simulink library "outp"  (R2021b)
(part 10 of 11)

  UnitConverter67/1 -> VOUTP_LRWhlRotDir_enum/1  "VOUTP_LRWhlRotDir_enum"
  VAPM_LRWhlRotDirTimeOut_flg/1 -> VAPM_LRWhlRotDirTimeOut_flg_Inproc/1  "VAPM_LRWhlRotDirTimeOut_flg"
  VAPM_LRWhlRotDirTimeOut_flg_Inproc/1 -> UnitConverter68/1
  UnitConverter68/1 -> VOUTP_LRWhlRotDirTimeOut_flg/1  "VOUTP_LRWhlRotDirTimeOut_flg"
  VAPM_RRWhlRotDir_enum/1 -> VAPM_RRWhlRotDir_enum_Inproc/1  "VAPM_RRWhlRotDir_enum"
  VAPM_RRWhlRotDir_enum_Inproc/1 -> UnitConverter69/1
  UnitConverter69/1 -> VOUTP_RRWhlRotDir_enum/1  "VOUTP_RRWhlRotDir_enum"
  VAPM_RRWhlRotDirTimeOut_flg/1 -> VAPM_RRWhlRotDirTimeOut_flg_Inproc/1  "VAPM_RRWhlRotDirTimeOut_flg"
  VAPM_RRWhlRotDirTimeOut_flg_Inproc/1 -> UnitConverter70/1
  UnitConverter70/1 -> VOUTP_RRWhlRotDirTimeOut_flg/1  "VOUTP_RRWhlRotDirTimeOut_flg"
  VAPM_LFPulseCountV_flg/1 -> VAPM_LFPulseCountV_flg_Inproc/1  "VAPM_LFPulseCountV_flg"
  VAPM_LFPulseCountV_flg_Inproc/1 -> UnitConverter71/1
  UnitConverter71/1 -> VOUTP_LFPulseCountV_flg/1  "VOUTP_LFPulseCountV_flg"
  VAPM_LFPulseCountVTimeOut_flg/1 -> VAPM_LFPulseCountVTimeOut_flg_Inproc/1  "VAPM_LFPulseCountVTimeOut_flg"
  VAPM_LFPulseCountVTimeOut_flg_Inproc/1 -> UnitConverter72/1
  UnitConverter72/1 -> VOUTP_LFPulseCountVTimeOut_flg/1  "VOUTP_LFPulseCountVTimeOut_flg"
  VAPM_RFPulseCountV_flg/1 -> VAPM_RFPulseCountV_flg_Inproc/1  "VAPM_RFPulseCountV_flg"
  VAPM_RFPulseCountV_flg_Inproc/1 -> UnitConverter73/1
  UnitConverter73/1 -> VOUTP_RFPulseCountV_flg/1  "VOUTP_RFPulseCountV_flg"
  VAPM_RFPulseCountVTimeOut_flg/1 -> VAPM_RFPulseCountVTimeOut_flg_Inproc/1  "VAPM_RFPulseCountVTimeOut_flg"
  VAPM_RFPulseCountVTimeOut_flg_Inproc/1 -> UnitConverter74/1
  UnitConverter74/1 -> VOUTP_RFPulseCountVTimeOut_flg/1  "VOUTP_RFPulseCountVTimeOut_flg"
  VAPM_LRPulseCountV_flg/1 -> VAPM_LRPulseCountV_flg_Inproc/1  "VAPM_LRPulseCountV_flg"
  VAPM_LRPulseCountV_flg_Inproc/1 -> UnitConverter75/1
  UnitConverter75/1 -> VOUTP_LRPulseCountV_flg/1  "VOUTP_LRPulseCountV_flg"
  VAPM_LRPulseCountVTimeOut_flg/1 -> VAPM_LRPulseCountVTimeOut_flg_Inproc/1  "VAPM_LRPulseCountVTimeOut_flg"
  VAPM_LRPulseCountVTimeOut_flg_Inproc/1 -> UnitConverter76/1
  UnitConverter76/1 -> VOUTP_LRPulseCountVTimeOut_flg/1  "VOUTP_LRPulseCountVTimeOut_flg"
  VAPM_RRPulseCountV_flg/1 -> VAPM_RRPulseCountV_flg_Inproc/1  "VAPM_RRPulseCountV_flg"
  VAPM_RRPulseCountV_flg_Inproc/1 -> UnitConverter77/1
  UnitConverter77/1 -> VOUTP_RRPulseCountV_flg/1  "VOUTP_RRPulseCountV_flg"
  VAPM_RRPulseCountVTimeOut_flg/1 -> VAPM_RRPulseCountVTimeOut_flg_Inproc/1  "VAPM_RRPulseCountVTimeOut_flg"
  VAPM_RRPulseCountVTimeOut_flg_Inproc/1 -> UnitConverter78/1
  UnitConverter78/1 -> VOUTP_RRPulseCountVTimeOut_flg/1  "VOUTP_RRPulseCountVTimeOut_flg"
  VAPM_LFPulseCount_enum/1 -> VAPM_LFPulseCount_enum_Inproc/1  "VAPM_LFPulseCount_enum"
  VAPM_LFPulseCount_enum_Inproc/1 -> UnitConverter79/1
  UnitConverter79/1 -> VOUTP_LFPulseCount_enum/1  "VOUTP_LFPulseCount_enum"
  VAPM_LFPulseCountTimeOut_flg/1 -> VAPM_LFPulseCountTimeOut_flg_Inproc/1  "VAPM_LFPulseCountTimeOut_flg"
  VAPM_LFPulseCountTimeOut_flg_Inproc/1 -> UnitConverter80/1
  UnitConverter80/1 -> VOUTP_LFPulseCountTimeOut_flg/1  "VOUTP_LFPulseCountTimeOut_flg"
  VAPM_RFPulseCount_enum/1 -> VAPM_RFPulseCount_enum_Inproc/1  "VAPM_RFPulseCount_enum"
  VAPM_RFPulseCount_enum_Inproc/1 -> UnitConverter81/1
  UnitConverter81/1 -> VOUTP_RFPulseCount_enum/1  "VOUTP_RFPulseCount_enum"
  VAPM_RFPulseCountTimeOut_flg/1 -> VAPM_RFPulseCountTimeOut_flg_Inproc/1  "VAPM_RFPulseCountTimeOut_flg"
  VAPM_RFPulseCountTimeOut_flg_Inproc/1 -> UnitConverter82/1
  UnitConverter82/1 -> VOUTP_RFPulseCountTimeOut_flg/1  "VOUTP_RFPulseCountTimeOut_flg"
  VAPM_LRPulseCount_enum/1 -> VAPM_LRPulseCount_enum_Inproc/1  "VAPM_LRPulseCount_enum"
  VAPM_LRPulseCount_enum_Inproc/1 -> UnitConverter83/1
  UnitConverter83/1 -> VOUTP_LRPulseCount_enum/1  "VOUTP_LRPulseCount_enum"
  VAPM_LRPulseCountTimeOut_flg/1 -> VAPM_LRPulseCountTimeOut_flg_Inproc/1  "VAPM_LRPulseCountTimeOut_flg"
  VAPM_LRPulseCountTimeOut_flg_Inproc/1 -> UnitConverter84/1
  UnitConverter84/1 -> VOUTP_LRPulseCountTimeOut_flg/1  "VOUTP_LRPulseCountTimeOut_flg"
  VAPM_RRPulseCount_enum/1 -> VAPM_RRPulseCount_enum_Inproc/1  "VAPM_RRPulseCount_enum"
  VAPM_RRPulseCount_enum_Inproc/1 -> UnitConverter85/1
  UnitConverter85/1 -> VOUTP_RRPulseCount_enum/1  "VOUTP_RRPulseCount_enum"
  VAPM_RRPulseCountTimeOut_flg/1 -> VAPM_RRPulseCountTimeOut_flg_Inproc/1  "VAPM_RRPulseCountTimeOut_flg"
  VAPM_RRPulseCountTimeOut_flg_Inproc/1 -> UnitConverter86/1
  UnitConverter86/1 -> VOUTP_RRPulseCountTimeOut_flg/1  "VOUTP_RRPulseCountTimeOut_flg"
  VAPM_ShifterHandleCmd_enum/1 -> VAPM_ShifterHandleCmd_enum_Inproc/1  "VAPM_ShifterHandleCmd_enum"
  VAPM_ShifterHandleCmd_enum_Inproc/1 -> UnitConverter87/1
  UnitConverter87/1 -> VOUTP_ShifterHandleCmd_enum/1  "VOUTP_ShifterHandleCmd_enum"
  VAPM_ShifterHandleCmdTimeOut_flg/1 -> VAPM_ShifterHandleCmdTimeOut_flg_Inproc/1  "VAPM_ShifterHandleCmdTimeOut_flg"
  VAPM_ShifterHandleCmdTimeOut_flg_Inproc/1 -> UnitConverter88/1
  UnitConverter88/1 -> VOUTP_ShifterHandleCmdTimeOut_flg/1  "VOUTP_ShifterHandleCmdTimeOut_flg"
  VAPM_DriIntend_enum/1 -> VAPM_DriIntend_enum_Inproc/1  "VAPM_DriIntend_enum"
  VAPM_DriIntend_enum_Inproc/1 -> UnitConverter89/1
  UnitConverter89/1 -> VOUTP_DriIntend_enum/1  "VOUTP_DriIntend_enum"
  VAPM_DriIntendTimeOut_flg/1 -> VAPM_DriIntendTimeOut_flg_Inproc/1  "VAPM_DriIntendTimeOut_flg"
  VAPM_DriIntendTimeOut_flg_Inproc/1 -> UnitConverter90/1
  UnitConverter90/1 -> VOUTP_DriIntendTimeOut_flg/1  "VOUTP_DriIntendTimeOut_flg"
  VAPM_EPSAOIControl_enum/1 -> VAPM_EPSAOIControl_enum_Inproc/1  "VAPM_EPSAOIControl_enum"
  VAPM_EPSAOIControl_enum_Inproc/1 -> UnitConverter91/1
  UnitConverter91/1 -> VOUTP_EPSAOIControl_enum/1  "VOUTP_EPSAOIControl_enum"
  VAPM_EPSAOIControlTimeOut_flg/1 -> VAPM_EPSAOIControlTimeOut_flg_Inproc/1  "VAPM_EPSAOIControlTimeOut_flg"
  VAPM_EPSAOIControlTimeOut_flg_Inproc/1 -> UnitConverter92/1
  UnitConverter92/1 -> VOUTP_EPSAOIControlTimeOut_flg/1  "VOUTP_EPSAOIControlTimeOut_flg"
  VAPM_SASAngle_Deg/1 -> VAPM_SASAngle_Deg_Inproc/1  "VAPM_SASAngle_Deg"
  VAPM_SASAngle_Deg_Inproc/1 -> UnitConverter93/1
  UnitConverter93/1 -> VOUTP_SASAngle_Deg/1  "VOUTP_SASAngle_Deg"
  VAPM_SASAngleTimeOut_flg/1 -> VAPM_SASAngleTimeOut_flg_Inproc/1  "VAPM_SASAngleTimeOut_flg"
  VAPM_SASAngleTimeOut_flg_Inproc/1 -> UnitConverter94/1
  UnitConverter94/1 -> VOUTP_SASAngleTimeOut_flg/1  "VOUTP_SASAngleTimeOut_flg"
  VAPM_SASSpeed_degps/1 -> VAPM_SASSpeed_degps_Inproc/1  "VAPM_SASSpeed_degps"
  VAPM_SASSpeed_degps_Inproc/1 -> UnitConverter95/1
  UnitConverter95/1 -> VOUTP_SASSpeed_degps/1  "VOUTP_SASSpeed_degps"
  VAPM_SASSpeedTimeOut_flg/1 -> VAPM_SASSpeedTimeOut_flg_Inproc/1  "VAPM_SASSpeedTimeOut_flg"
  VAPM_SASSpeedTimeOut_flg_Inproc/1 -> UnitConverter96/1
  UnitConverter96/1 -> VOUTP_SASSpeedTimeOut_flg/1  "VOUTP_SASSpeedTimeOut_flg"
  VAPM_SASSpeedValid_flg/1 -> VAPM_SASSpeedValid_flg_Inproc/1  "VAPM_SASSpeedValid_flg"
  VAPM_SASSpeedValid_flg_Inproc/1 -> UnitConverter97/1
  UnitConverter97/1 -> VOUTP_SASSpeedValid_flg/1  "VOUTP_SASSpeedValid_flg"
  VAPM_SASSpeedValidTimeOut_flg/1 -> VAPM_SASSpeedValidTimeOut_flg_Inproc/1  "VAPM_SASSpeedValidTimeOut_flg"
  VAPM_SASSpeedValidTimeOut_flg_Inproc/1 -> UnitConverter98/1
  UnitConverter98/1 -> VOUTP_SASSpeedValidTimeOut_flg/1  "VOUTP_SASSpeedValidTimeOut_flg"
  VAPM_SASCAL_flg/1 -> VAPM_SASCAL_flg_Inproc/1  "VAPM_SASCAL_flg"
  VAPM_SASCAL_flg_Inproc/1 -> UnitConverter99/1
  UnitConverter99/1 -> VOUTP_SASCAL_flg/1  "VOUTP_SASCAL_flg"
  VAPM_SASCALTimeOut_flg/1 -> VAPM_SASCALTimeOut_flg_Inproc/1  "VAPM_SASCALTimeOut_flg"
  VAPM_SASCALTimeOut_flg_Inproc/1 -> UnitConverter100/1
  UnitConverter100/1 -> VOUTP_SASCALTimeOut_flg/1  "VOUTP_SASCALTimeOut_flg"
  VAPM_SASV_flg/1 -> VAPM_SASV_flg_Inproc/1  "VAPM_SASV_flg"
  VAPM_SASV_flg_Inproc/1 -> UnitConverter101/1
  UnitConverter101/1 -> VOUTP_SASV_flg/1  "VOUTP_SASV_flg"
  VAPM_SASVTimeOut_flg/1 -> VAPM_SASVTimeOut_flg_Inproc/1  "VAPM_SASVTimeOut_flg"
  VAPM_SASVTimeOut_flg_Inproc/1 -> UnitConverter102/1
  UnitConverter102/1 -> VOUTP_SASVTimeOut_flg/1  "VOUTP_SASVTimeOut_flg"
  VAPM_GRADE_Deg/1 -> VAPM_GRADE_Deg_Inproc/1  "VAPM_GRADE_Deg"
  VAPM_GRADE_Deg_Inproc/1 -> UnitConverter103/1
  UnitConverter103/1 -> VOUTP_GRADE_Deg/1  "VOUTP_GRADE_Deg"
  VAPM_GRADETimeOut_flg/1 -> VAPM_GRADETimeOut_flg_Inproc/1  "VAPM_GRADETimeOut_flg"
  VAPM_GRADETimeOut_flg_Inproc/1 -> UnitConverter104/1
  UnitConverter104/1 -> VOUTP_GRADETimeOut_flg/1  "VOUTP_GRADETimeOut_flg"
  VAPM_YawRate_degps/1 -> VAPM_YawRate_degps_Inproc/1  "VAPM_YawRate_degps"
  VAPM_YawRate_degps_Inproc/1 -> UnitConverter105/1
  UnitConverter105/1 -> VOUTP_YawRate_degps/1  "VOUTP_YawRate_degps"
  VAPM_YawRateTimeOut_flg/1 -> VAPM_YawRateTimeOut_flg_Inproc/1  "VAPM_YawRateTimeOut_flg"
  VAPM_YawRateTimeOut_flg_Inproc/1 -> UnitConverter106/1
  UnitConverter106/1 -> VOUTP_YawRateTimeOut_flg/1  "VOUTP_YawRateTimeOut_flg"
  VAPM_LatAccel_Gps/1 -> VAPM_LatAccel_Gps_Inproc/1  "VAPM_LatAccel_Gps"
  VAPM_LatAccel_Gps_Inproc/1 -> UnitConverter107/1
  UnitConverter107/1 -> VOUTP_LatAccel_Gps/1  "VOUTP_LatAccel_Gps"
  VAPM_LatAccelTimeOut_flg/1 -> VAPM_LatAccelTimeOut_flg_Inproc/1  "VAPM_LatAccelTimeOut_flg"
  VAPM_LatAccelTimeOut_flg_Inproc/1 -> UnitConverter108/1
  UnitConverter108/1 -> VOUTP_LatAccelTimeOut_flg/1  "VOUTP_LatAccelTimeOut_flg"
  VAPM_LongAccel_Gps/1 -> VAPM_LongAccel_Gps_Inproc/1  "VAPM_LongAccel_Gps"
  VAPM_LongAccel_Gps_Inproc/1 -> UnitConverter109/1
  UnitConverter109/1 -> VOUTP_LongAccel_Gps/1  "VOUTP_LongAccel_Gps"
  VAPM_LongAccelTimeOut_flg/1 -> VAPM_LongAccelTimeOut_flg_Inproc/1  "VAPM_LongAccelTimeOut_flg"
  VAPM_LongAccelTimeOut_flg_Inproc/1 -> UnitConverter110/1
  UnitConverter110/1 -> VOUTP_LongAccelTimeOut_flg/1  "VOUTP_LongAccelTimeOut_flg"
  VAPM_MCPressure_bar/1 -> VAPM_MCPressure_bar_Inproc/1  "VAPM_MCPressure_bar"
  VAPM_MCPressure_bar_Inproc/1 -> UnitConverter111/1
  UnitConverter111/1 -> VOUTP_MCPressure_bar/1  "VOUTP_MCPressure_bar"
  VAPM_MCPressureTimeOut_flg/1 -> VAPM_MCPressureTimeOut_flg_Inproc/1  "VAPM_MCPressureTimeOut_flg"
  VAPM_MCPressureTimeOut_flg_Inproc/1 -> UnitConverter112/1
  UnitConverter112/1 -> VOUTP_MCPressureTimeOut_flg/1  "VOUTP_MCPressureTimeOut_flg"
  VAPM_YawRateV_flg/1 -> VAPM_YawRateV_flg_Inproc/1  "VAPM_YawRateV_flg"
  VAPM_YawRateV_flg_Inproc/1 -> UnitConverter113/1
  UnitConverter113/1 -> VOUTP_YawRateV_flg/1  "VOUTP_YawRateV_flg"
  VAPM_YawRateVTimeOut_flg/1 -> VAPM_YawRateVTimeOut_flg_Inproc/1  "VAPM_YawRateVTimeOut_flg"
  VAPM_YawRateVTimeOut_flg_Inproc/1 -> UnitConverter114/1
  UnitConverter114/1 -> VOUTP_YawRateVTimeOut_flg/1  "VOUTP_YawRateVTimeOut_flg"
  VAPM_LatAccelV_flg/1 -> VAPM_LatAccelV_flg_Inproc/1  "VAPM_LatAccelV_flg"
  VAPM_LatAccelV_flg_Inproc/1 -> UnitConverter115/1
  UnitConverter115/1 -> VOUTP_LatAccelV_flg/1  "VOUTP_LatAccelV_flg"
  VAPM_LatAccelVTimeOut_flg/1 -> VAPM_LatAccelVTimeOut_flg_Inproc/1  "VAPM_LatAccelVTimeOut_flg"
  VAPM_LatAccelVTimeOut_flg_Inproc/1 -> UnitConverter116/1
  UnitConverter116/1 -> VOUTP_LatAccelVTimeOut_flg/1  "VOUTP_LatAccelVTimeOut_flg"
  VAPM_LongAccelV_flg/1 -> VAPM_LongAccelV_flg_Inproc/1  "VAPM_LongAccelV_flg"
  VAPM_LongAccelV_flg_Inproc/1 -> UnitConverter117/1
  UnitConverter117/1 -> VOUTP_LongAccelV_flg/1  "VOUTP_LongAccelV_flg"
  VAPM_LongAccelVTimeOut_flg/1 -> VAPM_LongAccelVTimeOut_flg_Inproc/1  "VAPM_LongAccelVTimeOut_flg"
  VAPM_LongAccelVTimeOut_flg_Inproc/1 -> UnitConverter118/1
  UnitConverter118/1 -> VOUTP_LongAccelVTimeOut_flg/1  "VOUTP_LongAccelVTimeOut_flg"
  VAPM_MCPressureV_bar/1 -> VAPM_MCPressureV_bar_Inproc/1  "VAPM_MCPressureV_bar"
  VAPM_MCPressureV_bar_Inproc/1 -> UnitConverter119/1
  UnitConverter119/1 -> VOUTP_MCPressureV_bar/1  "VOUTP_MCPressureV_bar"
  VAPM_MCPressureVTimeOut_flg/1 -> VAPM_MCPressureVTimeOut_flg_Inproc/1  "VAPM_MCPressureVTimeOut_flg"
  VAPM_MCPressureVTimeOut_flg_Inproc/1 -> UnitConverter120/1
  UnitConverter120/1 -> VOUTP_MCPressureVTimeOut_flg/1  "VOUTP_MCPressureVTimeOut_flg"
  VAPM_BrkSwSta_flg/1 -> VAPM_BrkSwSta_flg_Inproc/1  "VAPM_BrkSwSta_flg"
  VAPM_BrkSwSta_flg_Inproc/1 -> UnitConverter121/1
  UnitConverter121/1 -> VOUTP_BrkSwSta_flg/1  "VOUTP_BrkSwSta_flg"
  VAPM_BrkSwStaTimeOut_flg/1 -> VAPM_BrkSwStaTimeOut_flg_Inproc/1  "VAPM_BrkSwStaTimeOut_flg"
  VAPM_BrkSwStaTimeOut_flg_Inproc/1 -> UnitConverter122/1
  UnitConverter122/1 -> VOUTP_BrkSwStaTimeOut_flg/1  "VOUTP_BrkSwStaTimeOut_flg"
  VAPM_BrkSwV_flg/1 -> VAPM_BrkSwV_flg_Inproc/1  "VAPM_BrkSwV_flg"
  VAPM_BrkSwV_flg_Inproc/1 -> UnitConverter123/1
  UnitConverter123/1 -> VOUTP_BrkSwV_flg/1  "VOUTP_BrkSwV_flg"
  VAPM_BrkSwVTimeOut_flg/1 -> VAPM_BrkSwVTimeOut_flg_Inproc/1  "VAPM_BrkSwVTimeOut_flg"
  VAPM_BrkSwVTimeOut_flg_Inproc/1 -> UnitConverter124/1
  UnitConverter124/1 -> VOUTP_BrkSwVTimeOut_flg/1  "VOUTP_BrkSwVTimeOut_flg"
  VAPM_ESCStandstill_flg/1 -> VAPM_ESCStandstill_flg_Inproc/1  "VAPM_ESCStandstill_flg"
  VAPM_ESCStandstill_flg_Inproc/1 -> UnitConverter125/1
  UnitConverter125/1 -> VOUTP_ESCStandstill_flg/1  "VOUTP_ESCStandstill_flg"
  VAPM_ESCStandstillTimeOut_flg/1 -> VAPM_ESCStandstillTimeOut_flg_Inproc/1  "VAPM_ESCStandstillTimeOut_flg"
  VAPM_ESCStandstillTimeOut_flg_Inproc/1 -> UnitConverter126/1
  UnitConverter126/1 -> VOUTP_ESCStandstillTimeOut_flg/1  "VOUTP_ESCStandstillTimeOut_flg"
  VAPM_ESCAPSSta_enum/1 -> VAPM_ESCAPSSta_enum_Inproc/1  "VAPM_ESCAPSSta_enum"
  VAPM_ESCAPSSta_enum_Inproc/1 -> UnitConverter127/1
  UnitConverter127/1 -> VOUTP_ESCAPSSta_enum/1  "VOUTP_ESCAPSSta_enum"
  VAPM_ESCAPSStaTimeOut_flg/1 -> VAPM_ESCAPSStaTimeOut_flg_Inproc/1  "VAPM_ESCAPSStaTimeOut_flg"
  VAPM_ESCAPSStaTimeOut_flg_Inproc/1 -> UnitConverter128/1
  UnitConverter128/1 -> VOUTP_ESCAPSStaTimeOut_flg/1  "VOUTP_ESCAPSStaTimeOut_flg"
  VAPM_EPBExtReleaseAvail_flg/1 -> VAPM_EPBExtReleaseAvail_flg_Inproc/1  "VAPM_EPBExtReleaseAvail_flg"
  VAPM_EPBExtReleaseAvail_flg_Inproc/1 -> UnitConverter129/1
  UnitConverter129/1 -> VOUTP_EPBExtReleaseAvail_flg/1  "VOUTP_EPBExtReleaseAvail_flg"
  VAPM_EPBExtReleaseAvailTimeOut_flg/1 -> VAPM_EPBExtReleaseAvailTimeOut_flg_Inproc/1  "VAPM_EPBExtReleaseAvailTimeOut_flg"
  VAPM_EPBExtReleaseAvailTimeOut_flg_Inproc/1 -> UnitConverter130/1
  UnitConverter130/1 -> VOUTP_EPBExtReleaseAvailTimeOut_flg/1  "VOUTP_EPBExtReleaseAvailTimeOut_flg"
  VAPM_EPBExtApplyAvail_flg/1 -> VAPM_EPBExtApplyAvail_flg_Inproc/1  "VAPM_EPBExtApplyAvail_flg"
  VAPM_EPBExtApplyAvail_flg_Inproc/1 -> UnitConverter131/1
  UnitConverter131/1 -> VOUTP_EPBExtApplyAvail_flg/1  "VOUTP_EPBExtApplyAvail_flg"
  VAPM_EPBExtApplyAvailTimeOut_flg/1 -> VAPM_EPBExtApplyAvailTimeOut_flg_Inproc/1  "VAPM_EPBExtApplyAvailTimeOut_flg"
  VAPM_EPBExtApplyAvailTimeOut_flg_Inproc/1 -> UnitConverter132/1
  UnitConverter132/1 -> VOUTP_EPBExtApplyAvailTimeOut_flg/1  "VOUTP_EPBExtApplyAvailTimeOut_flg"
  VAPM_EPBErrSta_enum/1 -> VAPM_EPBErrSta_enum_Inproc/1  "VAPM_EPBErrSta_enum"
  VAPM_EPBErrSta_enum_Inproc/1 -> UnitConverter133/1
  UnitConverter133/1 -> VOUTP_EPBErrSta_enum/1  "VOUTP_EPBErrSta_enum"
  VAPM_EPBErrStaTimeOut_flg/1 -> VAPM_EPBErrStaTimeOut_flg_Inproc/1  "VAPM_EPBErrStaTimeOut_flg"
  VAPM_EPBErrStaTimeOut_flg_Inproc/1 -> UnitConverter134/1
  UnitConverter134/1 -> VOUTP_EPBErrStaTimeOut_flg/1  "VOUTP_EPBErrStaTimeOut_flg"
  VAPM_EPBSta_enum/1 -> VAPM_EPBSta_enum_Inproc/1  "VAPM_EPBSta_enum"
  VAPM_EPBSta_enum_Inproc/1 -> UnitConverter135/1
  UnitConverter135/1 -> VOUTP_EPBSta_enum/1  "VOUTP_EPBSta_enum"
  VAPM_EPBStaTimeOut_flg/1 -> VAPM_EPBStaTimeOut_flg_Inproc/1  "VAPM_EPBStaTimeOut_flg"
  VAPM_EPBStaTimeOut_flg_Inproc/1 -> UnitConverter136/1
  UnitConverter136/1 -> VOUTP_EPBStaTimeOut_flg/1  "VOUTP_EPBStaTimeOut_flg"
  VAPM_AVMparkingcancel_enum/1 -> VAPM_AVMparkingcancel_enum_Inproc/1  "VAPM_AVMparkingcancel_enum"
  VAPM_AVMparkingcancel_enum_Inproc/1 -> UnitConverter137/1
  UnitConverter137/1 -> VOUTP_AVMparkingcancel_enum/1  "VOUTP_AVMparkingcancel_enum"
  VAPM_AVMparkingcancelTimeOut_flg/1 -> VAPM_AVMparkingcancelTimeOut_flg_Inproc/1  "VAPM_AVMparkingcancelTimeOut_flg"
  VAPM_AVMparkingcancelTimeOut_flg_Inproc/1 -> UnitConverter138/1
  UnitConverter138/1 -> VOUTP_AVMparkingcancelTimeOut_flg/1  "VOUTP_AVMparkingcancelTimeOut_flg"
  VAPM_AVMparkingexcute_enum/1 -> VAPM_AVMparkingexcute_enum_Inproc/1  "VAPM_AVMparkingexcute_enum"
  VAPM_AVMparkingexcute_enum_Inproc/1 -> UnitConverter139/1
  UnitConverter139/1 -> VOUTP_AVMparkingexcute_enum/1  "VOUTP_AVMparkingexcute_enum"
  VAPM_AVMparkingexcuteTimeOut_flg/1 -> VAPM_AVMparkingexcuteTimeOut_flg_Inproc/1  "VAPM_AVMparkingexcuteTimeOut_flg"
  VAPM_AVMparkingexcuteTimeOut_flg_Inproc/1 -> UnitConverter140/1
  UnitConverter140/1 -> VOUTP_AVMparkingexcuteTimeOut_flg/1  "VOUTP_AVMparkingexcuteTimeOut_flg"
  VAPM_AVMParkingmode_enum/1 -> VAPM_AVMParkingmode_enum_Inproc/1  "VAPM_AVMParkingmode_enum"
  VAPM_AVMParkingmode_enum_Inproc/1 -> UnitConverter141/1
  UnitConverter141/1 -> VOUTP_AVMParkingmode_enum/1  "VOUTP_AVMParkingmode_enum"
  VAPM_AVMParkingmodeTimeOut_flg/1 -> VAPM_AVMParkingmodeTimeOut_flg_Inproc/1  "VAPM_AVMParkingmodeTimeOut_flg"
  VAPM_AVMParkingmodeTimeOut_flg_Inproc/1 -> UnitConverter142/1
  UnitConverter142/1 -> VOUTP_AVMParkingmodeTimeOut_flg/1  "VOUTP_AVMParkingmodeTimeOut_flg"
  VAPM_AVMErrSTA_flg/1 -> VAPM_AVMErrSTA_flg_Inproc/1  "VAPM_AVMErrSTA_flg"
  VAPM_AVMErrSTA_flg_Inproc/1 -> UnitConverter143/1
  UnitConverter143/1 -> VOUTP_AVMErrSTA_flg/1  "VOUTP_AVMErrSTA_flg"
  VAPM_AVMErrSTATimeOut_flg/1 -> VAPM_AVMErrSTATimeOut_flg_Inproc/1  "VAPM_AVMErrSTATimeOut_flg"
  VAPM_AVMErrSTATimeOut_flg_Inproc/1 -> UnitConverter144/1
  UnitConverter144/1 -> VOUTP_AVMErrSTATimeOut_flg/1  "VOUTP_AVMErrSTATimeOut_flg"
  VAPM_IVIStatus_flg/1 -> VAPM_IVIStatus_flg_Inproc/1  "VAPM_IVIStatus_flg"
  VAPM_IVIStatus_flg_Inproc/1 -> UnitConverter145/1
  UnitConverter145/1 -> VOUTP_IVIStatus_flg/1  "VOUTP_IVIStatus_flg"
  VAPM_IVIStatusTimeOut_flg/1 -> VAPM_IVIStatusTimeOut_flg_Inproc/1  "VAPM_IVIStatusTimeOut_flg"
  VAPM_IVIStatusTimeOut_flg_Inproc/1 -> UnitConverter146/1
  UnitConverter146/1 -> VOUTP_IVIStatusTimeOut_flg/1  "VOUTP_IVIStatusTimeOut_flg"
  VAPM_CAASSw_enum/1 -> VAPM_CAASSw_enum_Inproc/1  "VAPM_CAASSw_enum"
  VAPM_CAASSw_enum_Inproc/1 -> UnitConverter147/1
  UnitConverter147/1 -> VOUTP_CAASSw_enum/1  "VOUTP_CAASSw_enum"
  VAPM_CAASSwTimeOut_flg/1 -> VAPM_CAASSwTimeOut_flg_Inproc/1  "VAPM_CAASSwTimeOut_flg"
  VAPM_CAASSwTimeOut_flg_Inproc/1 -> UnitConverter148/1
  UnitConverter148/1 -> VOUTP_CAASSwTimeOut_flg/1  "VOUTP_CAASSwTimeOut_flg"
  VAPM_IVIScreen_enum/1 -> VAPM_IVIScreen_enum_Inproc/1  "VAPM_IVIScreen_enum"
  VAPM_IVIScreen_enum_Inproc/1 -> UnitConverter149/1
  UnitConverter149/1 -> VOUTP_IVIScreen_enum/1  "VOUTP_IVIScreen_enum"
  VAPM_IVIScreenTimeOut_flg/1 -> VAPM_IVIScreenTimeOut_flg_Inproc/1  "VAPM_IVIScreenTimeOut_flg"
  VAPM_IVIScreenTimeOut_flg_Inproc/1 -> UnitConverter150/1
  UnitConverter150/1 -> VOUTP_IVIScreenTimeOut_flg/1  "VOUTP_IVIScreenTimeOut_flg"
  VAPM_ABSActive_flg/1 -> VAPM_ABSActive_flg_Inproc/1  "VAPM_ABSActive_flg"
  VAPM_ABSActive_flg_Inproc/1 -> UnitConverter151/1
  UnitConverter151/1 -> VOUTP_ABSActive_flg/1  "VOUTP_ABSActive_flg"
  VAPM_ABSActiveTimeOut_flg/1 -> VAPM_ABSActiveTimeOut_flg_Inproc/1  "VAPM_ABSActiveTimeOut_flg"
  VAPM_ABSActiveTimeOut_flg_Inproc/1 -> UnitConverter152/1
  UnitConverter152/1 -> VOUTP_ABSActiveTimeOut_flg/1  "VOUTP_ABSActiveTimeOut_flg"
  VAPM_TCSActive_flg/1 -> VAPM_TCSActive_flg_Inproc/1  "VAPM_TCSActive_flg"
  VAPM_TCSActive_flg_Inproc/1 -> UnitConverter153/1
  UnitConverter153/1 -> VOUTP_TCSActive_flg/1  "VOUTP_TCSActive_flg"
  VAPM_TCSActiveTimeOut_flg/1 -> VAPM_TCSActiveTimeOut_flg_Inproc/1  "VAPM_TCSActiveTimeOut_flg"
  VAPM_TCSActiveTimeOut_flg_Inproc/1 -> UnitConverter154/1
  UnitConverter154/1 -> VOUTP_TCSActiveTimeOut_flg/1  "VOUTP_TCSActiveTimeOut_flg"
  VAPM_DriverSeatBeltCmd_flg/1 -> VAPM_DriverSeatBeltCmd_flg_Inproc/1  "VAPM_DriverSeatBeltCmd_flg"
  VAPM_DriverSeatBeltCmd_flg_Inproc/1 -> UnitConverter155/1
  UnitConverter155/1 -> VOUTP_DriverSeatBeltCmd_flg/1  "VOUTP_DriverSeatBeltCmd_flg"
  VAPM_DriverSeatBeltCmdTimeOut_flg/1 -> VAPM_DriverSeatBeltCmdTimeOut_flg_Inproc/1  "VAPM_DriverSeatBeltCmdTimeOut_flg"
  VAPM_DriverSeatBeltCmdTimeOut_flg_Inproc/1 -> UnitConverter156/1
  UnitConverter156/1 -> VOUTP_DriverSeatBeltCmdTimeOut_flg/1  "VOUTP_DriverSeatBeltCmdTimeOut_flg"
  VAPM_APSProgressPCT_pct/1 -> VAPM_APSProgressPCT_pct_Inproc/1  "VAPM_APSProgressPCT_pct"
  VAPM_APSProgressPCT_pct_Inproc/1 -> UnitConverter157/1
  UnitConverter157/1 -> VOUTP_APSProgressPCT_pct/1  "VOUTP_APSProgressPCT_pct"
  VAPM_APSRQDisplay_enum/1 -> VAPM_APSRQDisplay_enum_Inproc/1  "VAPM_APSRQDisplay_enum"
  VAPM_APSRQDisplay_enum_Inproc/1 -> UnitConverter158/1
  UnitConverter158/1 -> VOUTP_APSRQDisplay_enum/1  "VOUTP_APSRQDisplay_enum"
  VAPM_APSSWVer_enum/1 -> VAPM_APSSWVer_enum_Inproc/1  "VAPM_APSSWVer_enum"
  VAPM_APSSWVer_enum_Inproc/1 -> UnitConverter159/1
  UnitConverter159/1 -> VOUTP_APSSWVer_enum/1  "VOUTP_APSSWVer_enum"
  VAPM_APSHWVer_enum/1 -> VAPM_APSHWVer_enum_Inproc/1  "VAPM_APSHWVer_enum"
  VAPM_APSHWVer_enum_Inproc/1 -> UnitConverter160/1
  UnitConverter160/1 -> VOUTP_APSHWVer_enum/1  "VOUTP_APSHWVer_enum"
  VAPM_APSExitCondition_enum/1 -> VAPM_APSExitCondition_enum_Inproc/1  "VAPM_APSExitCondition_enum"
  VAPM_APSExitCondition_enum_Inproc/1 -> UnitConverter161/1
  UnitConverter161/1 -> VOUTP_APSExitCondition_enum/1  "VOUTP_APSExitCondition_enum"
  VAPM_APSAngleTarget_Deg/1 -> VAPM_APSAngleTarget_Deg_Inproc/1  "VAPM_APSAngleTarget_Deg"
  VAPM_APSAngleTarget_Deg_Inproc/1 -> UnitConverter162/1
  UnitConverter162/1 -> VOUTP_APSAngleTarget_Deg/1  "VOUTP_APSAngleTarget_Deg"
  VAPM_APSVRqEPASCtrl_flg/1 -> VAPM_APSVRqEPASCtrl_flg_Inproc/1  "VAPM_APSVRqEPASCtrl_flg"
  VAPM_APSVRqEPASCtrl_flg_Inproc/1 -> UnitConverter163/1
  UnitConverter163/1 -> VOUTP_APSVRqEPASCtrl_flg/1  "VOUTP_APSVRqEPASCtrl_flg"
  VAPM_APSRqEPASCtrl_flg/1 -> VAPM_APSRqEPASCtrl_flg_Inproc/1  "VAPM_APSRqEPASCtrl_flg"
  VAPM_APSRqEPASCtrl_flg_Inproc/1 -> UnitConverter164/1
  UnitConverter164/1 -> VOUTP_APSRqEPASCtrl_flg/1  "VOUTP_APSRqEPASCtrl_flg"
  VAPM_CAASSta_enum/1 -> VAPM_CAASSta_enum_Inproc/1  "VAPM_CAASSta_enum"
  VAPM_CAASSta_enum_Inproc/1 -> UnitConverter165/1
  UnitConverter165/1 -> VOUTP_CAASSta_enum/1  "VOUTP_CAASSta_enum"
  VAPM_DKCPDkeyAreaRAPSSta_enum/1 -> VAPM_DKCPDkeyAreaRAPSSta_enum_Inproc/1  "VAPM_DKCPDkeyAreaRAPSSta_enum"
  VAPM_DKCPDkeyAreaRAPSSta_enum_Inproc/1 -> UnitConverter166/1
  UnitConverter166/1 -> VOUTP_DKCPDkeyAreaRAPSSta_enum/1  "VOUTP_DKCPDkeyAreaRAPSSta_enum"
  VAPM_DKCParkingModeCmd_enum/1 -> VAPM_DKCParkingModeCmd_enum_Inproc/1  "VAPM_DKCParkingModeCmd_enum"
  VAPM_DKCParkingModeCmd_enum_Inproc/1 -> UnitConverter167/1
  UnitConverter167/1 -> VOUTP_DKCParkingModeCmd_enum/1  "VOUTP_DKCParkingModeCmd_enum"
  VAPM_PUIDLowPower_flg/1 -> VAPM_PUIDLowPower_flg_Inproc/1  "VAPM_PUIDLowPower_flg"
  VAPM_PUIDLowPower_flg_Inproc/1 -> UnitConverter168/1
  UnitConverter168/1 -> VOUTP_PUIDLowPower_flg/1  "VOUTP_PUIDLowPower_flg"
  VAPM_CAASVMCReqA_flg/1 -> VAPM_CAASVMCReqA_flg_Inproc/1  "VAPM_CAASVMCReqA_flg"
  VAPM_CAASVMCReqA_flg_Inproc/1 -> UnitConverter169/1
  UnitConverter169/1 -> VOUTP_CAASVMCReqA_flg/1  "VOUTP_CAASVMCReqA_flg"
  VAPM_APSShiftPosnReq_enum/1 -> VAPM_APSShiftPosnReq_enum_Inproc/1  "VAPM_APSShiftPosnReq_enum"
  VAPM_APSShiftPosnReq_enum_Inproc/1 -> UnitConverter170/1
  UnitConverter170/1 -> VOUTP_APSShiftPosnReq_enum/1  "VOUTP_APSShiftPosnReq_enum"
  VAPM_APSSpeedCMD_kph/1 -> VAPM_APSSpeedCMD_kph_Inproc/1  "VAPM_APSSpeedCMD_kph"
  VAPM_APSSpeedCMD_kph_Inproc/1 -> UnitConverter171/1
  UnitConverter171/1 -> VOUTP_APSSpeedCMD_kph/1  "VOUTP_APSSpeedCMD_kph"
  VAPM_APSVMCReqA_flg/1 -> VAPM_APSVMCReqA_flg_Inproc/1  "VAPM_APSVMCReqA_flg"
  VAPM_APSVMCReqA_flg_Inproc/1 -> UnitConverter172/1
  UnitConverter172/1 -> VOUTP_APSVMCReqA_flg/1  "VOUTP_APSVMCReqA_flg"
  VAPM_RAPSBCMLamp_enum/1 -> VAPM_RAPSBCMLamp_enum_Inproc/1  "VAPM_RAPSBCMLamp_enum"
  VAPM_RAPSBCMLamp_enum_Inproc/1 -> UnitConverter173/1
  UnitConverter173/1 -> VOUTP_RAPSBCMLamp_enum/1  "VOUTP_RAPSBCMLamp_enum"
  VAPM_RAPSBCMLockReq_flg/1 -> VAPM_RAPSBCMLockReq_flg_Inproc/1  "VAPM_RAPSBCMLockReq_flg"
  VAPM_RAPSBCMLockReq_flg_Inproc/1 -> UnitConverter174/1
  UnitConverter174/1 -> VOUTP_RAPSBCMLockReq_flg/1  "VOUTP_RAPSBCMLockReq_flg"
  VAPM_APSPwrReq_enum/1 -> VAPM_APSPwrReq_enum_Inproc/1  "VAPM_APSPwrReq_enum"
  VAPM_APSPwrReq_enum_Inproc/1 -> UnitConverter175/1
  UnitConverter175/1 -> VOUTP_APSPwrReq_enum/1  "VOUTP_APSPwrReq_enum"
  VAPM_RAPSErrWarnSta_enum/1 -> VAPM_RAPSErrWarnSta_enum_Inproc/1  "VAPM_RAPSErrWarnSta_enum"
  VAPM_RAPSErrWarnSta_enum_Inproc/1 -> UnitConverter176/1
  UnitConverter176/1 -> VOUTP_RAPSErrWarnSta_enum/1  "VOUTP_RAPSErrWarnSta_enum"
  VAPM_RAPSErrLv1_flg/1 -> VAPM_RAPSErrLv1_flg_Inproc/1  "VAPM_RAPSErrLv1_flg"
  VAPM_RAPSErrLv1_flg_Inproc/1 -> UnitConverter177/1
  UnitConverter177/1 -> VOUTP_RAPSErrLv1_flg/1  "VOUTP_RAPSErrLv1_flg"
  VAPM_IVIUserTakeOverAPSSta_flg/1 -> VAPM_IVIUserTakeOverAPSSta_flg_Inproc/1  "VAPM_IVIUserTakeOverAPSSta_flg"
  VAPM_IVIUserTakeOverAPSSta_flg_Inproc/1 -> UnitConverter178/1
  UnitConverter178/1 -> VOUTP_IVIUserTakeOverAPSSta_flg/1  "VOUTP_IVIUserTakeOverAPSSta_flg"
  VBCM_AntitheftSta_enum/1 -> VBCM_AntitheftSta_enum_Inproc/1  "VBCM_AntitheftSta_enum"
  VBCM_AntitheftSta_enum_Inproc/1 -> UnitConverter179/1
  UnitConverter179/1 -> VOUTP_AntitheftSta_enum/1  "VOUTP_AntitheftSta_enum"
  VBCM_TailgateRemote_enum/1 -> VBCM_TailgateRemote_enum_Inproc/1  "VBCM_TailgateRemote_enum"
  VBCM_TailgateRemote_enum_Inproc/1 -> UnitConverter180/1
  UnitConverter180/1 -> VOUTP_TailgateRemote_enum/1  "VOUTP_TailgateRemote_enum"
  VBCM_HornCtrl_flg/1 -> VBCM_HornCtrl_flg_Inproc/1  "VBCM_HornCtrl_flg"
  VBCM_HornCtrl_flg_Inproc/1 -> UnitConverter181/1
  UnitConverter181/1 -> VOUTP_HornCtrl_flg/1  "VOUTP_HornCtrl_flg"
  VBCM_AllDoorSW_flg/1 -> VBCM_AllDoorSW_flg_Inproc/1  "VBCM_AllDoorSW_flg"
  VBCM_AllDoorSW_flg_Inproc/1 -> UnitConverter182/1
  UnitConverter182/1 -> VOUTP_AllDoorSW_flg/1  "VOUTP_AllDoorSW_flg"
  VBCM_BCMDoorLockSta_flg/1 -> VBCM_BCMDoorLockSta_flg_Inproc/1  "VBCM_BCMDoorLockSta_flg"
  VBCM_BCMDoorLockSta_flg_Inproc/1 -> UnitConverter183/1
  UnitConverter183/1 -> VOUTP_BCMDoorLockSta_flg/1  "VOUTP_BCMDoorLockSta_flg"
  VBCM_AntitheftSeatFlod_flg/1 -> VBCM_AntitheftSeatFlod_flg_Inproc/1  "VBCM_AntitheftSeatFlod_flg"
  VBCM_AntitheftSeatFlod_flg_Inproc/1 -> UnitConverter184/1
  UnitConverter184/1 -> VOUTP_AntitheftSeatFlod_flg/1  "VOUTP_AntitheftSeatFlod_flg"
  VBCM_HoodSW_flg/1 -> VBCM_HoodSW_flg_Inproc/1  "VBCM_HoodSW_flg"
  VBCM_HoodSW_flg_Inproc/1 -> UnitConverter185/1
  UnitConverter185/1 -> VOUTP_HoodSW_flg/1  "VOUTP_HoodSW_flg"
  VBCM_TailgateSW_flg/1 -> VBCM_TailgateSW_flg_Inproc/1  "VBCM_TailgateSW_flg"
  VBCM_TailgateSW_flg_Inproc/1 -> UnitConverter186/1
  UnitConverter186/1 -> VOUTP_TailgateSW_flg/1  "VOUTP_TailgateSW_flg"
  VBCM_DrDoorSW_flg/1 -> VBCM_DrDoorSW_flg_Inproc/1  "VBCM_DrDoorSW_flg"
  VBCM_DrDoorSW_flg_Inproc/1 -> UnitConverter187/1
  UnitConverter187/1 -> VOUTP_DrDoorSW_flg/1  "VOUTP_DrDoorSW_flg"
  VBCM_PsDoorSW_flg/1 -> VBCM_PsDoorSW_flg_Inproc/1  "VBCM_PsDoorSW_flg"
  VBCM_PsDoorSW_flg_Inproc/1 -> UnitConverter188/1
  UnitConverter188/1 -> VOUTP_PsDoorSW_flg/1  "VOUTP_PsDoorSW_flg"
  VBCM_RLDoorSW_flg/1 -> VBCM_RLDoorSW_flg_Inproc/1  "VBCM_RLDoorSW_flg"
  VBCM_RLDoorSW_flg_Inproc/1 -> UnitConverter189/1
  UnitConverter189/1 -> VOUTP_RLDoorSW_flg/1  "VOUTP_RLDoorSW_flg"
  VBCM_RRDoorSW_flg/1 -> VBCM_RRDoorSW_flg_Inproc/1  "VBCM_RRDoorSW_flg"
  VBCM_RRDoorSW_flg_Inproc/1 -> UnitConverter190/1
  UnitConverter190/1 -> VOUTP_RRDoorSW_flg/1  "VOUTP_RRDoorSW_flg"
  VBCM_LockSetting_flg/1 -> VBCM_LockSetting_flg_Inproc/1  "VBCM_LockSetting_flg"
  VBCM_LockSetting_flg_Inproc/1 -> UnitConverter191/1
  UnitConverter191/1 -> VOUTP_LockSetting_flg/1  "VOUTP_LockSetting_flg"
  VBCM_FrChargingDoorCtrl_enum/1 -> VBCM_FrChargingDoorCtrl_enum_Inproc/1  "VBCM_FrChargingDoorCtrl_enum"
  VBCM_FrChargingDoorCtrl_enum_Inproc/1 -> UnitConverter192/1
  UnitConverter192/1 -> VOUTP_FrChargingDoorCtrl_enum/1  "VOUTP_FrChargingDoorCtrl_enum"
  VBCM_RrChargingDoorCtrl_enum/1 -> VBCM_RrChargingDoorCtrl_enum_Inproc/1  "VBCM_RrChargingDoorCtrl_enum"
  VBCM_RrChargingDoorCtrl_enum_Inproc/1 -> UnitConverter193/1
  UnitConverter193/1 -> VOUTP_RrChargingDoorCtrl_enum/1  "VOUTP_RrChargingDoorCtrl_enum"
  VBCM_CrashDetd_flg/1 -> VBCM_CrashDetd_flg_Inproc/1  "VBCM_CrashDetd_flg"
  VBCM_CrashDetd_flg_Inproc/1 -> UnitConverter194/1
  UnitConverter194/1 -> VOUTP_CrashDetd_flg/1  "VOUTP_CrashDetd_flg"
  VBCM_CTDCtrl_enum/1 -> VBCM_CTDCtrl_enum_Inproc/1  "VBCM_CTDCtrl_enum"
  VBCM_CTDCtrl_enum_Inproc/1 -> UnitConverter195/1
  UnitConverter195/1 -> VOUTP_CTDCtrl_enum/1  "VOUTP_CTDCtrl_enum"
  VBCM_DoorLockIND_flg/1 -> VBCM_DoorLockIND_flg_Inproc/1  "VBCM_DoorLockIND_flg"
  VBCM_DoorLockIND_flg_Inproc/1 -> UnitConverter196/1
  UnitConverter196/1 -> VOUTP_DoorLockIND_flg/1  "VOUTP_DoorLockIND_flg"
  VBCM_CTDLockSW_flg/1 -> VBCM_CTDLockSW_flg_Inproc/1  "VBCM_CTDLockSW_flg"
  VBCM_CTDLockSW_flg_Inproc/1 -> UnitConverter197/1
  UnitConverter197/1 -> VOUTP_CTDLockSW_flg/1  "VOUTP_CTDLockSW_flg"
  VBCM_Dimmer_pct/1 -> VBCM_Dimmer_pct_Inproc/1  "VBCM_Dimmer_pct"
  VBCM_Dimmer_pct_Inproc/1 -> UnitConverter198/1
  UnitConverter198/1 -> VOUTP_Dimmer_pct/1  "VOUTP_Dimmer_pct"
  VBCM_DimmerEN_flg/1 -> VBCM_DimmerEN_flg_Inproc/1  "VBCM_DimmerEN_flg"
  VBCM_DimmerEN_flg_Inproc/1 -> UnitConverter199/1
  UnitConverter199/1 -> VOUTP_DimmerEN_flg/1  "VOUTP_DimmerEN_flg"
  VBCM_PosLamp_flg/1 -> VBCM_PosLamp_flg_Inproc/1  "VBCM_PosLamp_flg"
  VBCM_PosLamp_flg_Inproc/1 -> UnitConverter200/1
  UnitConverter200/1 -> VOUTP_PosLamp_flg/1  "VOUTP_PosLamp_flg"
  VBCM_LBeam_flg/1 -> VBCM_LBeam_flg_Inproc/1  "VBCM_LBeam_flg"
  VBCM_LBeam_flg_Inproc/1 -> UnitConverter201/1
  UnitConverter201/1 -> VOUTP_LBeam_flg/1  "VOUTP_LBeam_flg"
  VBCM_HBeam_flg/1 -> VBCM_HBeam_flg_Inproc/1  "VBCM_HBeam_flg"
  VBCM_HBeam_flg_Inproc/1 -> UnitConverter202/1
  UnitConverter202/1 -> VOUTP_HBeam_flg/1  "VOUTP_HBeam_flg"
  VBCM_RrFogLamp_flg/1 -> VBCM_RrFogLamp_flg_Inproc/1  "VBCM_RrFogLamp_flg"
  VBCM_RrFogLamp_flg_Inproc/1 -> UnitConverter203/1
  UnitConverter203/1 -> VOUTP_RrFogLamp_flg/1  "VOUTP_RrFogLamp_flg"
  VBCM_BrakeLamp_flg/1 -> VBCM_BrakeLamp_flg_Inproc/1  "VBCM_BrakeLamp_flg"
  VBCM_BrakeLamp_flg_Inproc/1 -> UnitConverter204/1
  UnitConverter204/1 -> VOUTP_BrakeLamp_flg/1  "VOUTP_BrakeLamp_flg"
  VBCM_ReverseLamp_flg/1 -> VBCM_ReverseLamp_flg_Inproc/1  "VBCM_ReverseLamp_flg"
  VBCM_ReverseLamp_flg_Inproc/1 -> UnitConverter205/1
  UnitConverter205/1 -> VOUTP_ReverseLamp_flg/1  "VOUTP_ReverseLamp_flg"
  VBCM_LDRL_flg/1 -> VBCM_LDRL_flg_Inproc/1  "VBCM_LDRL_flg"
  VBCM_LDRL_flg_Inproc/1 -> UnitConverter206/1
  UnitConverter206/1 -> VOUTP_LDRL_flg/1  "VOUTP_LDRL_flg"
  VBCM_RDRL_flg/1 -> VBCM_RDRL_flg_Inproc/1  "VBCM_RDRL_flg"
  VBCM_RDRL_flg_Inproc/1 -> UnitConverter207/1
  UnitConverter207/1 -> VOUTP_RDRL_flg/1  "VOUTP_RDRL_flg"
  VBCM_LBSD_flg/1 -> VBCM_LBSD_flg_Inproc/1  "VBCM_LBSD_flg"
  VBCM_LBSD_flg_Inproc/1 -> UnitConverter208/1
  UnitConverter208/1 -> VOUTP_LBSD_flg/1  "VOUTP_LBSD_flg"
  VBCM_RBSD_flg/1 -> VBCM_RBSD_flg_Inproc/1  "VBCM_RBSD_flg"
  VBCM_RBSD_flg_Inproc/1 -> UnitConverter209/1
  UnitConverter209/1 -> VOUTP_RBSD_flg/1  "VOUTP_RBSD_flg"
  VBCM_HazardSW_flg/1 -> VBCM_HazardSW_flg_Inproc/1  "VBCM_HazardSW_flg"
  VBCM_HazardSW_flg_Inproc/1 -> UnitConverter210/1
  UnitConverter210/1 -> VOUTP_HazardSW_flg/1  "VOUTP_HazardSW_flg"
  VBCM_LTurnLP_flg/1 -> VBCM_LTurnLP_flg_Inproc/1  "VBCM_LTurnLP_flg"
  VBCM_LTurnLP_flg_Inproc/1 -> UnitConverter211/1
  UnitConverter211/1 -> VOUTP_LTurnLP_flg/1  "VOUTP_LTurnLP_flg"
  VBCM_RTurnLP_flg/1 -> VBCM_RTurnLP_flg_Inproc/1  "VBCM_RTurnLP_flg"
  VBCM_RTurnLP_flg_Inproc/1 -> UnitConverter212/1
  UnitConverter212/1 -> VOUTP_RTurnLP_flg/1  "VOUTP_RTurnLP_flg"
  VBCM_BCMBuzzerReq_flg/1 -> VBCM_BCMBuzzerReq_flg_Inproc/1  "VBCM_BCMBuzzerReq_flg"
  VBCM_BCMBuzzerReq_flg_Inproc/1 -> UnitConverter213/1
  UnitConverter213/1 -> VOUTP_BCMBuzzerReq_flg/1  "VOUTP_BCMBuzzerReq_flg"
  VBCM_MirrorCtrl_enum/1 -> VBCM_MirrorCtrl_enum_Inproc/1  "VBCM_MirrorCtrl_enum"
  VBCM_MirrorCtrl_enum_Inproc/1 -> UnitConverter214/1
  UnitConverter214/1 -> VOUTP_MirrorCtrl_enum/1  "VOUTP_MirrorCtrl_enum"
  VBCM_MirrorDefog_flg/1 -> VBCM_MirrorDefog_flg_Inproc/1  "VBCM_MirrorDefog_flg"
  VBCM_MirrorDefog_flg_Inproc/1 -> UnitConverter215/1
  UnitConverter215/1 -> VOUTP_MirrorDefog_flg/1  "VOUTP_MirrorDefog_flg"
  VBCM_RrDefog_flg/1 -> VBCM_RrDefog_flg_Inproc/1  "VBCM_RrDefog_flg"
  VBCM_RrDefog_flg_Inproc/1 -> UnitConverter216/1
  UnitConverter216/1 -> VOUTP_RrDefog_flg/1  "VOUTP_RrDefog_flg"
  VBCM_RoomLampH_flg/1 -> VBCM_RoomLampH_flg_Inproc/1  "VBCM_RoomLampH_flg"
  VBCM_RoomLampH_flg_Inproc/1 -> UnitConverter217/1
  UnitConverter217/1 -> VOUTP_RoomLampH_flg/1  "VOUTP_RoomLampH_flg"
  VBCM_RoomLampL_flg/1 -> VBCM_RoomLampL_flg_Inproc/1  "VBCM_RoomLampL_flg"
  VBCM_RoomLampL_flg_Inproc/1 -> UnitConverter218/1
  UnitConverter218/1 -> VOUTP_RoomLampL_flg/1  "VOUTP_RoomLampL_flg"
  VBCM_TrunkRel_flg/1 -> VBCM_TrunkRel_flg_Inproc/1  "VBCM_TrunkRel_flg"
  VBCM_TrunkRel_flg_Inproc/1 -> UnitConverter219/1
  UnitConverter219/1 -> VOUTP_TrunkRel_flg/1  "VOUTP_TrunkRel_flg"
  VBCM_TailgateHDSW_flg/1 -> VBCM_TailgateHDSW_flg_Inproc/1  "VBCM_TailgateHDSW_flg"
  VBCM_TailgateHDSW_flg_Inproc/1 -> UnitConverter220/1
  UnitConverter220/1 -> VOUTP_TailgateHDSW_flg/1  "VOUTP_TailgateHDSW_flg"
  VBCM_FrWiperL_flg/1 -> VBCM_FrWiperL_flg_Inproc/1  "VBCM_FrWiperL_flg"
  VBCM_FrWiperL_flg_Inproc/1 -> UnitConverter221/1
  UnitConverter221/1 -> VOUTP_FrWiperL_flg/1  "VOUTP_FrWiperL_flg"
  VBCM_FrWiperH_flg/1 -> VBCM_FrWiperH_flg_Inproc/1  "VBCM_FrWiperH_flg"
  VBCM_FrWiperH_flg_Inproc/1 -> UnitConverter222/1
  UnitConverter222/1 -> VOUTP_FrWiperH_flg/1  "VOUTP_FrWiperH_flg"
  VBCM_RrWiper_flg/1 -> VBCM_RrWiper_flg_Inproc/1  "VBCM_RrWiper_flg"
  VBCM_RrWiper_flg_Inproc/1 -> UnitConverter223/1
  UnitConverter223/1 -> VOUTP_RrWiper_flg/1  "VOUTP_RrWiper_flg"
  VBCM_WasherCtrl_enum/1 -> VBCM_WasherCtrl_enum_Inproc/1  "VBCM_WasherCtrl_enum"
  VBCM_WasherCtrl_enum_Inproc/1 -> UnitConverter224/1
  UnitConverter224/1 -> VOUTP_WasherCtrl_enum/1  "VOUTP_WasherCtrl_enum"
  VBCM_WiperFixMode_flg/1 -> VBCM_WiperFixMode_flg_Inproc/1  "VBCM_WiperFixMode_flg"
  VBCM_WiperFixMode_flg_Inproc/1 -> UnitConverter225/1
  UnitConverter225/1 -> VOUTP_WiperFixMode_flg/1  "VOUTP_WiperFixMode_flg"
  VBCM_AmbLightBreath1_enum/1 -> VBCM_AmbLightBreath1_enum_Inproc/1  "VBCM_AmbLightBreath1_enum"
  VBCM_AmbLightBreath1_enum_Inproc/1 -> UnitConverter226/1
  UnitConverter226/1 -> VOUTP_AmbLightBreath1_enum/1  "VOUTP_AmbLightBreath1_enum"
  VBCM_AmbLightBreath2_enum/1 -> VBCM_AmbLightBreath2_enum_Inproc/1  "VBCM_AmbLightBreath2_enum"
  VBCM_AmbLightBreath2_enum_Inproc/1 -> UnitConverter227/1
  UnitConverter227/1 -> VOUTP_AmbLightBreath2_enum/1  "VOUTP_AmbLightBreath2_enum"
  VBCM_AmbLightBreath3_enum/1 -> VBCM_AmbLightBreath3_enum_Inproc/1  "VBCM_AmbLightBreath3_enum"
  VBCM_AmbLightBreath3_enum_Inproc/1 -> UnitConverter228/1
  UnitConverter228/1 -> VOUTP_AmbLightBreath3_enum/1  "VOUTP_AmbLightBreath3_enum"
  VBCM_AmbLightBreath4_enum/1 -> VBCM_AmbLightBreath4_enum_Inproc/1  "VBCM_AmbLightBreath4_enum"
  VBCM_AmbLightBreath4_enum_Inproc/1 -> UnitConverter229/1
  UnitConverter229/1 -> VOUTP_AmbLightBreath4_enum/1  "VOUTP_AmbLightBreath4_enum"
  VBCM_AmbLightBreath5_enum/1 -> VBCM_AmbLightBreath5_enum_Inproc/1  "VBCM_AmbLightBreath5_enum"
  VBCM_AmbLightBreath5_enum_Inproc/1 -> UnitConverter230/1
  UnitConverter230/1 -> VOUTP_AmbLightBreath5_enum/1  "VOUTP_AmbLightBreath5_enum"
  VBCM_AmbLightBreath6_enum/1 -> VBCM_AmbLightBreath6_enum_Inproc/1  "VBCM_AmbLightBreath6_enum"
  VBCM_AmbLightBreath6_enum_Inproc/1 -> UnitConverter231/1
  UnitConverter231/1 -> VOUTP_AmbLightBreath6_enum/1  "VOUTP_AmbLightBreath6_enum"
  VBCM_AmbLightBrightness1_enum/1 -> VBCM_AmbLightBrightness1_enum_Inproc/1  "VBCM_AmbLightBrightness1_enum"
  VBCM_AmbLightBrightness1_enum_Inproc/1 -> UnitConverter232/1
  UnitConverter232/1 -> VOUTP_AmbLightBrightness1_enum/1  "VOUTP_AmbLightBrightness1_enum"
  VBCM_AmbLightBrightness2_enum/1 -> VBCM_AmbLightBrightness2_enum_Inproc/1  "VBCM_AmbLightBrightness2_enum"
  VBCM_AmbLightBrightness2_enum_Inproc/1 -> UnitConverter233/1
  UnitConverter233/1 -> VOUTP_AmbLightBrightness2_enum/1  "VOUTP_AmbLightBrightness2_enum"
  VBCM_AmbLightBrightness3_enum/1 -> VBCM_AmbLightBrightness3_enum_Inproc/1  "VBCM_AmbLightBrightness3_enum"
  VBCM_AmbLightBrightness3_enum_Inproc/1 -> UnitConverter234/1
  UnitConverter234/1 -> VOUTP_AmbLightBrightness3_enum/1  "VOUTP_AmbLightBrightness3_enum"
  VBCM_AmbLightBrightness4_enum/1 -> VBCM_AmbLightBrightness4_enum_Inproc/1  "VBCM_AmbLightBrightness4_enum"
  VBCM_AmbLightBrightness4_enum_Inproc/1 -> UnitConverter235/1
  UnitConverter235/1 -> VOUTP_AmbLightBrightness4_enum/1  "VOUTP_AmbLightBrightness4_enum"
  VBCM_AmbLightBrightness5_enum/1 -> VBCM_AmbLightBrightness5_enum_Inproc/1  "VBCM_AmbLightBrightness5_enum"
  VBCM_AmbLightBrightness5_enum_Inproc/1 -> UnitConverter236/1
  UnitConverter236/1 -> VOUTP_AmbLightBrightness5_enum/1  "VOUTP_AmbLightBrightness5_enum"
  VBCM_AmbLightBrightness6_enum/1 -> VBCM_AmbLightBrightness6_enum_Inproc/1  "VBCM_AmbLightBrightness6_enum"
  VBCM_AmbLightBrightness6_enum_Inproc/1 -> UnitConverter237/1
  UnitConverter237/1 -> VOUTP_AmbLightBrightness6_enum/1  "VOUTP_AmbLightBrightness6_enum"
  VBCM_AmbLightColor1_enum/1 -> VBCM_AmbLightColor1_enum_Inproc/1  "VBCM_AmbLightColor1_enum"
  VBCM_AmbLightColor1_enum_Inproc/1 -> UnitConverter238/1
  UnitConverter238/1 -> VOUTP_AmbLightColor1_enum/1  "VOUTP_AmbLightColor1_enum"
  VBCM_AmbLightColor2_enum/1 -> VBCM_AmbLightColor2_enum_Inproc/1  "VBCM_AmbLightColor2_enum"
  VBCM_AmbLightColor2_enum_Inproc/1 -> UnitConverter239/1
  UnitConverter239/1 -> VOUTP_AmbLightColor2_enum/1  "VOUTP_AmbLightColor2_enum"
  VBCM_AmbLightColor3_enum/1 -> VBCM_AmbLightColor3_enum_Inproc/1  "VBCM_AmbLightColor3_enum"
  VBCM_AmbLightColor3_enum_Inproc/1 -> UnitConverter240/1
  UnitConverter240/1 -> VOUTP_AmbLightColor3_enum/1  "VOUTP_AmbLightColor3_enum"
  VBCM_AmbLightColor4_enum/1 -> VBCM_AmbLightColor4_enum_Inproc/1  "VBCM_AmbLightColor4_enum"
  VBCM_AmbLightColor4_enum_Inproc/1 -> UnitConverter241/1
  UnitConverter241/1 -> VOUTP_AmbLightColor4_enum/1  "VOUTP_AmbLightColor4_enum"
  VBCM_AmbLightColor5_enum/1 -> VBCM_AmbLightColor5_enum_Inproc/1  "VBCM_AmbLightColor5_enum"
  VBCM_AmbLightColor5_enum_Inproc/1 -> UnitConverter242/1
  UnitConverter242/1 -> VOUTP_AmbLightColor5_enum/1  "VOUTP_AmbLightColor5_enum"
  VBCM_AmbLightColor6_enum/1 -> VBCM_AmbLightColor6_enum_Inproc/1  "VBCM_AmbLightColor6_enum"
  VBCM_AmbLightColor6_enum_Inproc/1 -> UnitConverter243/1
  UnitConverter243/1 -> VOUTP_AmbLightColor6_enum/1  "VOUTP_AmbLightColor6_enum"
  VBCM_LampPwr_flg/1 -> VBCM_LampPwr_flg_Inproc/1  "VBCM_LampPwr_flg"
  VBCM_LampPwr_flg_Inproc/1 -> UnitConverter244/1
  UnitConverter244/1 -> VOUTP_LampPwr_flg/1  "VOUTP_LampPwr_flg"
  VBCM_SPTGDet_flg/1 -> VBCM_SPTGDet_flg_Inproc/1  "VBCM_SPTGDet_flg"
  VBCM_SPTGDet_flg_Inproc/1 -> UnitConverter245/1
  UnitConverter245/1 -> VOUTP_SPTGDet_flg/1  "VOUTP_SPTGDet_flg"
  VBCM_APSOpenPTG_flg/1 -> VBCM_APSOpenPTG_flg_Inproc/1  "VBCM_APSOpenPTG_flg"
  VBCM_APSOpenPTG_flg_Inproc/1 -> UnitConverter246/1
  UnitConverter246/1 -> VOUTP_APSOpenPTG_flg/1  "VOUTP_APSOpenPTG_flg"
  VBCM_FollowMe_flg/1 -> VBCM_FollowMe_flg_Inproc/1  "VBCM_FollowMe_flg"
  VBCM_FollowMe_flg_Inproc/1 -> UnitConverter247/1
  UnitConverter247/1 -> VOUTP_FollowMe_flg/1  "VOUTP_FollowMe_flg"
  VBCM_IVIRST_flg/1 -> VBCM_IVIRST_flg_Inproc/1  "VBCM_IVIRST_flg"
  VBCM_IVIRST_flg_Inproc/1 -> UnitConverter248/1
  UnitConverter248/1 -> VOUTP_IVIRST_flg/1  "VOUTP_IVIRST_flg"
  VBCM_CountAlarm_enum/1 -> VBCM_CountAlarm_enum_Inproc/1  "VBCM_CountAlarm_enum"
  VBCM_CountAlarm_enum_Inproc/1 -> UnitConverter249/1
  UnitConverter249/1 -> VOUTP_CountAlarm_enum/1  "VOUTP_CountAlarm_enum"
  VBCM_MFSWTri_flg/1 -> VBCM_MFSWTri_flg_Inproc/1  "VBCM_MFSWTri_flg"
  VBCM_MFSWTri_flg_Inproc/1 -> UnitConverter250/1
  UnitConverter250/1 -> VOUTP_MFSWTri_flg/1  "VOUTP_MFSWTri_flg"
  VBCM_MirrorFlodPos_flg/1 -> VBCM_MirrorFlodPos_flg_Inproc/1  "VBCM_MirrorFlodPos_flg"
  VBCM_MirrorFlodPos_flg_Inproc/1 -> UnitConverter251/1
  UnitConverter251/1 -> VOUTP_MirrorFlodPos_flg/1  "VOUTP_MirrorFlodPos_flg"
  VBCM_FuelDoorPos_flg/1 -> VBCM_FuelDoorPos_flg_Inproc/1  "VBCM_FuelDoorPos_flg"
  VBCM_FuelDoorPos_flg_Inproc/1 -> UnitConverter252/1
  UnitConverter252/1 -> VOUTP_FuelDoorPos_flg/1  "VOUTP_FuelDoorPos_flg"
  VBCM_MFRDNBrightReq_pct/1 -> VBCM_MFRDNBrightReq_pct_Inproc/1  "VBCM_MFRDNBrightReq_pct"
  VBCM_MFRDNBrightReq_pct_Inproc/1 -> UnitConverter253/1
  UnitConverter253/1 -> VOUTP_MFRDNBrightReq_pct/1  "VOUTP_MFRDNBrightReq_pct"
  VBCM_PTGInnerSW2_enum/1 -> VBCM_PTGInnerSW2_enum_Inproc/1  "VBCM_PTGInnerSW2_enum"
  VBCM_PTGInnerSW2_enum_Inproc/1 -> UnitConverter254/1
  UnitConverter254/1 -> VOUTP_PTGInnerSW2_enum/1  "VOUTP_PTGInnerSW2_enum"
  VBCM_DrvWdwCtrlCmd_pct/1 -> VBCM_DrvWdwCtrlCmd_pct_Inproc/1  "VBCM_DrvWdwCtrlCmd_pct"
  VBCM_DrvWdwCtrlCmd_pct_Inproc/1 -> UnitConverter255/1
  UnitConverter255/1 -> VOUTP_DrvWdwCtrlCmd_pct/1  "VOUTP_DrvWdwCtrlCmd_pct"
  VBCM_PasWdwCtrlCmd_pct/1 -> VBCM_PasWdwCtrlCmd_pct_Inproc/1  "VBCM_PasWdwCtrlCmd_pct"
  VBCM_PasWdwCtrlCmd_pct_Inproc/1 -> UnitConverter256/1
  UnitConverter256/1 -> VOUTP_PasWdwCtrlCmd_pct/1  "VOUTP_PasWdwCtrlCmd_pct"
  VBCM_DrRWdwCtrlCmd_pct/1 -> VBCM_DrRWdwCtrlCmd_pct_Inproc/1  "VBCM_DrRWdwCtrlCmd_pct"
  VBCM_DrRWdwCtrlCmd_pct_Inproc/1 -> UnitConverter257/1
  UnitConverter257/1 -> VOUTP_DrRWdwCtrlCmd_pct/1  "VOUTP_DrRWdwCtrlCmd_pct"
  VBCM_PsRWdwCtrlCmd_pct/1 -> VBCM_PsRWdwCtrlCmd_pct_Inproc/1  "VBCM_PsRWdwCtrlCmd_pct"
  VBCM_PsRWdwCtrlCmd_pct_Inproc/1 -> UnitConverter258/1
  UnitConverter258/1 -> VOUTP_PsRWdwCtrlCmd_pct/1  "VOUTP_PsRWdwCtrlCmd_pct"
  VBCM_APMDoorControlSta_flg/1 -> VBCM_APMDoorControlSta_flg_Inproc/1  "VBCM_APMDoorControlSta_flg"
  VBCM_APMDoorControlSta_flg_Inproc/1 -> UnitConverter259/1
  UnitConverter259/1 -> VOUTP_APMDoorControlSta_flg/1  "VOUTP_APMDoorControlSta_flg"
  VBCM_AmbFunEN_flg/1 -> VBCM_AmbFunEN_flg_Inproc/1  "VBCM_AmbFunEN_flg"
  VBCM_AmbFunEN_flg_Inproc/1 -> UnitConverter260/1
  UnitConverter260/1 -> VOUTP_AmbFunEN_flg/1  "VOUTP_AmbFunEN_flg"
  VBCM_AmbWelEN_flg/1 -> VBCM_AmbWelEN_flg_Inproc/1  "VBCM_AmbWelEN_flg"
  VBCM_AmbWelEN_flg_Inproc/1 -> UnitConverter261/1
  UnitConverter261/1 -> VOUTP_AmbWelEN_flg/1  "VOUTP_AmbWelEN_flg"
  VBCM_AmbDimEN_flg/1 -> VBCM_AmbDimEN_flg_Inproc/1  "VBCM_AmbDimEN_flg"
  VBCM_AmbDimEN_flg_Inproc/1 -> UnitConverter262/1
  UnitConverter262/1 -> VOUTP_AmbDimEN_flg/1  "VOUTP_AmbDimEN_flg"
  VBCM_AmbLinkDriSta_flg/1 -> VBCM_AmbLinkDriSta_flg_Inproc/1  "VBCM_AmbLinkDriSta_flg"
  VBCM_AmbLinkDriSta_flg_Inproc/1 -> UnitConverter263/1
  UnitConverter263/1 -> VOUTP_AmbLinkDriSta_flg/1  "VOUTP_AmbLinkDriSta_flg"
  VBCM_AmbPwrWarnEN_flg/1 -> VBCM_AmbPwrWarnEN_flg_Inproc/1  "VBCM_AmbPwrWarnEN_flg"
  VBCM_AmbPwrWarnEN_flg_Inproc/1 -> UnitConverter264/1
  UnitConverter264/1 -> VOUTP_AmbPwrWarnEN_flg/1  "VOUTP_AmbPwrWarnEN_flg"
  VBCM_AmbODAEN_flg/1 -> VBCM_AmbODAEN_flg_Inproc/1  "VBCM_AmbODAEN_flg"
  VBCM_AmbODAEN_flg_Inproc/1 -> UnitConverter265/1
  UnitConverter265/1 -> VOUTP_AmbODAEN_flg/1  "VOUTP_AmbODAEN_flg"
  VBCM_AmbColorSta_enum/1 -> VBCM_AmbColorSta_enum_Inproc/1  "VBCM_AmbColorSta_enum"
  VBCM_AmbColorSta_enum_Inproc/1 -> UnitConverter266/1
  UnitConverter266/1 -> VOUTP_AmbColorSta_enum/1  "VOUTP_AmbColorSta_enum"
  VBCM_AmbBrightSta_enum/1 -> VBCM_AmbBrightSta_enum_Inproc/1  "VBCM_AmbBrightSta_enum"
  VBCM_AmbBrightSta_enum_Inproc/1 -> UnitConverter267/1
  UnitConverter267/1 -> VOUTP_AmbBrightSta_enum/1  "VOUTP_AmbBrightSta_enum"
  VBCM_LockAlarm_enum/1 -> VBCM_LockAlarm_enum_Inproc/1  "VBCM_LockAlarm_enum"
  VBCM_LockAlarm_enum_Inproc/1 -> UnitConverter268/1
  UnitConverter268/1 -> VOUTP_LockAlarm_enum/1  "VOUTP_LockAlarm_enum"
  VBCM_ATCtrl_enum/1 -> VBCM_ATCtrl_enum_Inproc/1  "VBCM_ATCtrl_enum"
  VBCM_ATCtrl_enum_Inproc/1 -> UnitConverter269/1
  UnitConverter269/1 -> VOUTP_ATCtrl_enum/1  "VOUTP_ATCtrl_enum"
  VBCM_fUnlockSingle_flg/1 -> VBCM_fUnlockSingle_flg_Inproc/1  "VBCM_fUnlockSingle_flg"
  VBCM_fUnlockSingle_flg_Inproc/1 -> UnitConverter270/1
  UnitConverter270/1 -> VOUTP_fUnlockSingle_flg/1  "VOUTP_fUnlockSingle_flg"
  VBCM_UserNow_enum/1 -> VBCM_UserNow_enum_Inproc/1  "VBCM_UserNow_enum"
  VBCM_UserNow_enum_Inproc/1 -> UnitConverter271/1
  UnitConverter271/1 -> VOUTP_UserNow_enum/1  "VOUTP_UserNow_enum"
  VBCM_AmbFunENFlash_enum/1 -> VBCM_AmbFunENFlash_enum_Inproc/1  "VBCM_AmbFunENFlash_enum"
  VBCM_AmbFunENFlash_enum_Inproc/1 -> UnitConverter272/1
  UnitConverter272/1 -> VOUTP_AmbFunENFlash_enum/1  "VOUTP_AmbFunENFlash_enum"
  VBCM_AmbWelENFlash_enum/1 -> VBCM_AmbWelENFlash_enum_Inproc/1  "VBCM_AmbWelENFlash_enum"
  VBCM_AmbWelENFlash_enum_Inproc/1 -> UnitConverter273/1
  UnitConverter273/1 -> VOUTP_AmbWelENFlash_enum/1  "VOUTP_AmbWelENFlash_enum"
  VBCM_AmbDimENFlash_enum/1 -> VBCM_AmbDimENFlash_enum_Inproc/1  "VBCM_AmbDimENFlash_enum"
  VBCM_AmbDimENFlash_enum_Inproc/1 -> UnitConverter274/1
  UnitConverter274/1 -> VOUTP_AmbDimENFlash_enum/1  "VOUTP_AmbDimENFlash_enum"
  VBCM_AmbLinkDriStaFlash_enum/1 -> VBCM_AmbLinkDriStaFlash_enum_Inproc/1  "VBCM_AmbLinkDriStaFlash_enum"
  VBCM_AmbLinkDriStaFlash_enum_Inproc/1 -> UnitConverter275/1
  UnitConverter275/1 -> VOUTP_AmbLinkDriStaFlash_enum/1  "VOUTP_AmbLinkDriStaFlash_enum"
  VBCM_AmbPwrWarnENFlash_enum/1 -> VBCM_AmbPwrWarnENFlash_enum_Inproc/1  "VBCM_AmbPwrWarnENFlash_enum"
  VBCM_AmbPwrWarnENFlash_enum_Inproc/1 -> UnitConverter276/1
  UnitConverter276/1 -> VOUTP_AmbPwrWarnENFlash_enum/1  "VOUTP_AmbPwrWarnENFlash_enum"
  VBCM_AmbODAENFlash_enum/1 -> VBCM_AmbODAENFlash_enum_Inproc/1  "VBCM_AmbODAENFlash_enum"
  VBCM_AmbODAENFlash_enum_Inproc/1 -> UnitConverter277/1
  UnitConverter277/1 -> VOUTP_AmbODAENFlash_enum/1  "VOUTP_AmbODAENFlash_enum"
  VBCM_AmbColorSta1_enum/1 -> VBCM_AmbColorSta1_enum_Inproc/1  "VBCM_AmbColorSta1_enum"
  VBCM_AmbColorSta1_enum_Inproc/1 -> UnitConverter278/1
  UnitConverter278/1 -> VOUTP_AmbColorSta1_enum/1  "VOUTP_AmbColorSta1_enum"
  VBCM_AmbColorSta2_enum/1 -> VBCM_AmbColorSta2_enum_Inproc/1  "VBCM_AmbColorSta2_enum"
  VBCM_AmbColorSta2_enum_Inproc/1 -> UnitConverter279/1
  UnitConverter279/1 -> VOUTP_AmbColorSta2_enum/1  "VOUTP_AmbColorSta2_enum"
  VBCM_AmbColorSta3_enum/1 -> VBCM_AmbColorSta3_enum_Inproc/1  "VBCM_AmbColorSta3_enum"
  VBCM_AmbColorSta3_enum_Inproc/1 -> UnitConverter280/1
  UnitConverter280/1 -> VOUTP_AmbColorSta3_enum/1  "VOUTP_AmbColorSta3_enum"
  VBCM_AmbColorSta4_enum/1 -> VBCM_AmbColorSta4_enum_Inproc/1  "VBCM_AmbColorSta4_enum"
  VBCM_AmbColorSta4_enum_Inproc/1 -> UnitConverter281/1
  UnitConverter281/1 -> VOUTP_AmbColorSta4_enum/1  "VOUTP_AmbColorSta4_enum"
  VBCM_AmbColorSta5_enum/1 -> VBCM_AmbColorSta5_enum_Inproc/1  "VBCM_AmbColorSta5_enum"
  VBCM_AmbColorSta5_enum_Inproc/1 -> UnitConverter282/1
  UnitConverter282/1 -> VOUTP_AmbColorSta5_enum/1  "VOUTP_AmbColorSta5_enum"
  VBCM_AmbColorSta7_enum/1 -> VBCM_AmbColorSta7_enum_Inproc/1  "VBCM_AmbColorSta7_enum"
  VBCM_AmbColorSta7_enum_Inproc/1 -> UnitConverter283/1
  UnitConverter283/1 -> VOUTP_AmbColorSta7_enum/1  "VOUTP_AmbColorSta7_enum"
  VBCM_AmbBrightnessSta1_enum/1 -> VBCM_AmbBrightnessSta1_enum_Inproc/1  "VBCM_AmbBrightnessSta1_enum"
  VBCM_AmbBrightnessSta1_enum_Inproc/1 -> UnitConverter284/1
  UnitConverter284/1 -> VOUTP_AmbBrightnessSta1_enum/1  "VOUTP_AmbBrightnessSta1_enum"
  VBCM_AmbBrightnessSta2_enum/1 -> VBCM_AmbBrightnessSta2_enum_Inproc/1  "VBCM_AmbBrightnessSta2_enum"
  VBCM_AmbBrightnessSta2_enum_Inproc/1 -> UnitConverter285/1
  UnitConverter285/1 -> VOUTP_AmbBrightnessSta2_enum/1  "VOUTP_AmbBrightnessSta2_enum"
  VBCM_AmbBrightnessSta3_enum/1 -> VBCM_AmbBrightnessSta3_enum_Inproc/1  "VBCM_AmbBrightnessSta3_enum"
  VBCM_AmbBrightnessSta3_enum_Inproc/1 -> UnitConverter286/1
  UnitConverter286/1 -> VOUTP_AmbBrightnessSta3_enum/1  "VOUTP_AmbBrightnessSta3_enum"
  VBCM_AmbBrightnessSta4_enum/1 -> VBCM_AmbBrightnessSta4_enum_Inproc/1  "VBCM_AmbBrightnessSta4_enum"
  VBCM_AmbBrightnessSta4_enum_Inproc/1 -> UnitConverter287/1
  UnitConverter287/1 -> VOUTP_AmbBrightnessSta4_enum/1  "VOUTP_AmbBrightnessSta4_enum"
  VBCM_AmbBrightnessSta5_enum/1 -> VBCM_AmbBrightnessSta5_enum_Inproc/1  "VBCM_AmbBrightnessSta5_enum"
  VBCM_AmbBrightnessSta5_enum_Inproc/1 -> UnitConverter288/1
  UnitConverter288/1 -> VOUTP_AmbBrightnessSta5_enum/1  "VOUTP_AmbBrightnessSta5_enum"
  VBCM_AmbBrightnessSta7_enum/1 -> VBCM_AmbBrightnessSta7_enum_Inproc/1  "VBCM_AmbBrightnessSta7_enum"
  VBCM_AmbBrightnessSta7_enum_Inproc/1 -> UnitConverter289/1
  UnitConverter289/1 -> VOUTP_AmbBrightnessSta7_enum/1  "VOUTP_AmbBrightnessSta7_enum"
  VBCM_HazardIND_flg/1 -> VBCM_HazardIND_flg_Inproc/1  "VBCM_HazardIND_flg"
  VBCM_HazardIND_flg_Inproc/1 -> UnitConverter290/1
  UnitConverter290/1 -> VOUTP_HazardIND_flg/1  "VOUTP_HazardIND_flg"
  VBCM_DimSwSta_flg/1 -> VBCM_DimSwSta_flg_Inproc/1  "VBCM_DimSwSta_flg"
  VBCM_DimSwSta_flg_Inproc/1 -> UnitConverter291/1
  UnitConverter291/1 -> VOUTP_DimSwSta_flg/1  "VOUTP_DimSwSta_flg"
  VBCM_PassSWSta_flg/1 -> VBCM_PassSWSta_flg_Inproc/1  "VBCM_PassSWSta_flg"
  VBCM_PassSWSta_flg_Inproc/1 -> UnitConverter292/1
  UnitConverter292/1 -> VOUTP_PassSWSta_flg/1  "VOUTP_PassSWSta_flg"
  VBCM_FWipSwSta_enum/1 -> VBCM_FWipSwSta_enum_Inproc/1  "VBCM_FWipSwSta_enum"
  VBCM_FWipSwSta_enum_Inproc/1 -> UnitConverter293/1
  UnitConverter293/1 -> VOUTP_FWipSwSta_enum/1  "VOUTP_FWipSwSta_enum"
  VBCM_FWasSwSta_enum/1 -> VBCM_FWasSwSta_enum_Inproc/1  "VBCM_FWasSwSta_enum"
  VBCM_FWasSwSta_enum_Inproc/1 -> UnitConverter294/1
  UnitConverter294/1 -> VOUTP_FWasSwSta_enum/1  "VOUTP_FWasSwSta_enum"
  VBCM_TurnSwSta_enum/1 -> VBCM_TurnSwSta_enum_Inproc/1  "VBCM_TurnSwSta_enum"
  VBCM_TurnSwSta_enum_Inproc/1 -> UnitConverter295/1
  UnitConverter295/1 -> VOUTP_TurnSwSta_enum/1  "VOUTP_TurnSwSta_enum"
  VBCM_TurnSwTSetSta_enum/1 -> VBCM_TurnSwTSetSta_enum_Inproc/1  "VBCM_TurnSwTSetSta_enum"
  VBCM_TurnSwTSetSta_enum_Inproc/1 -> UnitConverter296/1
  UnitConverter296/1 -> VOUTP_TurnSwTSetSta_enum/1  "VOUTP_TurnSwTSetSta_enum"
  VBCM_SPTGENFun_flg/1 -> VBCM_SPTGENFun_flg_Inproc/1  "VBCM_SPTGENFun_flg"
  VBCM_SPTGENFun_flg_Inproc/1 -> UnitConverter297/1
  UnitConverter297/1 -> VOUTP_SPTGENFun_flg/1  "VOUTP_SPTGENFun_flg"
  VBCM_SPTGENFunMem_enum/1 -> VBCM_SPTGENFunMem_enum_Inproc/1  "VBCM_SPTGENFunMem_enum"
  VBCM_SPTGENFunMem_enum_Inproc/1 -> UnitConverter298/1
  UnitConverter298/1 -> VOUTP_SPTGENFunMem_enum/1  "VOUTP_SPTGENFunMem_enum"
  VBCM_OutMode_enum/1 -> VBCM_OutMode_enum_Inproc/1  "VBCM_OutMode_enum"
  VBCM_OutMode_enum_Inproc/1 -> UnitConverter299/1
  UnitConverter299/1 -> VOUTP_OutMode_enum/1  "VOUTP_OutMode_enum"
  VBCM_TurnSwTimeSetSta123_enum/1 -> VBCM_TurnSwTimeSetSta123_enum_Inproc/1  "VBCM_TurnSwTimeSetSta123_enum"
  VBCM_TurnSwTimeSetSta123_enum_Inproc/1 -> UnitConverter300/1
  UnitConverter300/1 -> VOUTP_TurnSwTimeSetSta123_enum/1  "VOUTP_TurnSwTimeSetSta123_enum"
  VBCM_TurnSwTimeSetSta457_enum/1 -> VBCM_TurnSwTimeSetSta457_enum_Inproc/1  "VBCM_TurnSwTimeSetSta457_enum"
  VBCM_TurnSwTimeSetSta457_enum_Inproc/1 -> UnitConverter301/1
  UnitConverter301/1 -> VOUTP_TurnSwTimeSetSta457_enum/1  "VOUTP_TurnSwTimeSetSta457_enum"
  VBCM_FDLHandleLampCmd_flg/1 -> VBCM_FDLHandleLampCmd_flg_Inproc/1  "VBCM_FDLHandleLampCmd_flg"
  VBCM_FDLHandleLampCmd_flg_Inproc/1 -> UnitConverter302/1
  UnitConverter302/1 -> VOUTP_FDLHandleLampCmd_flg/1  "VOUTP_FDLHandleLampCmd_flg"
  VBCM_FDRHandleLampCmd_flg/1 -> VBCM_FDRHandleLampCmd_flg_Inproc/1  "VBCM_FDRHandleLampCmd_flg"
  VBCM_FDRHandleLampCmd_flg_Inproc/1 -> UnitConverter303/1
  UnitConverter303/1 -> VOUTP_FDRHandleLampCmd_flg/1  "VOUTP_FDRHandleLampCmd_flg"
  VBCM_FDHandleCmd_enum/1 -> VBCM_FDHandleCmd_enum_Inproc/1  "VBCM_FDHandleCmd_enum"
  VBCM_FDHandleCmd_enum_Inproc/1 -> UnitConverter304/1
  UnitConverter304/1 -> VOUTP_FDHandleCmd_enum/1  "VOUTP_FDHandleCmd_enum"
  VBCM_HBeamADB_enum/1 -> VBCM_HBeamADB_enum_Inproc/1  "VBCM_HBeamADB_enum"
  VBCM_HBeamADB_enum_Inproc/1 -> UnitConverter305/1
  UnitConverter305/1 -> VOUTP_HBeamADB_enum/1  "VOUTP_HBeamADB_enum"
  VBCM_WalkInUnLkENMem_enum/1 -> VBCM_WalkInUnLkENMem_enum_Inproc/1  "VBCM_WalkInUnLkENMem_enum"
  VBCM_WalkInUnLkENMem_enum_Inproc/1 -> UnitConverter306/1
  UnitConverter306/1 -> VOUTP_WalkInUnLkENMem_enum/1  "VOUTP_WalkInUnLkENMem_enum"
  VBCM_WalkOutLkENMem_enum/1 -> VBCM_WalkOutLkENMem_enum_Inproc/1  "VBCM_WalkOutLkENMem_enum"
  VBCM_WalkOutLkENMem_enum_Inproc/1 -> UnitConverter307/1
  UnitConverter307/1 -> VOUTP_WalkOutLkENMem_enum/1  "VOUTP_WalkOutLkENMem_enum"
  VBCM_RmLpModeENMem_enum/1 -> VBCM_RmLpModeENMem_enum_Inproc/1  "VBCM_RmLpModeENMem_enum"
  VBCM_RmLpModeENMem_enum_Inproc/1 -> UnitConverter308/1
  UnitConverter308/1 -> VOUTP_RmLpModeENMem_enum/1  "VOUTP_RmLpModeENMem_enum"
  VBCM_LockSettingStaMem_enum/1 -> VBCM_LockSettingStaMem_enum_Inproc/1  "VBCM_LockSettingStaMem_enum"
  VBCM_LockSettingStaMem_enum_Inproc/1 -> UnitConverter309/1
  UnitConverter309/1 -> VOUTP_LockSettingStaMem_enum/1  "VOUTP_LockSettingStaMem_enum"
  VBCM_FollowMeENMem_enum/1 -> VBCM_FollowMeENMem_enum_Inproc/1  "VBCM_FollowMeENMem_enum"
  VBCM_FollowMeENMem_enum_Inproc/1 -> UnitConverter310/1
  UnitConverter310/1 -> VOUTP_FollowMeENMem_enum/1  "VOUTP_FollowMeENMem_enum"
  VBCM_WalkInUnLkENFunSta_flg/1 -> VBCM_WalkInUnLkENFunSta_flg_Inproc/1  "VBCM_WalkInUnLkENFunSta_flg"
  VBCM_WalkInUnLkENFunSta_flg_Inproc/1 -> UnitConverter311/1
  UnitConverter311/1 -> VOUTP_WalkInUnLkENFunSta_flg/1  "VOUTP_WalkInUnLkENFunSta_flg"
  VBCM_WalkOutLkENFunSta_flg/1 -> VBCM_WalkOutLkENFunSta_flg_Inproc/1  "VBCM_WalkOutLkENFunSta_flg"
  VBCM_WalkOutLkENFunSta_flg_Inproc/1 -> UnitConverter312/1
  UnitConverter312/1 -> VOUTP_WalkOutLkENFunSta_flg/1  "VOUTP_WalkOutLkENFunSta_flg"
  VBCM_RmLpModeENFunSta_flg/1 -> VBCM_RmLpModeENFunSta_flg_Inproc/1  "VBCM_RmLpModeENFunSta_flg"
  VBCM_RmLpModeENFunSta_flg_Inproc/1 -> UnitConverter313/1
  UnitConverter313/1 -> VOUTP_RmLpModeENFunSta_flg/1  "VOUTP_RmLpModeENFunSta_flg"
  VBCM_FollowMeENFunSta_flg/1 -> VBCM_FollowMeENFunSta_flg_Inproc/1  "VBCM_FollowMeENFunSta_flg"
  VBCM_FollowMeENFunSta_flg_Inproc/1 -> UnitConverter314/1
  UnitConverter314/1 -> VOUTP_FollowMeENFunSta_flg/1  "VOUTP_FollowMeENFunSta_flg"
  VBCM_HoodRelCmd_flg/1 -> VBCM_HoodRelCmd_flg_Inproc/1  "VBCM_HoodRelCmd_flg"
  VBCM_HoodRelCmd_flg_Inproc/1 -> UnitConverter315/1
  UnitConverter315/1 -> VOUTP_HoodRelCmd_flg/1  "VOUTP_HoodRelCmd_flg"
  VBCM_WelcomeLight_enum/1 -> VBCM_WelcomeLight_enum_Inproc/1  "VBCM_WelcomeLight_enum"
  VBCM_WelcomeLight_enum_Inproc/1 -> UnitConverter316/1
  UnitConverter316/1 -> VOUTP_WelcomeLight_enum/1  "VOUTP_WelcomeLight_enum"
  VBCM_PTGOpenHeightSta_enum/1 -> VBCM_PTGOpenHeightSta_enum_Inproc/1  "VBCM_PTGOpenHeightSta_enum"
  VBCM_PTGOpenHeightSta_enum_Inproc/1 -> UnitConverter317/1
  UnitConverter317/1 -> VOUTP_PTGOpenHeightSta_enum/1  "VOUTP_PTGOpenHeightSta_enum"
  VBCM_UserHeightSet_cnt/1 -> VBCM_UserHeightSet_cnt_Inproc/1  "VBCM_UserHeightSet_cnt"
  VBCM_UserHeightSet_cnt_Inproc/1 -> UnitConverter318/1
  UnitConverter318/1 -> VOUTP_UserHeightSet_cnt/1  "VOUTP_UserHeightSet_cnt"
  VBCM_PTGUserHeight1_cnt/1 -> VBCM_PTGUserHeight1_cnt_Inproc/1  "VBCM_PTGUserHeight1_cnt"
  VBCM_PTGUserHeight1_cnt_Inproc/1 -> UnitConverter319/1
  UnitConverter319/1 -> VOUTP_PTGUserHeight1_cnt/1  "VOUTP_PTGUserHeight1_cnt"
  VBCM_PTGUserHeight2_cnt/1 -> VBCM_PTGUserHeight2_cnt_Inproc/1  "VBCM_PTGUserHeight2_cnt"
  VBCM_PTGUserHeight2_cnt_Inproc/1 -> UnitConverter320/1
  UnitConverter320/1 -> VOUTP_PTGUserHeight2_cnt/1  "VOUTP_PTGUserHeight2_cnt"
  VBCM_PTGUserHeight3_cnt/1 -> VBCM_PTGUserHeight3_cnt_Inproc/1  "VBCM_PTGUserHeight3_cnt"
  VBCM_PTGUserHeight3_cnt_Inproc/1 -> UnitConverter321/1
  UnitConverter321/1 -> VOUTP_PTGUserHeight3_cnt/1  "VOUTP_PTGUserHeight3_cnt"
  VBCM_PTGUserHeight4_cnt/1 -> VBCM_PTGUserHeight4_cnt_Inproc/1  "VBCM_PTGUserHeight4_cnt"
  VBCM_PTGUserHeight4_cnt_Inproc/1 -> UnitConverter322/1
  UnitConverter322/1 -> VOUTP_PTGUserHeight4_cnt/1  "VOUTP_PTGUserHeight4_cnt"
  VBCM_PTGUserHeight5_cnt/1 -> VBCM_PTGUserHeight5_cnt_Inproc/1  "VBCM_PTGUserHeight5_cnt"
  VBCM_PTGUserHeight5_cnt_Inproc/1 -> UnitConverter323/1
  UnitConverter323/1 -> VOUTP_PTGUserHeight5_cnt/1  "VOUTP_PTGUserHeight5_cnt"
  VBCM_PTGUserHeight7_cnt/1 -> VBCM_PTGUserHeight7_cnt_Inproc/1  "VBCM_PTGUserHeight7_cnt"
  VBCM_PTGUserHeight7_cnt_Inproc/1 -> UnitConverter324/1
  UnitConverter324/1 -> VOUTP_PTGUserHeight7_cnt/1  "VOUTP_PTGUserHeight7_cnt"
  VBCM_PTGOpenHeight12_enum/1 -> VBCM_PTGOpenHeight12_enum_Inproc/1  "VBCM_PTGOpenHeight12_enum"
  VBCM_PTGOpenHeight12_enum_Inproc/1 -> UnitConverter325/1
  UnitConverter325/1 -> VOUTP_PTGOpenHeight12_enum/1  "VOUTP_PTGOpenHeight12_enum"
  VBCM_PTGOpenHeight34_enum/1 -> VBCM_PTGOpenHeight34_enum_Inproc/1  "VBCM_PTGOpenHeight34_enum"
  VBCM_PTGOpenHeight34_enum_Inproc/1 -> UnitConverter326/1
  UnitConverter326/1 -> VOUTP_PTGOpenHeight34_enum/1  "VOUTP_PTGOpenHeight34_enum"
  VBCM_PTGOpenHeight57_enum/1 -> VBCM_PTGOpenHeight57_enum_Inproc/1  "VBCM_PTGOpenHeight57_enum"
  VBCM_PTGOpenHeight57_enum_Inproc/1 -> UnitConverter327/1
  UnitConverter327/1 -> VOUTP_PTGOpenHeight57_enum/1  "VOUTP_PTGOpenHeight57_enum"
  VBCM_SenstivityPosnCmd_enum/1 -> VBCM_SenstivityPosnCmd_enum_Inproc/1  "VBCM_SenstivityPosnCmd_enum"
  VBCM_SenstivityPosnCmd_enum_Inproc/1 -> UnitConverter328/1
  UnitConverter328/1 -> VOUTP_SenstivityPosnCmd_enum/1  "VOUTP_SenstivityPosnCmd_enum"
  VBCM_TimeGapLevelSta_enum/1 -> VBCM_TimeGapLevelSta_enum_Inproc/1  "VBCM_TimeGapLevelSta_enum"
  VBCM_TimeGapLevelSta_enum_Inproc/1 -> UnitConverter329/1
  UnitConverter329/1 -> VOUTP_TimeGapLevelSta_enum/1  "VOUTP_TimeGapLevelSta_enum"
  VBCM_ACCLevelMem12_enum/1 -> VBCM_ACCLevelMem12_enum_Inproc/1  "VBCM_ACCLevelMem12_enum"
  VBCM_ACCLevelMem12_enum_Inproc/1 -> UnitConverter330/1
  UnitConverter330/1 -> VOUTP_ACCLevelMem12_enum/1  "VOUTP_ACCLevelMem12_enum"
  VBCM_ACCLevelMem34_enum/1 -> VBCM_ACCLevelMem34_enum_Inproc/1  "VBCM_ACCLevelMem34_enum"
  VBCM_ACCLevelMem34_enum_Inproc/1 -> UnitConverter331/1
  UnitConverter331/1 -> VOUTP_ACCLevelMem34_enum/1  "VOUTP_ACCLevelMem34_enum"
  VBCM_ACCLevelMem57_enum/1 -> VBCM_ACCLevelMem57_enum_Inproc/1  "VBCM_ACCLevelMem57_enum"
  VBCM_ACCLevelMem57_enum_Inproc/1 -> UnitConverter332/1
  UnitConverter332/1 -> VOUTP_ACCLevelMem57_enum/1  "VOUTP_ACCLevelMem57_enum"
  VBCM_LRightStaCmd_flg/1 -> VBCM_LRightStaCmd_flg_Inproc/1  "VBCM_LRightStaCmd_flg"
  VBCM_LRightStaCmd_flg_Inproc/1 -> UnitConverter333/1
  UnitConverter333/1 -> VOUTP_LRightStaCmd_flg/1  "VOUTP_LRightStaCmd_flg"
  VBCM_LLeftStaCmd_flg/1 -> VBCM_LLeftStaCmd_flg_Inproc/1  "VBCM_LLeftStaCmd_flg"
  VBCM_LLeftStaCmd_flg_Inproc/1 -> UnitConverter334/1
  UnitConverter334/1 -> VOUTP_LLeftStaCmd_flg/1  "VOUTP_LLeftStaCmd_flg"
  VBCM_AutoLockSta_flg/1 -> VBCM_AutoLockSta_flg_Inproc/1  "VBCM_AutoLockSta_flg"
  VBCM_AutoLockSta_flg_Inproc/1 -> UnitConverter335/1
  UnitConverter335/1 -> VOUTP_AutoLockSta_flg/1  "VOUTP_AutoLockSta_flg"
  VBCM_AutoLockMem_enum/1 -> VBCM_AutoLockMem_enum_Inproc/1  "VBCM_AutoLockMem_enum"
  VBCM_AutoLockMem_enum_Inproc/1 -> UnitConverter336/1
  UnitConverter336/1 -> VOUTP_AutoLockMem_enum/1  "VOUTP_AutoLockMem_enum"
  VBCM_AutoUnlockSta_flg/1 -> VBCM_AutoUnlockSta_flg_Inproc/1  "VBCM_AutoUnlockSta_flg"
  VBCM_AutoUnlockSta_flg_Inproc/1 -> UnitConverter337/1
  UnitConverter337/1 -> VOUTP_AutoUnlockSta_flg/1  "VOUTP_AutoUnlockSta_flg"
  VBCM_AutoUnlockMem_enum/1 -> VBCM_AutoUnlockMem_enum_Inproc/1  "VBCM_AutoUnlockMem_enum"
  VBCM_AutoUnlockMem_enum_Inproc/1 -> UnitConverter338/1
  UnitConverter338/1 -> VOUTP_AutoUnlockMem_enum/1  "VOUTP_AutoUnlockMem_enum"
  VBCM_HMIKey1FuncSta_enum/1 -> VBCM_HMIKey1FuncSta_enum_Inproc/1  "VBCM_HMIKey1FuncSta_enum"
  VBCM_HMIKey1FuncSta_enum_Inproc/1 -> UnitConverter339/1
  UnitConverter339/1 -> VOUTP_HMIKey1FuncSta_enum/1  "VOUTP_HMIKey1FuncSta_enum"
  VBCM_HMIKey2FuncSta_enum/1 -> VBCM_HMIKey2FuncSta_enum_Inproc/1  "VBCM_HMIKey2FuncSta_enum"
  VBCM_HMIKey2FuncSta_enum_Inproc/1 -> UnitConverter340/1
  UnitConverter340/1 -> VOUTP_HMIKey2FuncSta_enum/1  "VOUTP_HMIKey2FuncSta_enum"
  VBCM_HMIKey3FuncSta_enum/1 -> VBCM_HMIKey3FuncSta_enum_Inproc/1  "VBCM_HMIKey3FuncSta_enum"
  VBCM_HMIKey3FuncSta_enum_Inproc/1 -> UnitConverter341/1
  UnitConverter341/1 -> VOUTP_HMIKey3FuncSta_enum/1  "VOUTP_HMIKey3FuncSta_enum"
  VBCM_HMIKey4FuncSta_enum/1 -> VBCM_HMIKey4FuncSta_enum_Inproc/1  "VBCM_HMIKey4FuncSta_enum"
  VBCM_HMIKey4FuncSta_enum_Inproc/1 -> UnitConverter342/1
  UnitConverter342/1 -> VOUTP_HMIKey4FuncSta_enum/1  "VOUTP_HMIKey4FuncSta_enum"
  VBCM_HMIKey5FuncSta_enum/1 -> VBCM_HMIKey5FuncSta_enum_Inproc/1  "VBCM_HMIKey5FuncSta_enum"
  VBCM_HMIKey5FuncSta_enum_Inproc/1 -> UnitConverter343/1
  UnitConverter343/1 -> VOUTP_HMIKey5FuncSta_enum/1  "VOUTP_HMIKey5FuncSta_enum"
  VBCM_HMIKey6FuncSta_enum/1 -> VBCM_HMIKey6FuncSta_enum_Inproc/1  "VBCM_HMIKey6FuncSta_enum"
  VBCM_HMIKey6FuncSta_enum_Inproc/1 -> UnitConverter344/1
  UnitConverter344/1 -> VOUTP_HMIKey6FuncSta_enum/1  "VOUTP_HMIKey6FuncSta_enum"
  VBCM_HMIKey7FuncSta_enum/1 -> VBCM_HMIKey7FuncSta_enum_Inproc/1  "VBCM_HMIKey7FuncSta_enum"
  VBCM_HMIKey7FuncSta_enum_Inproc/1 -> UnitConverter345/1
  UnitConverter345/1 -> VOUTP_HMIKey7FuncSta_enum/1  "VOUTP_HMIKey7FuncSta_enum"
  VBCM_HMIKey8FuncSta_enum/1 -> VBCM_HMIKey8FuncSta_enum_Inproc/1  "VBCM_HMIKey8FuncSta_enum"
  VBCM_HMIKey8FuncSta_enum_Inproc/1 -> UnitConverter346/1
  UnitConverter346/1 -> VOUTP_HMIKey8FuncSta_enum/1  "VOUTP_HMIKey8FuncSta_enum"
  VBCM_AutoWipHSpdENSta_flg/1 -> VBCM_AutoWipHSpdENSta_flg_Inproc/1  "VBCM_AutoWipHSpdENSta_flg"
  VBCM_AutoWipHSpdENSta_flg_Inproc/1 -> UnitConverter347/1
  UnitConverter347/1 -> VOUTP_AutoWipHSpdENSta_flg/1  "VOUTP_AutoWipHSpdENSta_flg"
  VBCM_DrvWdwReqAP_enum/1 -> VBCM_DrvWdwReqAP_enum_Inproc/1  "VBCM_DrvWdwReqAP_enum"
  VBCM_DrvWdwReqAP_enum_Inproc/1 -> UnitConverter348/1
  UnitConverter348/1 -> VOUTP_DrvWdwReqAP_enum/1  "VOUTP_DrvWdwReqAP_enum"
  VBCM_PasWdwReqAP_enum/1 -> VBCM_PasWdwReqAP_enum_Inproc/1  "VBCM_PasWdwReqAP_enum"
  VBCM_PasWdwReqAP_enum_Inproc/1 -> UnitConverter349/1
  UnitConverter349/1 -> VOUTP_PasWdwReqAP_enum/1  "VOUTP_PasWdwReqAP_enum"
  VBCM_DrRWdwReqAP_enum/1 -> VBCM_DrRWdwReqAP_enum_Inproc/1  "VBCM_DrRWdwReqAP_enum"
  VBCM_DrRWdwReqAP_enum_Inproc/1 -> UnitConverter350/1
  UnitConverter350/1 -> VOUTP_DrRWdwReqAP_enum/1  "VOUTP_DrRWdwReqAP_enum"
  VBCM_PsRWdwReqAP_enum/1 -> VBCM_PsRWdwReqAP_enum_Inproc/1  "VBCM_PsRWdwReqAP_enum"
  VBCM_PsRWdwReqAP_enum_Inproc/1 -> UnitConverter351/1
  UnitConverter351/1 -> VOUTP_PsRWdwReqAP_enum/1  "VOUTP_PsRWdwReqAP_enum"
  VBCM_CLWinLockDrSta_flg/1 -> VBCM_CLWinLockDrSta_flg_Inproc/1  "VBCM_CLWinLockDrSta_flg"
  VBCM_CLWinLockDrSta_flg_Inproc/1 -> UnitConverter352/1
  UnitConverter352/1 -> VOUTP_CLWinLockDrSta_flg/1  "VOUTP_CLWinLockDrSta_flg"
  VBCM_CLWinLockDrStaMem_enum/1 -> VBCM_CLWinLockDrStaMem_enum_Inproc/1  "VBCM_CLWinLockDrStaMem_enum"
  VBCM_CLWinLockDrStaMem_enum_Inproc/1 -> UnitConverter353/1
  UnitConverter353/1 -> VOUTP_CLWinLockDrStaMem_enum/1  "VOUTP_CLWinLockDrStaMem_enum"
  VBCM_WinLFOpenedSta_pct/1 -> VBCM_WinLFOpenedSta_pct_Inproc/1  "VBCM_WinLFOpenedSta_pct"
  VBCM_WinLFOpenedSta_pct_Inproc/1 -> UnitConverter354/1
  UnitConverter354/1 -> VOUTP_WinLFOpenedSta_pct/1  "VOUTP_WinLFOpenedSta_pct"
  VBCM_WinRFOpenedSta_pct/1 -> VBCM_WinRFOpenedSta_pct_Inproc/1  "VBCM_WinRFOpenedSta_pct"
  VBCM_WinRFOpenedSta_pct_Inproc/1 -> UnitConverter355/1
  UnitConverter355/1 -> VOUTP_WinRFOpenedSta_pct/1  "VOUTP_WinRFOpenedSta_pct"
  VBCM_WinLROpenedSta_pct/1 -> VBCM_WinLROpenedSta_pct_Inproc/1  "VBCM_WinLROpenedSta_pct"
  VBCM_WinLROpenedSta_pct_Inproc/1 -> UnitConverter356/1
  UnitConverter356/1 -> VOUTP_WinLROpenedSta_pct/1  "VOUTP_WinLROpenedSta_pct"
  VBCM_WinRROpenedSta_pct/1 -> VBCM_WinRROpenedSta_pct_Inproc/1  "VBCM_WinRROpenedSta_pct"
  VBCM_WinRROpenedSta_pct_Inproc/1 -> UnitConverter357/1
  UnitConverter357/1 -> VOUTP_WinRROpenedSta_pct/1  "VOUTP_WinRROpenedSta_pct"
  VDDM_C3BMS6RCDTC_raw32/1 -> VDDM_C3BMS6RCDTC_raw32_Inproc/1  "VDDM_C3BMS6RCDTC_raw32"
  VDDM_C3BMS6RCDTC_raw32_Inproc/1 -> UnitConverter358/1
  UnitConverter358/1 -> VOUTP_C3BMS6RCDTC_raw32/1  "VOUTP_C3BMS6RCDTC_raw32"
  VDDM_C3BMS6CSDTC_raw32/1 -> VDDM_C3BMS6CSDTC_raw32_Inproc/1  "VDDM_C3BMS6CSDTC_raw32"
  VDDM_C3BMS6CSDTC_raw32_Inproc/1 -> UnitConverter359/1
  UnitConverter359/1 -> VOUTP_C3BMS6CSDTC_raw32/1  "VOUTP_C3BMS6CSDTC_raw32"
  VDDM_C3BMS6LCDTC_raw32/1 -> VDDM_C3BMS6LCDTC_raw32_Inproc/1  "VDDM_C3BMS6LCDTC_raw32"
  VDDM_C3BMS6LCDTC_raw32_Inproc/1 -> UnitConverter360/1
  UnitConverter360/1 -> VOUTP_C3BMS6LCDTC_raw32/1  "VOUTP_C3BMS6LCDTC_raw32"
  VDDM_C3BMS1RCDTC_raw32/1 -> VDDM_C3BMS1RCDTC_raw32_Inproc/1  "VDDM_C3BMS1RCDTC_raw32"
  VDDM_C3BMS1RCDTC_raw32_Inproc/1 -> UnitConverter361/1
  UnitConverter361/1 -> VOUTP_C3BMS1RCDTC_raw32/1  "VOUTP_C3BMS1RCDTC_raw32"
  VDDM_C3BMS1CSDTC_raw32/1 -> VDDM_C3BMS1CSDTC_raw32_Inproc/1  "VDDM_C3BMS1CSDTC_raw32"
  VDDM_C3BMS1CSDTC_raw32_Inproc/1 -> UnitConverter362/1
  UnitConverter362/1 -> VOUTP_C3BMS1CSDTC_raw32/1  "VOUTP_C3BMS1CSDTC_raw32"
  VDDM_C3BMS1LCDTC_raw32/1 -> VDDM_C3BMS1LCDTC_raw32_Inproc/1  "VDDM_C3BMS1LCDTC_raw32"
  VDDM_C3BMS1LCDTC_raw32_Inproc/1 -> UnitConverter363/1
  UnitConverter363/1 -> VOUTP_C3BMS1LCDTC_raw32/1  "VOUTP_C3BMS1LCDTC_raw32"
  VDDM_C3CCU1RCDTC_raw32/1 -> VDDM_C3CCU1RCDTC_raw32_Inproc/1  "VDDM_C3CCU1RCDTC_raw32"
  VDDM_C3CCU1RCDTC_raw32_Inproc/1 -> UnitConverter364/1
  UnitConverter364/1 -> VOUTP_C3CCU1RCDTC_raw32/1  "VOUTP_C3CCU1RCDTC_raw32"
  VDDM_C3CCU1CSDTC_raw32/1 -> VDDM_C3CCU1CSDTC_raw32_Inproc/1  "VDDM_C3CCU1CSDTC_raw32"
  VDDM_C3CCU1CSDTC_raw32_Inproc/1 -> UnitConverter365/1
  UnitConverter365/1 -> VOUTP_C3CCU1CSDTC_raw32/1  "VOUTP_C3CCU1CSDTC_raw32"
  VDDM_C3CCU1LCDTC_raw32/1 -> VDDM_C3CCU1LCDTC_raw32_Inproc/1  "VDDM_C3CCU1LCDTC_raw32"
  VDDM_C3CCU1LCDTC_raw32_Inproc/1 -> UnitConverter366/1
  UnitConverter366/1 -> VOUTP_C3CCU1LCDTC_raw32/1  "VOUTP_C3CCU1LCDTC_raw32"
  VDDM_C3CCU2RCDTC_raw32/1 -> VDDM_C3CCU2RCDTC_raw32_Inproc/1  "VDDM_C3CCU2RCDTC_raw32"
  VDDM_C3CCU2RCDTC_raw32_Inproc/1 -> UnitConverter367/1
  UnitConverter367/1 -> VOUTP_C3CCU2RCDTC_raw32/1  "VOUTP_C3CCU2RCDTC_raw32"
  VDDM_C3CCU2CSDTC_raw32/1 -> VDDM_C3CCU2CSDTC_raw32_Inproc/1  "VDDM_C3CCU2CSDTC_raw32"
  VDDM_C3CCU2CSDTC_raw32_Inproc/1 -> UnitConverter368/1
  UnitConverter368/1 -> VOUTP_C3CCU2CSDTC_raw32/1  "VOUTP_C3CCU2CSDTC_raw32"
  VDDM_C3CCU2LCDTC_raw32/1 -> VDDM_C3CCU2LCDTC_raw32_Inproc/1  "VDDM_C3CCU2LCDTC_raw32"
  VDDM_C3CCU2LCDTC_raw32_Inproc/1 -> UnitConverter369/1
  UnitConverter369/1 -> VOUTP_C3CCU2LCDTC_raw32/1  "VOUTP_C3CCU2LCDTC_raw32"
  VDDM_C1ABM1RCDTC_raw32/1 -> VDDM_C1ABM1RCDTC_raw32_Inproc/1  "VDDM_C1ABM1RCDTC_raw32"
  VDDM_C1ABM1RCDTC_raw32_Inproc/1 -> UnitConverter370/1
  UnitConverter370/1 -> VOUTP_C1ABM1RCDTC_raw32/1  "VOUTP_C1ABM1RCDTC_raw32"
  VDDM_C1ABM1CSDTC_raw32/1 -> VDDM_C1ABM1CSDTC_raw32_Inproc/1  "VDDM_C1ABM1CSDTC_raw32"
  VDDM_C1ABM1CSDTC_raw32_Inproc/1 -> UnitConverter371/1
  UnitConverter371/1 -> VOUTP_C1ABM1CSDTC_raw32/1  "VOUTP_C1ABM1CSDTC_raw32"
  VDDM_C1ABM1LCDTC_raw32/1 -> VDDM_C1ABM1LCDTC_raw32_Inproc/1  "VDDM_C1ABM1LCDTC_raw32"
  VDDM_C1ABM1LCDTC_raw32_Inproc/1 -> UnitConverter372/1
  UnitConverter372/1 -> VOUTP_C1ABM1LCDTC_raw32/1  "VOUTP_C1ABM1LCDTC_raw32"
  VDDM_Lv1ErrDTC_raw32/1 -> VDDM_Lv1ErrDTC_raw32_Inproc/1  "VDDM_Lv1ErrDTC_raw32"
  VDDM_Lv1ErrDTC_raw32_Inproc/1 -> UnitConverter373/1
  UnitConverter373/1 -> VOUTP_Lv1ErrDTC_raw32/1  "VOUTP_Lv1ErrDTC_raw32"
  VDDM_Lv2ErrDTC_raw32/1 -> VDDM_Lv2ErrDTC_raw32_Inproc/1  "VDDM_Lv2ErrDTC_raw32"
  VDDM_Lv2ErrDTC_raw32_Inproc/1 -> UnitConverter374/1
  UnitConverter374/1 -> VOUTP_Lv2ErrDTC_raw32/1  "VOUTP_Lv2ErrDTC_raw32"
  VDDM_Lv3ErrDTC_raw32/1 -> VDDM_Lv3ErrDTC_raw32_Inproc/1  "VDDM_Lv3ErrDTC_raw32"
  VDDM_Lv3ErrDTC_raw32_Inproc/1 -> UnitConverter375/1
  UnitConverter375/1 -> VOUTP_Lv3ErrDTC_raw32/1  "VOUTP_Lv3ErrDTC_raw32"
  VDDM_Lv4ErrDTC_raw32/1 -> VDDM_Lv4ErrDTC_raw32_Inproc/1  "VDDM_Lv4ErrDTC_raw32"
  VDDM_Lv4ErrDTC_raw32_Inproc/1 -> UnitConverter376/1
  UnitConverter376/1 -> VOUTP_Lv4ErrDTC_raw32/1  "VOUTP_Lv4ErrDTC_raw32"
  VDDM_BrkSWErrDTC_raw32/1 -> VDDM_BrkSWErrDTC_raw32_Inproc/1  "VDDM_BrkSWErrDTC_raw32"
  VDDM_BrkSWErrDTC_raw32_Inproc/1 -> UnitConverter377/1
  UnitConverter377/1 -> VOUTP_BrkSWErrDTC_raw32/1  "VOUTP_BrkSWErrDTC_raw32"
  VDDM_BrkSWNoBacDTC_raw32/1 -> VDDM_BrkSWNoBacDTC_raw32_Inproc/1  "VDDM_BrkSWNoBacDTC_raw32"
  VDDM_BrkSWNoBacDTC_raw32_Inproc/1 -> UnitConverter378/1
  UnitConverter378/1 -> VOUTP_BrkSWNoBacDTC_raw32/1  "VOUTP_BrkSWNoBacDTC_raw32"
  VDDM_KeyAuthDTC_raw32/1 -> VDDM_KeyAuthDTC_raw32_Inproc/1  "VDDM_KeyAuthDTC_raw32"
  VDDM_KeyAuthDTC_raw32_Inproc/1 -> UnitConverter379/1
  UnitConverter379/1 -> VOUTP_KeyAuthDTC_raw32/1  "VOUTP_KeyAuthDTC_raw32"
  VDDM_ONtoRdyDTC_raw32/1 -> VDDM_ONtoRdyDTC_raw32_Inproc/1  "VDDM_ONtoRdyDTC_raw32"
  VDDM_ONtoRdyDTC_raw32_Inproc/1 -> UnitConverter380/1
  UnitConverter380/1 -> VOUTP_ONtoRdyDTC_raw32/1  "VOUTP_ONtoRdyDTC_raw32"
  VDDM_HVB4PreDTC_raw32/1 -> VDDM_HVB4PreDTC_raw32_Inproc/1  "VDDM_HVB4PreDTC_raw32"
  VDDM_HVB4PreDTC_raw32_Inproc/1 -> UnitConverter381/1
  UnitConverter381/1 -> VOUTP_HVB4PreDTC_raw32/1  "VOUTP_HVB4PreDTC_raw32"
  VDDM_MCU4PreDTC_raw32/1 -> VDDM_MCU4PreDTC_raw32_Inproc/1  "VDDM_MCU4PreDTC_raw32"
  VDDM_MCU4PreDTC_raw32_Inproc/1 -> UnitConverter382/1
  UnitConverter382/1 -> VOUTP_MCU4PreDTC_raw32/1  "VOUTP_MCU4PreDTC_raw32"
  VDDM_DCDC4PreDTC_raw32/1 -> VDDM_DCDC4PreDTC_raw32_Inproc/1  "VDDM_DCDC4PreDTC_raw32"
  VDDM_DCDC4PreDTC_raw32_Inproc/1 -> UnitConverter383/1
  UnitConverter383/1 -> VOUTP_DCDC4PreDTC_raw32/1  "VOUTP_DCDC4PreDTC_raw32"
  VDDM_HVRlyCloDTC_raw32/1 -> VDDM_HVRlyCloDTC_raw32_Inproc/1  "VDDM_HVRlyCloDTC_raw32"
  VDDM_HVRlyCloDTC_raw32_Inproc/1 -> UnitConverter384/1
  UnitConverter384/1 -> VOUTP_HVRlyCloDTC_raw32/1  "VOUTP_HVRlyCloDTC_raw32"
  VDDM_BMSRdyDTC_raw32/1 -> VDDM_BMSRdyDTC_raw32_Inproc/1  "VDDM_BMSRdyDTC_raw32"
  VDDM_BMSRdyDTC_raw32_Inproc/1 -> UnitConverter385/1
  UnitConverter385/1 -> VOUTP_BMSRdyDTC_raw32/1  "VOUTP_BMSRdyDTC_raw32"
  VDDM_DCDCEnaDTC_raw32/1 -> VDDM_DCDCEnaDTC_raw32_Inproc/1  "VDDM_DCDCEnaDTC_raw32"
  VDDM_DCDCEnaDTC_raw32_Inproc/1 -> UnitConverter386/1
  UnitConverter386/1 -> VOUTP_DCDCEnaDTC_raw32/1  "VOUTP_DCDCEnaDTC_raw32"
  VDDM_HiLvSaChkDTC_raw32/1 -> VDDM_HiLvSaChkDTC_raw32_Inproc/1  "VDDM_HiLvSaChkDTC_raw32"
  VDDM_HiLvSaChkDTC_raw32_Inproc/1 -> UnitConverter387/1
  UnitConverter387/1 -> VOUTP_HiLvSaChkDTC_raw32/1  "VOUTP_HiLvSaChkDTC_raw32"
  VDDM_MidLvSaChkDTC_raw32/1 -> VDDM_MidLvSaChkDTC_raw32_Inproc/1  "VDDM_MidLvSaChkDTC_raw32"
  VDDM_MidLvSaChkDTC_raw32_Inproc/1 -> UnitConverter388/1
  UnitConverter388/1 -> VOUTP_MidLvSaChkDTC_raw32/1  "VOUTP_MidLvSaChkDTC_raw32"
  VDDM_MCUDisDTC_raw32/1 -> VDDM_MCUDisDTC_raw32_Inproc/1  "VDDM_MCUDisDTC_raw32"
  VDDM_MCUDisDTC_raw32_Inproc/1 -> UnitConverter389/1
  UnitConverter389/1 -> VOUTP_MCUDisDTC_raw32/1  "VOUTP_MCUDisDTC_raw32"
  VDDM_DCDCDisDTC_raw32/1 -> VDDM_DCDCDisDTC_raw32_Inproc/1  "VDDM_DCDCDisDTC_raw32"
  VDDM_DCDCDisDTC_raw32_Inproc/1 -> UnitConverter390/1
  UnitConverter390/1 -> VOUTP_DCDCDisDTC_raw32/1  "VOUTP_DCDCDisDTC_raw32"
  VDDM_HVRlyOpDTC_raw32/1 -> VDDM_HVRlyOpDTC_raw32_Inproc/1  "VDDM_HVRlyOpDTC_raw32"
  VDDM_HVRlyOpDTC_raw32_Inproc/1 -> UnitConverter391/1
  UnitConverter391/1 -> VOUTP_HVRlyOpDTC_raw32/1  "VOUTP_HVRlyOpDTC_raw32"
  VDDM_MCUActDTC_raw32/1 -> VDDM_MCUActDTC_raw32_Inproc/1  "VDDM_MCUActDTC_raw32"
  VDDM_MCUActDTC_raw32_Inproc/1 -> UnitConverter392/1
  UnitConverter392/1 -> VOUTP_MCUActDTC_raw32/1  "VOUTP_MCUActDTC_raw32"
  VDDM_OBC4PreDTC_raw32/1 -> VDDM_OBC4PreDTC_raw32_Inproc/1  "VDDM_OBC4PreDTC_raw32"
  VDDM_OBC4PreDTC_raw32_Inproc/1 -> UnitConverter393/1
  UnitConverter393/1 -> VOUTP_OBC4PreDTC_raw32/1  "VOUTP_OBC4PreDTC_raw32"
  VDDM_IniLVLoDTC_raw32/1 -> VDDM_IniLVLoDTC_raw32_Inproc/1  "VDDM_IniLVLoDTC_raw32"
  VDDM_IniLVLoDTC_raw32_Inproc/1 -> UnitConverter394/1
  UnitConverter394/1 -> VOUTP_IniLVLoDTC_raw32/1  "VOUTP_IniLVLoDTC_raw32"
  VDDM_LVSupLoDTC_raw32/1 -> VDDM_LVSupLoDTC_raw32_Inproc/1  "VDDM_LVSupLoDTC_raw32"
  VDDM_LVSupLoDTC_raw32_Inproc/1 -> UnitConverter395/1
  UnitConverter395/1 -> VOUTP_LVSupLoDTC_raw32/1  "VOUTP_LVSupLoDTC_raw32"
  VDDM_LVSupHiDTC_raw32/1 -> VDDM_LVSupHiDTC_raw32_Inproc/1  "VDDM_LVSupHiDTC_raw32"
  VDDM_LVSupHiDTC_raw32_Inproc/1 -> UnitConverter396/1
  UnitConverter396/1 -> VOUTP_LVSupHiDTC_raw32/1  "VOUTP_LVSupHiDTC_raw32"
  VDDM_DrStSWDTC_raw32/1 -> VDDM_DrStSWDTC_raw32_Inproc/1  "VDDM_DrStSWDTC_raw32"
  VDDM_DrStSWDTC_raw32_Inproc/1 -> UnitConverter397/1
  UnitConverter397/1 -> VOUTP_DrStSWDTC_raw32/1  "VOUTP_DrStSWDTC_raw32"
  VDDM_FLDoorSWDTC_raw32/1 -> VDDM_FLDoorSWDTC_raw32_Inproc/1  "VDDM_FLDoorSWDTC_raw32"
  VDDM_FLDoorSWDTC_raw32_Inproc/1 -> UnitConverter398/1
  UnitConverter398/1 -> VOUTP_FLDoorSWDTC_raw32/1  "VOUTP_FLDoorSWDTC_raw32"
  VDDM_RLDoorSWDTC_raw32/1 -> VDDM_RLDoorSWDTC_raw32_Inproc/1  "VDDM_RLDoorSWDTC_raw32"
  VDDM_RLDoorSWDTC_raw32_Inproc/1 -> UnitConverter399/1
  UnitConverter399/1 -> VOUTP_RLDoorSWDTC_raw32/1  "VOUTP_RLDoorSWDTC_raw32"
  VDDM_FRDoorSWDTC_raw32/1 -> VDDM_FRDoorSWDTC_raw32_Inproc/1  "VDDM_FRDoorSWDTC_raw32"
  VDDM_FRDoorSWDTC_raw32_Inproc/1 -> UnitConverter400/1
  UnitConverter400/1 -> VOUTP_FRDoorSWDTC_raw32/1  "VOUTP_FRDoorSWDTC_raw32"
  VDDM_RRDoorSWDTC_raw32/1 -> VDDM_RRDoorSWDTC_raw32_Inproc/1  "VDDM_RRDoorSWDTC_raw32"
  VDDM_RRDoorSWDTC_raw32_Inproc/1 -> UnitConverter401/1
  UnitConverter401/1 -> VOUTP_RRDoorSWDTC_raw32/1  "VOUTP_RRDoorSWDTC_raw32"
  VDDM_HoodSWDTC_raw32/1 -> VDDM_HoodSWDTC_raw32_Inproc/1  "VDDM_HoodSWDTC_raw32"
  VDDM_HoodSWDTC_raw32_Inproc/1 -> UnitConverter402/1
  UnitConverter402/1 -> VOUTP_HoodSWDTC_raw32/1  "VOUTP_HoodSWDTC_raw32"
  VDDM_TailgaSWDTC_raw32/1 -> VDDM_TailgaSWDTC_raw32_Inproc/1  "VDDM_TailgaSWDTC_raw32"
  VDDM_TailgaSWDTC_raw32_Inproc/1 -> UnitConverter403/1
  UnitConverter403/1 -> VOUTP_TailgaSWDTC_raw32/1  "VOUTP_TailgaSWDTC_raw32"
  VDDM_EDriveSysErrVCUErr_flg/1 -> VDDM_EDriveSysErrVCUErr_flg_Inproc/1  "VDDM_EDriveSysErrVCUErr_flg"
  VDDM_EDriveSysErrVCUErr_flg_Inproc/1 -> UnitConverter404/1
  UnitConverter404/1 -> VOUTP_EDriveSysErrVCUErr_flg/1  "VOUTP_EDriveSysErrVCUErr_flg"
  VDDM_VehMalfunLevel_enum/1 -> VDDM_VehMalfunLevel_enum_Inproc/1  "VDDM_VehMalfunLevel_enum"
  VDDM_VehMalfunLevel_enum_Inproc/1 -> UnitConverter405/1
  UnitConverter405/1 -> VOUTP_VehMalfunLevel_enum/1  "VOUTP_VehMalfunLevel_enum"
  VDDM_APS1SigOoRDTC_raw32/1 -> VDDM_APS1SigOoRDTC_raw32_Inproc/1  "VDDM_APS1SigOoRDTC_raw32"
  VDDM_APS1SigOoRDTC_raw32_Inproc/1 -> UnitConverter406/1
  UnitConverter406/1 -> VOUTP_APS1SigOoRDTC_raw32/1  "VOUTP_APS1SigOoRDTC_raw32"
  VDDM_APS2SigOoRDTC_raw32/1 -> VDDM_APS2SigOoRDTC_raw32_Inproc/1  "VDDM_APS2SigOoRDTC_raw32"
  VDDM_APS2SigOoRDTC_raw32_Inproc/1 -> UnitConverter407/1
  UnitConverter407/1 -> VOUTP_APS2SigOoRDTC_raw32/1  "VOUTP_APS2SigOoRDTC_raw32"
  VDDM_APSCorrErrDTC_raw32/1 -> VDDM_APSCorrErrDTC_raw32_Inproc/1  "VDDM_APSCorrErrDTC_raw32"
  VDDM_APSCorrErrDTC_raw32_Inproc/1 -> UnitConverter408/1
  UnitConverter408/1 -> VOUTP_APSCorrErrDTC_raw32/1  "VOUTP_APSCorrErrDTC_raw32"
  VDDM_MCUF1NoComDTC_raw32/1 -> VDDM_MCUF1NoComDTC_raw32_Inproc/1  "VDDM_MCUF1NoComDTC_raw32"
  VDDM_MCUF1NoComDTC_raw32_Inproc/1 -> UnitConverter409/1
  UnitConverter409/1 -> VOUTP_MCUF1NoComDTC_raw32/1  "VOUTP_MCUF1NoComDTC_raw32"
  VDDM_MCUR1NoComDTC_raw32/1 -> VDDM_MCUR1NoComDTC_raw32_Inproc/1  "VDDM_MCUR1NoComDTC_raw32"
  VDDM_MCUR1NoComDTC_raw32_Inproc/1 -> UnitConverter410/1
  UnitConverter410/1 -> VOUTP_MCUR1NoComDTC_raw32/1  "VOUTP_MCUR1NoComDTC_raw32"
  VDDM_Shifter1NoComDTC_raw32/1 -> VDDM_Shifter1NoComDTC_raw32_Inproc/1  "VDDM_Shifter1NoComDTC_raw32"
  VDDM_Shifter1NoComDTC_raw32_Inproc/1 -> UnitConverter411/1
  UnitConverter411/1 -> VOUTP_Shifter1NoComDTC_raw32/1  "VOUTP_Shifter1NoComDTC_raw32"
  VDDM_ESC7NoComDTC_raw32/1 -> VDDM_ESC7NoComDTC_raw32_Inproc/1  "VDDM_ESC7NoComDTC_raw32"
  VDDM_ESC7NoComDTC_raw32_Inproc/1 -> UnitConverter412/1
  UnitConverter412/1 -> VOUTP_ESC7NoComDTC_raw32/1  "VOUTP_ESC7NoComDTC_raw32"
  VDDM_ESC1NoComDTC_raw32/1 -> VDDM_ESC1NoComDTC_raw32_Inproc/1  "VDDM_ESC1NoComDTC_raw32"
  VDDM_ESC1NoComDTC_raw32_Inproc/1 -> UnitConverter413/1
  UnitConverter413/1 -> VOUTP_ESC1NoComDTC_raw32/1  "VOUTP_ESC1NoComDTC_raw32"
  VDDM_ESC5NoComDTC_raw32/1 -> VDDM_ESC5NoComDTC_raw32_Inproc/1  "VDDM_ESC5NoComDTC_raw32"
  VDDM_ESC5NoComDTC_raw32_Inproc/1 -> UnitConverter414/1
  UnitConverter414/1 -> VOUTP_ESC5NoComDTC_raw32/1  "VOUTP_ESC5NoComDTC_raw32"
  VDDM_EnterNewOperCyc_flg/1 -> VDDM_EnterNewOperCyc_flg_Inproc/1  "VDDM_EnterNewOperCyc_flg"
  VDDM_EnterNewOperCyc_flg_Inproc/1 -> UnitConverter415/1
  UnitConverter415/1 -> VOUTP_EnterNewOperCyc_flg/1  "VOUTP_EnterNewOperCyc_flg"
  VDDM_DiagHCrashDTC_raw32/1 -> VDDM_DiagHCrashDTC_raw32_Inproc/1  "VDDM_DiagHCrashDTC_raw32"
  VDDM_DiagHCrashDTC_raw32_Inproc/1 -> UnitConverter416/1
  UnitConverter416/1 -> VOUTP_DiagHCrashDTC_raw32/1  "VOUTP_DiagHCrashDTC_raw32"
  VDDM_DiagFLTSDTC_raw32/1 -> VDDM_DiagFLTSDTC_raw32_Inproc/1  "VDDM_DiagFLTSDTC_raw32"
  VDDM_DiagFLTSDTC_raw32_Inproc/1 -> UnitConverter417/1
  UnitConverter417/1 -> VOUTP_DiagFLTSDTC_raw32/1  "VOUTP_DiagFLTSDTC_raw32"
  VDDM_DiagFRTSDTC_raw32/1 -> VDDM_DiagFRTSDTC_raw32_Inproc/1  "VDDM_DiagFRTSDTC_raw32"
  VDDM_DiagFRTSDTC_raw32_Inproc/1 -> UnitConverter418/1
  UnitConverter418/1 -> VOUTP_DiagFRTSDTC_raw32/1  "VOUTP_DiagFRTSDTC_raw32"
  VDDM_DiagRLTSDTC_raw32/1 -> VDDM_DiagRLTSDTC_raw32_Inproc/1  "VDDM_DiagRLTSDTC_raw32"
  VDDM_DiagRLTSDTC_raw32_Inproc/1 -> UnitConverter419/1
  UnitConverter419/1 -> VOUTP_DiagRLTSDTC_raw32/1  "VOUTP_DiagRLTSDTC_raw32"
  VDDM_DiagRRTSDTC_raw32/1 -> VDDM_DiagRRTSDTC_raw32_Inproc/1  "VDDM_DiagRRTSDTC_raw32"
  VDDM_DiagRRTSDTC_raw32_Inproc/1 -> UnitConverter420/1
  UnitConverter420/1 -> VOUTP_DiagRRTSDTC_raw32/1  "VOUTP_DiagRRTSDTC_raw32"
  VDDM_FCLUSSDTC_raw32/1 -> VDDM_FCLUSSDTC_raw32_Inproc/1  "VDDM_FCLUSSDTC_raw32"
  VDDM_FCLUSSDTC_raw32_Inproc/1 -> UnitConverter421/1
  UnitConverter421/1 -> VOUTP_FCLUSSDTC_raw32/1  "VOUTP_FCLUSSDTC_raw32"
  VDDM_FMLUSSDTC_raw32/1 -> VDDM_FMLUSSDTC_raw32_Inproc/1  "VDDM_FMLUSSDTC_raw32"
  VDDM_FMLUSSDTC_raw32_Inproc/1 -> UnitConverter422/1
  UnitConverter422/1 -> VOUTP_FMLUSSDTC_raw32/1  "VOUTP_FMLUSSDTC_raw32"
  VDDM_FMRUSSDTC_raw32/1 -> VDDM_FMRUSSDTC_raw32_Inproc/1  "VDDM_FMRUSSDTC_raw32"
  VDDM_FMRUSSDTC_raw32_Inproc/1 -> UnitConverter423/1
  UnitConverter423/1 -> VOUTP_FMRUSSDTC_raw32/1  "VOUTP_FMRUSSDTC_raw32"
  VDDM_FCRUSSDTC_raw32/1 -> VDDM_FCRUSSDTC_raw32_Inproc/1  "VDDM_FCRUSSDTC_raw32"
  VDDM_FCRUSSDTC_raw32_Inproc/1 -> UnitConverter424/1
  UnitConverter424/1 -> VOUTP_FCRUSSDTC_raw32/1  "VOUTP_FCRUSSDTC_raw32"
  VDDM_RCLUSSDTC_raw32/1 -> VDDM_RCLUSSDTC_raw32_Inproc/1  "VDDM_RCLUSSDTC_raw32"
  VDDM_RCLUSSDTC_raw32_Inproc/1 -> UnitConverter425/1
  UnitConverter425/1 -> VOUTP_RCLUSSDTC_raw32/1  "VOUTP_RCLUSSDTC_raw32"
  VDDM_RMLUSSDTC_raw32/1 -> VDDM_RMLUSSDTC_raw32_Inproc/1  "VDDM_RMLUSSDTC_raw32"
  VDDM_RMLUSSDTC_raw32_Inproc/1 -> UnitConverter426/1
  UnitConverter426/1 -> VOUTP_RMLUSSDTC_raw32/1  "VOUTP_RMLUSSDTC_raw32"
  VDDM_RMRUSSDTC_raw32/1 -> VDDM_RMRUSSDTC_raw32_Inproc/1  "VDDM_RMRUSSDTC_raw32"
  VDDM_RMRUSSDTC_raw32_Inproc/1 -> UnitConverter427/1
  UnitConverter427/1 -> VOUTP_RMRUSSDTC_raw32/1  "VOUTP_RMRUSSDTC_raw32"
  VDDM_RCRUSSDTC_raw32/1 -> VDDM_RCRUSSDTC_raw32_Inproc/1  "VDDM_RCRUSSDTC_raw32"
  VDDM_RCRUSSDTC_raw32_Inproc/1 -> UnitConverter428/1
  UnitConverter428/1 -> VOUTP_RCRUSSDTC_raw32/1  "VOUTP_RCRUSSDTC_raw32"
  VDDM_FLLUSSDTC_raw32/1 -> VDDM_FLLUSSDTC_raw32_Inproc/1  "VDDM_FLLUSSDTC_raw32"
  VDDM_FLLUSSDTC_raw32_Inproc/1 -> UnitConverter429/1
  UnitConverter429/1 -> VOUTP_FLLUSSDTC_raw32/1  "VOUTP_FLLUSSDTC_raw32"
  VDDM_FLRUSSDTC_raw32/1 -> VDDM_FLRUSSDTC_raw32_Inproc/1  "VDDM_FLRUSSDTC_raw32"
  VDDM_FLRUSSDTC_raw32_Inproc/1 -> UnitConverter430/1
  UnitConverter430/1 -> VOUTP_FLRUSSDTC_raw32/1  "VOUTP_FLRUSSDTC_raw32"
  VDDM_RLLUSSDTC_raw32/1 -> VDDM_RLLUSSDTC_raw32_Inproc/1  "VDDM_RLLUSSDTC_raw32"
  VDDM_RLLUSSDTC_raw32_Inproc/1 -> UnitConverter431/1
  UnitConverter431/1 -> VOUTP_RLLUSSDTC_raw32/1  "VOUTP_RLLUSSDTC_raw32"
  VDDM_RLRUSSDTC_raw32/1 -> VDDM_RLRUSSDTC_raw32_Inproc/1  "VDDM_RLRUSSDTC_raw32"
  VDDM_RLRUSSDTC_raw32_Inproc/1 -> UnitConverter432/1
  UnitConverter432/1 -> VOUTP_RLRUSSDTC_raw32/1  "VOUTP_RLRUSSDTC_raw32"
  VDDM_FCM2NoComDTC_raw32/1 -> VDDM_FCM2NoComDTC_raw32_Inproc/1  "VDDM_FCM2NoComDTC_raw32"
  VDDM_FCM2NoComDTC_raw32_Inproc/1 -> UnitConverter433/1
  UnitConverter433/1 -> VOUTP_FCM2NoComDTC_raw32/1  "VOUTP_FCM2NoComDTC_raw32"
  VDDM_FCM2RCErrDTC_raw32/1 -> VDDM_FCM2RCErrDTC_raw32_Inproc/1  "VDDM_FCM2RCErrDTC_raw32"
  VDDM_FCM2RCErrDTC_raw32_Inproc/1 -> UnitConverter434/1
  UnitConverter434/1 -> VOUTP_FCM2RCErrDTC_raw32/1  "VOUTP_FCM2RCErrDTC_raw32"
  VDDM_FCM2CSErrDTC_raw32/1 -> VDDM_FCM2CSErrDTC_raw32_Inproc/1  "VDDM_FCM2CSErrDTC_raw32"
  VDDM_FCM2CSErrDTC_raw32_Inproc/1 -> UnitConverter435/1
  UnitConverter435/1 -> VOUTP_FCM2CSErrDTC_raw32/1  "VOUTP_FCM2CSErrDTC_raw32"
  VDDM_FCM3NoComDTC_raw32/1 -> VDDM_FCM3NoComDTC_raw32_Inproc/1  "VDDM_FCM3NoComDTC_raw32"
  VDDM_FCM3NoComDTC_raw32_Inproc/1 -> UnitConverter436/1
  UnitConverter436/1 -> VOUTP_FCM3NoComDTC_raw32/1  "VOUTP_FCM3NoComDTC_raw32"
  VDDM_FCM3RCErrDTC_raw32/1 -> VDDM_FCM3RCErrDTC_raw32_Inproc/1  "VDDM_FCM3RCErrDTC_raw32"
  VDDM_FCM3RCErrDTC_raw32_Inproc/1 -> UnitConverter437/1
  UnitConverter437/1 -> VOUTP_FCM3RCErrDTC_raw32/1  "VOUTP_FCM3RCErrDTC_raw32"
  VDDM_FCM3CSErrDTC_raw32/1 -> VDDM_FCM3CSErrDTC_raw32_Inproc/1  "VDDM_FCM3CSErrDTC_raw32"
  VDDM_FCM3CSErrDTC_raw32_Inproc/1 -> UnitConverter438/1
  UnitConverter438/1 -> VOUTP_FCM3CSErrDTC_raw32/1  "VOUTP_FCM3CSErrDTC_raw32"
  VDDM_FCM4NoComDTC_raw32/1 -> VDDM_FCM4NoComDTC_raw32_Inproc/1  "VDDM_FCM4NoComDTC_raw32"
  VDDM_FCM4NoComDTC_raw32_Inproc/1 -> UnitConverter439/1
  UnitConverter439/1 -> VOUTP_FCM4NoComDTC_raw32/1  "VOUTP_FCM4NoComDTC_raw32"
  VDDM_FCM4CSErrDTC_raw32/1 -> VDDM_FCM4CSErrDTC_raw32_Inproc/1  "VDDM_FCM4CSErrDTC_raw32"
  VDDM_FCM4CSErrDTC_raw32_Inproc/1 -> UnitConverter440/1
  UnitConverter440/1 -> VOUTP_FCM4CSErrDTC_raw32/1  "VOUTP_FCM4CSErrDTC_raw32"
  VDDM_FCM5NoComDTC_raw32/1 -> VDDM_FCM5NoComDTC_raw32_Inproc/1  "VDDM_FCM5NoComDTC_raw32"
  VDDM_FCM5NoComDTC_raw32_Inproc/1 -> UnitConverter441/1
  UnitConverter441/1 -> VOUTP_FCM5NoComDTC_raw32/1  "VOUTP_FCM5NoComDTC_raw32"
  VDDM_FCM5CSErrDTC_raw32/1 -> VDDM_FCM5CSErrDTC_raw32_Inproc/1  "VDDM_FCM5CSErrDTC_raw32"
  VDDM_FCM5CSErrDTC_raw32_Inproc/1 -> UnitConverter442/1
  UnitConverter442/1 -> VOUTP_FCM5CSErrDTC_raw32/1  "VOUTP_FCM5CSErrDTC_raw32"
  VDDM_ZoneSCPNoComDTC_raw32/1 -> VDDM_ZoneSCPNoComDTC_raw32_Inproc/1  "VDDM_ZoneSCPNoComDTC_raw32"
  VDDM_ZoneSCPNoComDTC_raw32_Inproc/1 -> UnitConverter443/1
  UnitConverter443/1 -> VOUTP_ZoneSCPNoComDTC_raw32/1  "VOUTP_ZoneSCPNoComDTC_raw32"
  VDDM_BMSSigErrDetDTC_raw32/1 -> VDDM_BMSSigErrDetDTC_raw32_Inproc/1  "VDDM_BMSSigErrDetDTC_raw32"
  VDDM_BMSSigErrDetDTC_raw32_Inproc/1 -> UnitConverter444/1
  UnitConverter444/1 -> VOUTP_BMSSigErrDetDTC_raw32/1  "VOUTP_BMSSigErrDetDTC_raw32"
  VDDM_FCMACCSigErrDetDTC_raw32/1 -> VDDM_FCMACCSigErrDetDTC_raw32_Inproc/1  "VDDM_FCMACCSigErrDetDTC_raw32"
  VDDM_FCMACCSigErrDetDTC_raw32_Inproc/1 -> UnitConverter445/1
  UnitConverter445/1 -> VOUTP_FCMACCSigErrDetDTC_raw32/1  "VOUTP_FCMACCSigErrDetDTC_raw32"
  VDDM_FrMCUSigErrDetDTC_raw32/1 -> VDDM_FrMCUSigErrDetDTC_raw32_Inproc/1  "VDDM_FrMCUSigErrDetDTC_raw32"
  VDDM_FrMCUSigErrDetDTC_raw32_Inproc/1 -> UnitConverter446/1
  UnitConverter446/1 -> VOUTP_FrMCUSigErrDetDTC_raw32/1  "VOUTP_FrMCUSigErrDetDTC_raw32"
  VDDM_RrMCUSigErrDetDTC_raw32/1 -> VDDM_RrMCUSigErrDetDTC_raw32_Inproc/1  "VDDM_RrMCUSigErrDetDTC_raw32"
  VDDM_RrMCUSigErrDetDTC_raw32_Inproc/1 -> UnitConverter447/1
  UnitConverter447/1 -> VOUTP_RrMCUSigErrDetDTC_raw32/1  "VOUTP_RrMCUSigErrDetDTC_raw32"
  VDDM_CCUSigErrDetDTC_raw32/1 -> VDDM_CCUSigErrDetDTC_raw32_Inproc/1  "VDDM_CCUSigErrDetDTC_raw32"
  VDDM_CCUSigErrDetDTC_raw32_Inproc/1 -> UnitConverter448/1
  UnitConverter448/1 -> VOUTP_CCUSigErrDetDTC_raw32/1  "VOUTP_CCUSigErrDetDTC_raw32"
  VDDM_ACCAccelCmdErrDetDTC_raw32/1 -> VDDM_ACCAccelCmdErrDetDTC_raw32_Inproc/1  "VDDM_ACCAccelCmdErrDetDTC_raw32"
  VDDM_ACCAccelCmdErrDetDTC_raw32_Inproc/1 -> UnitConverter449/1
  UnitConverter449/1 -> VOUTP_ACCAccelCmdErrDetDTC_raw32/1  "VOUTP_ACCAccelCmdErrDetDTC_raw32"
  VDDM_ACCMalfuncDetDTC_raw32/1 -> VDDM_ACCMalfuncDetDTC_raw32_Inproc/1  "VDDM_ACCMalfuncDetDTC_raw32"
  VDDM_ACCMalfuncDetDTC_raw32_Inproc/1 -> UnitConverter450/1
  UnitConverter450/1 -> VOUTP_ACCMalfuncDetDTC_raw32/1  "VOUTP_ACCMalfuncDetDTC_raw32"
  VDDM_CCMalfuncDetDTC_raw32/1 -> VDDM_CCMalfuncDetDTC_raw32_Inproc/1  "VDDM_CCMalfuncDetDTC_raw32"
  VDDM_CCMalfuncDetDTC_raw32_Inproc/1 -> UnitConverter451/1
  UnitConverter451/1 -> VOUTP_CCMalfuncDetDTC_raw32/1  "VOUTP_CCMalfuncDetDTC_raw32"
  VDDM_MSAMalfuncDetDTC_raw32/1 -> VDDM_MSAMalfuncDetDTC_raw32_Inproc/1  "VDDM_MSAMalfuncDetDTC_raw32"
  VDDM_MSAMalfuncDetDTC_raw32_Inproc/1 -> UnitConverter452/1
  UnitConverter452/1 -> VOUTP_MSAMalfuncDetDTC_raw32/1  "VOUTP_MSAMalfuncDetDTC_raw32"
  VDDM_ISAMalfuncDetDTC_raw32/1 -> VDDM_ISAMalfuncDetDTC_raw32_Inproc/1  "VDDM_ISAMalfuncDetDTC_raw32"
  VDDM_ISAMalfuncDetDTC_raw32_Inproc/1 -> UnitConverter453/1
  UnitConverter453/1 -> VOUTP_ISAMalfuncDetDTC_raw32/1  "VOUTP_ISAMalfuncDetDTC_raw32"
  VDDM_MCUF1RCErrDTC_raw32/1 -> VDDM_MCUF1RCErrDTC_raw32_Inproc/1  "VDDM_MCUF1RCErrDTC_raw32"
  VDDM_MCUF1RCErrDTC_raw32_Inproc/1 -> UnitConverter454/1
  UnitConverter454/1 -> VOUTP_MCUF1RCErrDTC_raw32/1  "VOUTP_MCUF1RCErrDTC_raw32"
  VDDM_MCUR1RCErrDTC_raw32/1 -> VDDM_MCUR1RCErrDTC_raw32_Inproc/1  "VDDM_MCUR1RCErrDTC_raw32"
  VDDM_MCUR1RCErrDTC_raw32_Inproc/1 -> UnitConverter455/1
  UnitConverter455/1 -> VOUTP_MCUR1RCErrDTC_raw32/1  "VOUTP_MCUR1RCErrDTC_raw32"
  VDDM_MCUF1CSErrDTC_raw32/1 -> VDDM_MCUF1CSErrDTC_raw32_Inproc/1  "VDDM_MCUF1CSErrDTC_raw32"
  VDDM_MCUF1CSErrDTC_raw32_Inproc/1 -> UnitConverter456/1
  UnitConverter456/1 -> VOUTP_MCUF1CSErrDTC_raw32/1  "VOUTP_MCUF1CSErrDTC_raw32"
  VDDM_MCUR1CSErrDTC_raw32/1 -> VDDM_MCUR1CSErrDTC_raw32_Inproc/1  "VDDM_MCUR1CSErrDTC_raw32"
  VDDM_MCUR1CSErrDTC_raw32_Inproc/1 -> UnitConverter457/1
  UnitConverter457/1 -> VOUTP_MCUR1CSErrDTC_raw32/1  "VOUTP_MCUR1CSErrDTC_raw32"
  VDDM_Shifter1RCErrDTC_raw32/1 -> VDDM_Shifter1RCErrDTC_raw32_Inproc/1  "VDDM_Shifter1RCErrDTC_raw32"
  VDDM_Shifter1RCErrDTC_raw32_Inproc/1 -> UnitConverter458/1
  UnitConverter458/1 -> VOUTP_Shifter1RCErrDTC_raw32/1  "VOUTP_Shifter1RCErrDTC_raw32"
  VDDM_Shifter1CSErrDTC_raw32/1 -> VDDM_Shifter1CSErrDTC_raw32_Inproc/1  "VDDM_Shifter1CSErrDTC_raw32"
  VDDM_Shifter1CSErrDTC_raw32_Inproc/1 -> UnitConverter459/1
  UnitConverter459/1 -> VOUTP_Shifter1CSErrDTC_raw32/1  "VOUTP_Shifter1CSErrDTC_raw32"
  VDDM_ESC7RCErrDTC_raw32/1 -> VDDM_ESC7RCErrDTC_raw32_Inproc/1  "VDDM_ESC7RCErrDTC_raw32"
  VDDM_ESC7RCErrDTC_raw32_Inproc/1 -> UnitConverter460/1
  UnitConverter460/1 -> VOUTP_ESC7RCErrDTC_raw32/1  "VOUTP_ESC7RCErrDTC_raw32"
  VDDM_ESC7CSErrDTC_raw32/1 -> VDDM_ESC7CSErrDTC_raw32_Inproc/1  "VDDM_ESC7CSErrDTC_raw32"
  VDDM_ESC7CSErrDTC_raw32_Inproc/1 -> UnitConverter461/1
  UnitConverter461/1 -> VOUTP_ESC7CSErrDTC_raw32/1  "VOUTP_ESC7CSErrDTC_raw32"
  VDDM_ESC1RCErrDTC_raw32/1 -> VDDM_ESC1RCErrDTC_raw32_Inproc/1  "VDDM_ESC1RCErrDTC_raw32"
  VDDM_ESC1RCErrDTC_raw32_Inproc/1 -> UnitConverter462/1
  UnitConverter462/1 -> VOUTP_ESC1RCErrDTC_raw32/1  "VOUTP_ESC1RCErrDTC_raw32"
  VDDM_ESC1CSErrDTC_raw32/1 -> VDDM_ESC1CSErrDTC_raw32_Inproc/1  "VDDM_ESC1CSErrDTC_raw32"
  VDDM_ESC1CSErrDTC_raw32_Inproc/1 -> UnitConverter463/1
  UnitConverter463/1 -> VOUTP_ESC1CSErrDTC_raw32/1  "VOUTP_ESC1CSErrDTC_raw32"
  VDDM_ESC5RCErrDTC_raw32/1 -> VDDM_ESC5RCErrDTC_raw32_Inproc/1  "VDDM_ESC5RCErrDTC_raw32"
  VDDM_ESC5RCErrDTC_raw32_Inproc/1 -> UnitConverter464/1
  UnitConverter464/1 -> VOUTP_ESC5RCErrDTC_raw32/1  "VOUTP_ESC5RCErrDTC_raw32"
  VDDM_ESC5CSErrDTC_raw32/1 -> VDDM_ESC5CSErrDTC_raw32_Inproc/1  "VDDM_ESC5CSErrDTC_raw32"
  VDDM_ESC5CSErrDTC_raw32_Inproc/1 -> UnitConverter465/1
  UnitConverter465/1 -> VOUTP_ESC5CSErrDTC_raw32/1  "VOUTP_ESC5CSErrDTC_raw32"
  VDDM_FrMCUTqErrDTC_raw32/1 -> VDDM_FrMCUTqErrDTC_raw32_Inproc/1  "VDDM_FrMCUTqErrDTC_raw32"
  VDDM_FrMCUTqErrDTC_raw32_Inproc/1 -> UnitConverter466/1
  UnitConverter466/1 -> VOUTP_FrMCUTqErrDTC_raw32/1  "VOUTP_FrMCUTqErrDTC_raw32"
  VDDM_RrMCUTqErrDTC_raw32/1 -> VDDM_RrMCUTqErrDTC_raw32_Inproc/1  "VDDM_RrMCUTqErrDTC_raw32"
  VDDM_RrMCUTqErrDTC_raw32_Inproc/1 -> UnitConverter467/1
  UnitConverter467/1 -> VOUTP_RrMCUTqErrDTC_raw32/1  "VOUTP_RrMCUTqErrDTC_raw32"
  VDDM_LFBatwarnDTC_raw32/1 -> VDDM_LFBatwarnDTC_raw32_Inproc/1  "VDDM_LFBatwarnDTC_raw32"
  VDDM_LFBatwarnDTC_raw32_Inproc/1 -> UnitConverter468/1
  UnitConverter468/1 -> VOUTP_LFBatwarnDTC_raw32/1  "VOUTP_LFBatwarnDTC_raw32"
  VDDM_RFBatwarnDTC_raw32/1 -> VDDM_RFBatwarnDTC_raw32_Inproc/1  "VDDM_RFBatwarnDTC_raw32"
  VDDM_RFBatwarnDTC_raw32_Inproc/1 -> UnitConverter469/1
  UnitConverter469/1 -> VOUTP_RFBatwarnDTC_raw32/1  "VOUTP_RFBatwarnDTC_raw32"
  VDDM_LRBatwarnDTC_raw32/1 -> VDDM_LRBatwarnDTC_raw32_Inproc/1  "VDDM_LRBatwarnDTC_raw32"
  VDDM_LRBatwarnDTC_raw32_Inproc/1 -> UnitConverter470/1
  UnitConverter470/1 -> VOUTP_LRBatwarnDTC_raw32/1  "VOUTP_LRBatwarnDTC_raw32"
  VDDM_RRBatwarnDTC_raw32/1 -> VDDM_RRBatwarnDTC_raw32_Inproc/1  "VDDM_RRBatwarnDTC_raw32"
  VDDM_RRBatwarnDTC_raw32_Inproc/1 -> UnitConverter471/1
  UnitConverter471/1 -> VOUTP_RRBatwarnDTC_raw32/1  "VOUTP_RRBatwarnDTC_raw32"
  VDDM_LFPressIndiDTC_raw32/1 -> VDDM_LFPressIndiDTC_raw32_Inproc/1  "VDDM_LFPressIndiDTC_raw32"
  VDDM_LFPressIndiDTC_raw32_Inproc/1 -> UnitConverter472/1
  UnitConverter472/1 -> VOUTP_LFPressIndiDTC_raw32/1  "VOUTP_LFPressIndiDTC_raw32"
  VDDM_RFPressIndiDTC_raw32/1 -> VDDM_RFPressIndiDTC_raw32_Inproc/1  "VDDM_RFPressIndiDTC_raw32"
  VDDM_RFPressIndiDTC_raw32_Inproc/1 -> UnitConverter473/1
  UnitConverter473/1 -> VOUTP_RFPressIndiDTC_raw32/1  "VOUTP_RFPressIndiDTC_raw32"
  VDDM_LRPressIndiDTC_raw32/1 -> VDDM_LRPressIndiDTC_raw32_Inproc/1  "VDDM_LRPressIndiDTC_raw32"
  VDDM_LRPressIndiDTC_raw32_Inproc/1 -> UnitConverter474/1
  UnitConverter474/1 -> VOUTP_LRPressIndiDTC_raw32/1  "VOUTP_LRPressIndiDTC_raw32"
  VDDM_RRPressIndiDTC_raw32/1 -> VDDM_RRPressIndiDTC_raw32_Inproc/1  "VDDM_RRPressIndiDTC_raw32"
  VDDM_RRPressIndiDTC_raw32_Inproc/1 -> UnitConverter475/1
  UnitConverter475/1 -> VOUTP_RRPressIndiDTC_raw32/1  "VOUTP_RRPressIndiDTC_raw32"
  VDDM_LFWheelTmpHighDTC_raw32/1 -> VDDM_LFWheelTmpHighDTC_raw32_Inproc/1  "VDDM_LFWheelTmpHighDTC_raw32"
  VDDM_LFWheelTmpHighDTC_raw32_Inproc/1 -> UnitConverter476/1
  UnitConverter476/1 -> VOUTP_LFWheelTmpHighDTC_raw32/1  "VOUTP_LFWheelTmpHighDTC_raw32"
  VDDM_RFWheelTmpHighDTC_raw32/1 -> VDDM_RFWheelTmpHighDTC_raw32_Inproc/1  "VDDM_RFWheelTmpHighDTC_raw32"
  VDDM_RFWheelTmpHighDTC_raw32_Inproc/1 -> UnitConverter477/1
  UnitConverter477/1 -> VOUTP_RFWheelTmpHighDTC_raw32/1  "VOUTP_RFWheelTmpHighDTC_raw32"
  VDDM_LRWheelTmpHighDTC_raw32/1 -> VDDM_LRWheelTmpHighDTC_raw32_Inproc/1  "VDDM_LRWheelTmpHighDTC_raw32"
  VDDM_LRWheelTmpHighDTC_raw32_Inproc/1 -> UnitConverter478/1
  UnitConverter478/1 -> VOUTP_LRWheelTmpHighDTC_raw32/1  "VOUTP_LRWheelTmpHighDTC_raw32"
  VDDM_RRWheelTmpHighDTC_raw32/1 -> VDDM_RRWheelTmpHighDTC_raw32_Inproc/1  "VDDM_RRWheelTmpHighDTC_raw32"
  VDDM_RRWheelTmpHighDTC_raw32_Inproc/1 -> UnitConverter479/1
  UnitConverter479/1 -> VOUTP_RRWheelTmpHighDTC_raw32/1  "VOUTP_RRWheelTmpHighDTC_raw32"
  VDDM_LFSensorFailDTC_raw32/1 -> VDDM_LFSensorFailDTC_raw32_Inproc/1  "VDDM_LFSensorFailDTC_raw32"
  VDDM_LFSensorFailDTC_raw32_Inproc/1 -> UnitConverter480/1
  UnitConverter480/1 -> VOUTP_LFSensorFailDTC_raw32/1  "VOUTP_LFSensorFailDTC_raw32"
  VDDM_RFSensorFailDTC_raw32/1 -> VDDM_RFSensorFailDTC_raw32_Inproc/1  "VDDM_RFSensorFailDTC_raw32"
  VDDM_RFSensorFailDTC_raw32_Inproc/1 -> UnitConverter481/1
  UnitConverter481/1 -> VOUTP_RFSensorFailDTC_raw32/1  "VOUTP_RFSensorFailDTC_raw32"
  VDDM_LRSensorFailDTC_raw32/1 -> VDDM_LRSensorFailDTC_raw32_Inproc/1  "VDDM_LRSensorFailDTC_raw32"
  VDDM_LRSensorFailDTC_raw32_Inproc/1 -> UnitConverter482/1
  UnitConverter482/1 -> VOUTP_LRSensorFailDTC_raw32/1  "VOUTP_LRSensorFailDTC_raw32"
  VDDM_RRSensorFailDTC_raw32/1 -> VDDM_RRSensorFailDTC_raw32_Inproc/1  "VDDM_RRSensorFailDTC_raw32"
  VDDM_RRSensorFailDTC_raw32_Inproc/1 -> UnitConverter483/1
  UnitConverter483/1 -> VOUTP_RRSensorFailDTC_raw32/1  "VOUTP_RRSensorFailDTC_raw32"
  VDDM_C1EPAS2LCDTC_raw32/1 -> VDDM_C1EPAS2LCDTC_raw32_Inproc/1  "VDDM_C1EPAS2LCDTC_raw32"
  VDDM_C1EPAS2LCDTC_raw32_Inproc/1 -> UnitConverter484/1
  UnitConverter484/1 -> VOUTP_C1EPAS2LCDTC_raw32/1  "VOUTP_C1EPAS2LCDTC_raw32"
  VDDM_5vAPS1PwrErrDTC_raw32/1 -> VDDM_5vAPS1PwrErrDTC_raw32_Inproc/1  "VDDM_5vAPS1PwrErrDTC_raw32"
  VDDM_5vAPS1PwrErrDTC_raw32_Inproc/1 -> UnitConverter485/1
  UnitConverter485/1 -> VOUTP_5vAPS1PwrErrDTC_raw32/1  "VOUTP_5vAPS1PwrErrDTC_raw32"
  VDDM_5vAPS2PwrErrDTC_raw32/1 -> VDDM_5vAPS2PwrErrDTC_raw32_Inproc/1  "VDDM_5vAPS2PwrErrDTC_raw32"
  VDDM_5vAPS2PwrErrDTC_raw32_Inproc/1 -> UnitConverter486/1
  UnitConverter486/1 -> VOUTP_5vAPS2PwrErrDTC_raw32/1  "VOUTP_5vAPS2PwrErrDTC_raw32"
  VDDM_EPBLockTODTC_raw32/1 -> VDDM_EPBLockTODTC_raw32_Inproc/1  "VDDM_EPBLockTODTC_raw32"
  VDDM_EPBLockTODTC_raw32_Inproc/1 -> UnitConverter487/1
  UnitConverter487/1 -> VOUTP_EPBLockTODTC_raw32/1  "VOUTP_EPBLockTODTC_raw32"
  VDDM_EPBUnlockTODTC_raw32/1 -> VDDM_EPBUnlockTODTC_raw32_Inproc/1  "VDDM_EPBUnlockTODTC_raw32"
  VDDM_EPBUnlockTODTC_raw32_Inproc/1 -> UnitConverter488/1
  UnitConverter488/1 -> VOUTP_EPBUnlockTODTC_raw32/1  "VOUTP_EPBUnlockTODTC_raw32"
  VDDM_LimpHomeAct_flg/1 -> VDDM_LimpHomeAct_flg_Inproc/1  "VDDM_LimpHomeAct_flg"
  VDDM_LimpHomeAct_flg_Inproc/1 -> UnitConverter489/1
  UnitConverter489/1 -> VOUTP_LimpHomeAct_flg/1  "VOUTP_LimpHomeAct_flg"
  VDDM_DTCDetect_enum/1 -> VDDM_DTCDetect_enum_Inproc/1  "VDDM_DTCDetect_enum"
  VDDM_DTCDetect_enum_Inproc/1 -> UnitConverter490/1
  UnitConverter490/1 -> VOUTP_DTCDetect_enum/1  "VOUTP_DTCDetect_enum"
  VDDM_EngagePFail_flg/1 -> VDDM_EngagePFail_flg_Inproc/1  "VDDM_EngagePFail_flg"
  VDDM_EngagePFail_flg_Inproc/1 -> UnitConverter491/1
  UnitConverter491/1 -> VOUTP_EngagePFail_flg/1  "VOUTP_EngagePFail_flg"
  VDDM_DisengagePFail_flg/1 -> VDDM_DisengagePFail_flg_Inproc/1  "VDDM_DisengagePFail_flg"
  VDDM_DisengagePFail_flg_Inproc/1 -> UnitConverter492/1
  UnitConverter492/1 -> VOUTP_DisengagePFail_flg/1  "VOUTP_DisengagePFail_flg"
  VDDM_VCURAPSErrLv2_flg/1 -> VDDM_VCURAPSErrLv2_flg_Inproc/1  "VDDM_VCURAPSErrLv2_flg"
  VDDM_VCURAPSErrLv2_flg_Inproc/1 -> UnitConverter493/1
  UnitConverter493/1 -> VOUTP_VCURAPSErrLv2_flg/1  "VOUTP_VCURAPSErrLv2_flg"
  VDDM_VCURAPSErrLv3_flg/1 -> VDDM_VCURAPSErrLv3_flg_Inproc/1  "VDDM_VCURAPSErrLv3_flg"
  VDDM_VCURAPSErrLv3_flg_Inproc/1 -> UnitConverter494/1
  UnitConverter494/1 -> VOUTP_VCURAPSErrLv3_flg/1  "VOUTP_VCURAPSErrLv3_flg"
  VDDM_EDriveSysErrShifterErr_flg/1 -> VDDM_EDriveSysErrShifterErr_flg_Inproc/1  "VDDM_EDriveSysErrShifterErr_flg"
  VDDM_EDriveSysErrShifterErr_flg_Inproc/1 -> UnitConverter495/1
  UnitConverter495/1 -> VOUTP_EDriveSysErrShifterErr_flg/1  "VOUTP_EDriveSysErrShifterErr_flg"
  VDDM_LVSysErrPwrOutErr_flg/1 -> VDDM_LVSysErrPwrOutErr_flg_Inproc/1  "VDDM_LVSysErrPwrOutErr_flg"
  VDDM_LVSysErrPwrOutErr_flg_Inproc/1 -> UnitConverter496/1
  UnitConverter496/1 -> VOUTP_LVSysErrPwrOutErr_flg/1  "VOUTP_LVSysErrPwrOutErr_flg"
  VDDM_HVRlyOpFail_flg/1 -> VDDM_HVRlyOpFail_flg_Inproc/1  "VDDM_HVRlyOpFail_flg"
  VDDM_HVRlyOpFail_flg_Inproc/1 -> UnitConverter497/1
  UnitConverter497/1 -> VOUTP_HVRlyOpFail_flg/1  "VOUTP_HVRlyOpFail_flg"
  VDDM_MCUActDisFail_flg/1 -> VDDM_MCUActDisFail_flg_Inproc/1  "VDDM_MCUActDisFail_flg"
  VDDM_MCUActDisFail_flg_Inproc/1 -> UnitConverter498/1
  UnitConverter498/1 -> VOUTP_MCUActDisFail_flg/1  "VOUTP_MCUActDisFail_flg"
  VDDM_VCUBrkSWSta_enum/1 -> VDDM_VCUBrkSWSta_enum_Inproc/1  "VDDM_VCUBrkSWSta_enum"
  VDDM_VCUBrkSWSta_enum_Inproc/1 -> UnitConverter499/1
  UnitConverter499/1 -> VOUTP_VCUBrkSWSta_enum/1  "VOUTP_VCUBrkSWSta_enum"
  VDDM_VCUFLDoorSta_flg/1 -> VDDM_VCUFLDoorSta_flg_Inproc/1  "VDDM_VCUFLDoorSta_flg"
  VDDM_VCUFLDoorSta_flg_Inproc/1 -> UnitConverter500/1
  UnitConverter500/1 -> VOUTP_VCUFLDoorSta_flg/1  "VOUTP_VCUFLDoorSta_flg"
  VDDM_VCUFRDoorSta_flg/1 -> VDDM_VCUFRDoorSta_flg_Inproc/1  "VDDM_VCUFRDoorSta_flg"
  VDDM_VCUFRDoorSta_flg_Inproc/1 -> UnitConverter501/1
  UnitConverter501/1 -> VOUTP_VCUFRDoorSta_flg/1  "VOUTP_VCUFRDoorSta_flg"
  VDDM_VCURLDoorSta_flg/1 -> VDDM_VCURLDoorSta_flg_Inproc/1  "VDDM_VCURLDoorSta_flg"
  VDDM_VCURLDoorSta_flg_Inproc/1 -> UnitConverter502/1
  UnitConverter502/1 -> VOUTP_VCURLDoorSta_flg/1  "VOUTP_VCURLDoorSta_flg"
  VDDM_VCURRDoorSta_flg/1 -> VDDM_VCURRDoorSta_flg_Inproc/1  "VDDM_VCURRDoorSta_flg"
  VDDM_VCURRDoorSta_flg_Inproc/1 -> UnitConverter503/1
  UnitConverter503/1 -> VOUTP_VCURRDoorSta_flg/1  "VOUTP_VCURRDoorSta_flg"
  VDDM_SysAllowReadySta_flg/1 -> VDDM_SysAllowReadySta_flg_Inproc/1  "VDDM_SysAllowReadySta_flg"
  VDDM_SysAllowReadySta_flg_Inproc/1 -> UnitConverter504/1
  UnitConverter504/1 -> VOUTP_SysAllowReadySta_flg/1  "VOUTP_SysAllowReadySta_flg"
  VDDM_VCUHoodSWSta_flg/1 -> VDDM_VCUHoodSWSta_flg_Inproc/1  "VDDM_VCUHoodSWSta_flg"
  VDDM_VCUHoodSWSta_flg_Inproc/1 -> UnitConverter505/1
  UnitConverter505/1 -> VOUTP_VCUHoodSWSta_flg/1  "VOUTP_VCUHoodSWSta_flg"
  VDDM_VCUTailgateSWSta_flg/1 -> VDDM_VCUTailgateSWSta_flg_Inproc/1  "VDDM_VCUTailgateSWSta_flg"
  VDDM_VCUTailgateSWSta_flg_Inproc/1 -> UnitConverter506/1
  UnitConverter506/1 -> VOUTP_VCUTailgateSWSta_flg/1  "VOUTP_VCUTailgateSWSta_flg"
  VDDM_CAN1BusErrorDTC_raw32/1 -> VDDM_CAN1BusErrorDTC_raw32_Inproc/1  "VDDM_CAN1BusErrorDTC_raw32"
  VDDM_CAN1BusErrorDTC_raw32_Inproc/1 -> UnitConverter507/1
  UnitConverter507/1 -> VOUTP_CAN1BusErrorDTC_raw32/1  "VOUTP_CAN1BusErrorDTC_raw32"
  VDDM_CAN2BusErrorDTC_raw32/1 -> VDDM_CAN2BusErrorDTC_raw32_Inproc/1  "VDDM_CAN2BusErrorDTC_raw32"
  VDDM_CAN2BusErrorDTC_raw32_Inproc/1 -> UnitConverter508/1
  UnitConverter508/1 -> VOUTP_CAN2BusErrorDTC_raw32/1  "VOUTP_CAN2BusErrorDTC_raw32"
  VDDM_CAN3BusErrorDTC_raw32/1 -> VDDM_CAN3BusErrorDTC_raw32_Inproc/1  "VDDM_CAN3BusErrorDTC_raw32"
  VDDM_CAN3BusErrorDTC_raw32_Inproc/1 -> UnitConverter509/1
  UnitConverter509/1 -> VOUTP_CAN3BusErrorDTC_raw32/1  "VOUTP_CAN3BusErrorDTC_raw32"
  VDDM_CAN4BusErrorDTC_raw32/1 -> VDDM_CAN4BusErrorDTC_raw32_Inproc/1  "VDDM_CAN4BusErrorDTC_raw32"
  VDDM_CAN4BusErrorDTC_raw32_Inproc/1 -> UnitConverter510/1
  UnitConverter510/1 -> VOUTP_CAN4BusErrorDTC_raw32/1  "VOUTP_CAN4BusErrorDTC_raw32"
  VDDM_CAN5BusErrorDTC_raw32/1 -> VDDM_CAN5BusErrorDTC_raw32_Inproc/1  "VDDM_CAN5BusErrorDTC_raw32"
  VDDM_CAN5BusErrorDTC_raw32_Inproc/1 -> UnitConverter511/1
  UnitConverter511/1 -> VOUTP_CAN5BusErrorDTC_raw32/1  "VOUTP_CAN5BusErrorDTC_raw32"
  VDDM_CAN6BusErrorDTC_raw32/1 -> VDDM_CAN6BusErrorDTC_raw32_Inproc/1  "VDDM_CAN6BusErrorDTC_raw32"
  VDDM_CAN6BusErrorDTC_raw32_Inproc/1 -> UnitConverter512/1
  UnitConverter512/1 -> VOUTP_CAN6BusErrorDTC_raw32/1  "VOUTP_CAN6BusErrorDTC_raw32"
  VDDM_FrMCU4PreDTC_raw32/1 -> VDDM_FrMCU4PreDTC_raw32_Inproc/1  "VDDM_FrMCU4PreDTC_raw32"
  VDDM_FrMCU4PreDTC_raw32_Inproc/1 -> UnitConverter513/1
  UnitConverter513/1 -> VOUTP_FrMCU4PreDTC_raw32/1  "VOUTP_FrMCU4PreDTC_raw32"
  VDDM_FrMCUDisDTC_raw32/1 -> VDDM_FrMCUDisDTC_raw32_Inproc/1  "VDDM_FrMCUDisDTC_raw32"
  VDDM_FrMCUDisDTC_raw32_Inproc/1 -> UnitConverter514/1
  UnitConverter514/1 -> VOUTP_FrMCUDisDTC_raw32/1  "VOUTP_FrMCUDisDTC_raw32"
  VDDM_FrMCUActDTC_raw32/1 -> VDDM_FrMCUActDTC_raw32_Inproc/1  "VDDM_FrMCUActDTC_raw32"
  VDDM_FrMCUActDTC_raw32_Inproc/1 -> UnitConverter515/1
  UnitConverter515/1 -> VOUTP_FrMCUActDTC_raw32/1  "VOUTP_FrMCUActDTC_raw32"
  VDDM_RegenErrDTC_raw32/1 -> VDDM_RegenErrDTC_raw32_Inproc/1  "VDDM_RegenErrDTC_raw32"
  VDDM_RegenErrDTC_raw32_Inproc/1 -> UnitConverter516/1
  UnitConverter516/1 -> VOUTP_RegenErrDTC_raw32/1  "VOUTP_RegenErrDTC_raw32"
  VDHP_ActAPSPosn_pct/1 -> VDHP_ActAPSPosn_pct_Inproc/1  "VDHP_ActAPSPosn_pct"
  VDHP_ActAPSPosn_pct_Inproc/1 -> UnitConverter517/1
  UnitConverter517/1 -> VOUTP_ActAPSPosn_pct/1  "VOUTP_ActAPSPosn_pct"
  VDHP_LowIdleAccPedal_flg/1 -> VDHP_LowIdleAccPedal_flg_Inproc/1  "VDHP_LowIdleAccPedal_flg"
  VDHP_LowIdleAccPedal_flg_Inproc/1 -> UnitConverter518/1
  UnitConverter518/1 -> VOUTP_LowIdleAccPedal_flg/1  "VOUTP_LowIdleAccPedal_flg"
  VDHP_EAPS1MIN_pct/1 -> VDHP_EAPS1MIN_pct_Inproc/1  "VDHP_EAPS1MIN_pct"
  VDHP_EAPS1MIN_pct_Inproc/1 -> UnitConverter519/1
  UnitConverter519/1 -> VOUTP_EAPS1MIN_pct/1  "VOUTP_EAPS1MIN_pct"
  VDHP_EAPS2MIN_pct/1 -> VDHP_EAPS2MIN_pct_Inproc/1  "VDHP_EAPS2MIN_pct"
  VDHP_EAPS2MIN_pct_Inproc/1 -> UnitConverter520/1
  UnitConverter520/1 -> VOUTP_EAPS2MIN_pct/1  "VOUTP_EAPS2MIN_pct"
  VDHP_ResetPedalZeroPosStart_flg/1 -> VDHP_ResetPedalZeroPosStart_flg_Inproc/1  "VDHP_ResetPedalZeroPosStart_flg"
  VDHP_ResetPedalZeroPosStart_flg_Inproc/1 -> UnitConverter521/1
  UnitConverter521/1 -> VOUTP_ResetPedalZeroPosStart_flg/1  "VOUTP_ResetPedalZeroPosStart_flg"
  VDHP_EAPS1NRM_pct/1 -> VDHP_EAPS1NRM_pct_Inproc/1  "VDHP_EAPS1NRM_pct"
  VDHP_EAPS1NRM_pct_Inproc/1 -> UnitConverter522/1
  UnitConverter522/1 -> VOUTP_EAPS1NRM_pct/1  "VOUTP_EAPS1NRM_pct"
  VDHP_EAPS2NRM_pct/1 -> VDHP_EAPS2NRM_pct_Inproc/1  "VDHP_EAPS2NRM_pct"
  VDHP_EAPS2NRM_pct_Inproc/1 -> UnitConverter523/1
  UnitConverter523/1 -> VOUTP_EAPS2NRM_pct/1  "VOUTP_EAPS2NRM_pct"
  VDHP_EAPS1RAW_pct/1 -> VDHP_EAPS1RAW_pct_Inproc/1  "VDHP_EAPS1RAW_pct"
  VDHP_EAPS1RAW_pct_Inproc/1 -> UnitConverter524/1
  UnitConverter524/1 -> VOUTP_EAPS1RAW_pct/1  "VOUTP_EAPS1RAW_pct"
  VDHP_EAPS2RAW_pct/1 -> VDHP_EAPS2RAW_pct_Inproc/1  "VDHP_EAPS2RAW_pct"
  VDHP_EAPS2RAW_pct_Inproc/1 -> UnitConverter525/1
  UnitConverter525/1 -> VOUTP_EAPS2RAW_pct/1  "VOUTP_EAPS2RAW_pct"
  VDID_VSS_kph/1 -> VDID_VSS_kph_Inproc/1  "VDID_VSS_kph"
  VDID_VSS_kph_Inproc/1 -> UnitConverter526/1
  UnitConverter526/1 -> VOUTP_VSS_kph/1  "VOUTP_VSS_kph"
  VDID_RUNTM_s/1 -> VDID_RUNTM_s_Inproc/1  "VDID_RUNTM_s"
  VDID_RUNTM_s_Inproc/1 -> UnitConverter527/1
  UnitConverter527/1 -> VOUTP_RUNTM_s/1  "VOUTP_RUNTM_s"
  VDID_MILDIST_km/1 -> VDID_MILDIST_km_Inproc/1  "VDID_MILDIST_km"
  VDID_MILDIST_km_Inproc/1 -> UnitConverter528/1
  UnitConverter528/1 -> VOUTP_MILDIST_km/1  "VOUTP_MILDIST_km"
  VDID_CLRDIST_km/1 -> VDID_CLRDIST_km_Inproc/1  "VDID_CLRDIST_km"
  VDID_CLRDIST_km_Inproc/1 -> UnitConverter529/1
  UnitConverter529/1 -> VOUTP_CLRDIST_km/1  "VOUTP_CLRDIST_km"
  VDID_APPD_pct/1 -> VDID_APPD_pct_Inproc/1  "VDID_APPD_pct"
  VDID_APPD_pct_Inproc/1 -> UnitConverter530/1
  UnitConverter530/1 -> VOUTP_APPD_pct/1  "VOUTP_APPD_pct"
  VDID_APPE_pct/1 -> VDID_APPE_pct_Inproc/1  "VDID_APPE_pct"
  VDID_APPE_pct_Inproc/1 -> UnitConverter531/1
  UnitConverter531/1 -> VOUTP_APPE_pct/1  "VOUTP_APPE_pct"
  VDID_ODOMETER_km/1 -> VDID_ODOMETER_km_Inproc/1  "VDID_ODOMETER_km"
  VDID_ODOMETER_km_Inproc/1 -> UnitConverter532/1
  UnitConverter532/1 -> VOUTP_ODOMETER_km/1  "VOUTP_ODOMETER_km"
  VDID_NUMPSATRIPSFLTMEMCLR_cnt/1 -> VDID_NUMPSATRIPSFLTMEMCLR_cnt_Inproc/1  "VDID_NUMPSATRIPSFLTMEMCLR_cnt"
  VDID_NUMPSATRIPSFLTMEMCLR_cnt_Inproc/1 -> UnitConverter533/1
  UnitConverter533/1 -> VOUTP_NUMPSATRIPSFLTMEMCLR_cnt/1  "VOUTP_NUMPSATRIPSFLTMEMCLR_cnt"
  VDID_PSAR_sec/1 -> VDID_PSAR_sec_Inproc/1  "VDID_PSAR_sec"
  VDID_PSAR_sec_Inproc/1 -> UnitConverter534/1
  UnitConverter534/1 -> VOUTP_PSAR_sec/1  "VOUTP_PSAR_sec"
  VDID_PSAL_sec/1 -> VDID_PSAL_sec_Inproc/1  "VDID_PSAL_sec"
  VDID_PSAL_sec_Inproc/1 -> UnitConverter535/1
  UnitConverter535/1 -> VOUTP_PSAL_sec/1  "VOUTP_PSAL_sec"
  VDID_IPSAR_sec/1 -> VDID_IPSAR_sec_Inproc/1  "VDID_IPSAR_sec"
  VDID_IPSAR_sec_Inproc/1 -> UnitConverter536/1
  UnitConverter536/1 -> VOUTP_IPSAR_sec/1  "VOUTP_IPSAR_sec"
  VDID_IPSAL_sec/1 -> VDID_IPSAL_sec_Inproc/1  "VDID_IPSAL_sec"
  VDID_IPSAL_sec_Inproc/1 -> UnitConverter537/1
  UnitConverter537/1 -> VOUTP_IPSAL_sec/1  "VOUTP_IPSAL_sec"
  VDID_CPSAR_sec/1 -> VDID_CPSAR_sec_Inproc/1  "VDID_CPSAR_sec"
  VDID_CPSAR_sec_Inproc/1 -> UnitConverter538/1
  UnitConverter538/1 -> VOUTP_CPSAR_sec/1  "VOUTP_CPSAR_sec"
  VDID_CPSAL_sec/1 -> VDID_CPSAL_sec_Inproc/1  "VDID_CPSAL_sec"
  VDID_CPSAL_sec_Inproc/1 -> UnitConverter539/1
  UnitConverter539/1 -> VOUTP_CPSAL_sec/1  "VOUTP_CPSAL_sec"
  VDID_PKER_kphsqr/1 -> VDID_PKER_kphsqr_Inproc/1  "VDID_PKER_kphsqr"
  VDID_PKER_kphsqr_Inproc/1 -> UnitConverter540/1
  UnitConverter540/1 -> VOUTP_PKER_kphsqr/1  "VOUTP_PKER_kphsqr"
  VDID_PKEL_kphsqr/1 -> VDID_PKEL_kphsqr_Inproc/1  "VDID_PKEL_kphsqr"
  VDID_PKEL_kphsqr_Inproc/1 -> UnitConverter541/1
  UnitConverter541/1 -> VOUTP_PKEL_kphsqr/1  "VOUTP_PKEL_kphsqr"
  VDID_ResetCDEODTR_km/1 -> VDID_ResetCDEODTR_km_Inproc/1  "VDID_ResetCDEODTR_km"
  VDID_ResetCDEODTR_km_Inproc/1 -> UnitConverter542/1
  UnitConverter542/1 -> VOUTP_ResetCDEODTR_km/1  "VOUTP_ResetCDEODTR_km"
  VDID_CDEODTR_km/1 -> VDID_CDEODTR_km_Inproc/1  "VDID_CDEODTR_km"
  VDID_CDEODTR_km_Inproc/1 -> UnitConverter543/1
  UnitConverter543/1 -> VOUTP_CDEODTR_km/1  "VOUTP_CDEODTR_km"
  VDID_CDEODTL_km/1 -> VDID_CDEODTL_km_Inproc/1  "VDID_CDEODTL_km"
  VDID_CDEODTL_km_Inproc/1 -> UnitConverter544/1
  UnitConverter544/1 -> VOUTP_CDEODTL_km/1  "VOUTP_CDEODTL_km"
  VDID_QTYPSATRIPSR_cnt/1 -> VDID_QTYPSATRIPSR_cnt_Inproc/1  "VDID_QTYPSATRIPSR_cnt"
  VDID_QTYPSATRIPSR_cnt_Inproc/1 -> UnitConverter545/1
  UnitConverter545/1 -> VOUTP_QTYPSATRIPSR_cnt/1  "VOUTP_QTYPSATRIPSR_cnt"
  VDID_QTYPSATRIPSL_cnt/1 -> VDID_QTYPSATRIPSL_cnt_Inproc/1  "VDID_QTYPSATRIPSL_cnt"
  VDID_QTYPSATRIPSL_cnt_Inproc/1 -> UnitConverter546/1
  UnitConverter546/1 -> VOUTP_QTYPSATRIPSL_cnt/1  "VOUTP_QTYPSATRIPSL_cnt"
  VDID_PROTOCOLID_enum/1 -> VDID_PROTOCOLID_enum_Inproc/1  "VDID_PROTOCOLID_enum"
  VDID_PROTOCOLID_enum_Inproc/1 -> UnitConverter547/1
  UnitConverter547/1 -> VOUTP_PROTOCOLID_enum/1  "VOUTP_PROTOCOLID_enum"
  VDID_CALID_cnt/1 -> VDID_CALID_cnt_Inproc/1  "VDID_CALID_cnt"
  VDID_CALID_cnt_Inproc/1 -> UnitConverter548/1
  UnitConverter548/1 -> VOUTP_CALID_cnt/1  "VOUTP_CALID_cnt"
  VDID_ECUNAME_cnt/1 -> VDID_ECUNAME_cnt_Inproc/1  "VDID_ECUNAME_cnt"
  VDID_ECUNAME_cnt_Inproc/1 -> UnitConverter549/1
  UnitConverter549/1 -> VOUTP_ECUNAME_cnt/1  "VOUTP_ECUNAME_cnt"
  VDID_PKERNumerator_kphsqr/1 -> VDID_PKERNumerator_kphsqr_Inproc/1  "VDID_PKERNumerator_kphsqr"
  VDID_PKERNumerator_kphsqr_Inproc/1 -> UnitConverter550/1
  UnitConverter550/1 -> VOUTP_PKERNumerator_kphsqr/1  "VOUTP_PKERNumerator_kphsqr"
  VDID_PKELNumerator_kphsqr/1 -> VDID_PKELNumerator_kphsqr_Inproc/1  "VDID_PKELNumerator_kphsqr"
  VDID_PKELNumerator_kphsqr_Inproc/1 -> UnitConverter551/1
  UnitConverter551/1 -> VOUTP_PKELNumerator_kphsqr/1  "VOUTP_PKELNumerator_kphsqr"
  VDID_VinCode_cnt/1 -> VDID_VinCode_cnt_Inproc/1  "VDID_VinCode_cnt"
  VDID_VinCode_cnt_Inproc/1 -> UnitConverter552/1
  UnitConverter552/1 -> VOUTP_VinCode_cnt/1  "VOUTP_VinCode_cnt"
  VDID_DIDModelVersion_raw/1 -> VDID_DIDModelVersion_raw_Inproc/1  "VDID_DIDModelVersion_raw"
  VDID_DIDModelVersion_raw_Inproc/1 -> UnitConverter553/1
  UnitConverter553/1 -> VOUTP_DIDModelVersion_raw/1  "VOUTP_DIDModelVersion_raw"
  VDID_DIDModelVersionChksum_raw/1 -> VDID_DIDModelVersionChksum_raw_Inproc/1  "VDID_DIDModelVersionChksum_raw"
  VDID_DIDModelVersionChksum_raw_Inproc/1 -> UnitConverter554/1
  UnitConverter554/1 -> VOUTP_DIDModelVersionChksum_raw/1  "VOUTP_DIDModelVersionChksum_raw"
  VDKC_DKCTimeSN_cnt/1 -> VDKC_DKCTimeSN_cnt_Inproc/1  "VDKC_DKCTimeSN_cnt"
  VDKC_DKCTimeSN_cnt_Inproc/1 -> UnitConverter555/1
  UnitConverter555/1 -> VOUTP_DKCTimeSN_cnt/1  "VOUTP_DKCTimeSN_cnt"
  VDKC_DKCAuthSta_enum/1 -> VDKC_DKCAuthSta_enum_Inproc/1  "VDKC_DKCAuthSta_enum"
  VDKC_DKCAuthSta_enum_Inproc/1 -> UnitConverter556/1
  UnitConverter556/1 -> VOUTP_DKCAuthSta_enum/1  "VOUTP_DKCAuthSta_enum"
  VDKC_TimeSNDKCFbk_cnt/1 -> VDKC_TimeSNDKCFbk_cnt_Inproc/1  "VDKC_TimeSNDKCFbk_cnt"
  VDKC_TimeSNDKCFbk_cnt_Inproc/1 -> UnitConverter557/1
  UnitConverter557/1 -> VOUTP_TimeSNDKCFbk_cnt/1  "VOUTP_TimeSNDKCFbk_cnt"
  VDKC_PCommandToBCM_enum/1 -> VDKC_PCommandToBCM_enum_Inproc/1  "VDKC_PCommandToBCM_enum"
  VDKC_PCommandToBCM_enum_Inproc/1 -> UnitConverter558/1
  UnitConverter558/1 -> VOUTP_PCommandToBCM_enum/1  "VOUTP_PCommandToBCM_enum"
  VDKC_KeyAreaLockUnlock_enum/1 -> VDKC_KeyAreaLockUnlock_enum_Inproc/1  "VDKC_KeyAreaLockUnlock_enum"
  VDKC_KeyAreaLockUnlock_enum_Inproc/1 -> UnitConverter559/1
  UnitConverter559/1 -> VOUTP_KeyAreaLockUnlock_enum/1  "VOUTP_KeyAreaLockUnlock_enum"
  VDKC_KeyMissSta_flg/1 -> VDKC_KeyMissSta_flg_Inproc/1  "VDKC_KeyMissSta_flg"
  VDKC_KeyMissSta_flg_Inproc/1 -> UnitConverter560/1
  UnitConverter560/1 -> VOUTP_KeyMissSta_flg/1  "VOUTP_KeyMissSta_flg"
  VDKC_ShippingMode_flg/1 -> VDKC_ShippingMode_flg_Inproc/1  "VDKC_ShippingMode_flg"
  VDKC_ShippingMode_flg_Inproc/1 -> UnitConverter561/1
  UnitConverter561/1 -> VOUTP_ShippingMode_flg/1  "VOUTP_ShippingMode_flg"
  VDKC_KeyNumSta_enum/1 -> VDKC_KeyNumSta_enum_Inproc/1  "VDKC_KeyNumSta_enum"
  VDKC_KeyNumSta_enum_Inproc/1 -> UnitConverter562/1
  UnitConverter562/1 -> VOUTP_KeyNumSta_enum/1  "VOUTP_KeyNumSta_enum"
  VDKC_DkeyShowIVISta_enum/1 -> VDKC_DkeyShowIVISta_enum_Inproc/1  "VDKC_DkeyShowIVISta_enum"
  VDKC_DkeyShowIVISta_enum_Inproc/1 -> UnitConverter563/1
  UnitConverter563/1 -> VOUTP_DkeyShowIVISta_enum/1  "VOUTP_DkeyShowIVISta_enum"
  VDKC_DkeyAreaRAPSSta_enum/1 -> VDKC_DkeyAreaRAPSSta_enum_Inproc/1  "VDKC_DkeyAreaRAPSSta_enum"
  VDKC_DkeyAreaRAPSSta_enum_Inproc/1 -> UnitConverter564/1
  UnitConverter564/1 -> VOUTP_DkeyAreaRAPSSta_enum/1  "VOUTP_DkeyAreaRAPSSta_enum"
  VDKC_KeyAreaPS_enum/1 -> VDKC_KeyAreaPS_enum_Inproc/1  "VDKC_KeyAreaPS_enum"
  VDKC_KeyAreaPS_enum_Inproc/1 -> UnitConverter565/1
  UnitConverter565/1 -> VOUTP_KeyAreaPS_enum/1  "VOUTP_KeyAreaPS_enum"
  VDKC_KeyAreaSPTGSta_enum/1 -> VDKC_KeyAreaSPTGSta_enum_Inproc/1  "VDKC_KeyAreaSPTGSta_enum"
  VDKC_KeyAreaSPTGSta_enum_Inproc/1 -> UnitConverter566/1
  UnitConverter566/1 -> VOUTP_KeyAreaSPTGSta_enum/1  "VOUTP_KeyAreaSPTGSta_enum"
  VDKC_KeyAreaPTG_enum/1 -> VDKC_KeyAreaPTG_enum_Inproc/1  "VDKC_KeyAreaPTG_enum"
  VDKC_KeyAreaPTG_enum_Inproc/1 -> UnitConverter567/1
  UnitConverter567/1 -> VOUTP_KeyAreaPTG_enum/1  "VOUTP_KeyAreaPTG_enum"
  VDKC_UWB4Invalid_flg/1 -> VDKC_UWB4Invalid_flg_Inproc/1  "VDKC_UWB4Invalid_flg"
  VDKC_UWB4Invalid_flg_Inproc/1 -> UnitConverter568/1
  UnitConverter568/1 -> VOUTP_UWB4Invalid_flg/1  "VOUTP_UWB4Invalid_flg"
  VDKC_UWBOnOff_flg/1 -> VDKC_UWBOnOff_flg_Inproc/1  "VDKC_UWBOnOff_flg"
  VDKC_UWBOnOff_flg_Inproc/1 -> UnitConverter569/1
  UnitConverter569/1 -> VOUTP_UWBOnOff_flg/1  "VOUTP_UWBOnOff_flg"
  VDKC_UWB3Invalid_flg/1 -> VDKC_UWB3Invalid_flg_Inproc/1  "VDKC_UWB3Invalid_flg"
  VDKC_UWB3Invalid_flg_Inproc/1 -> UnitConverter570/1
  UnitConverter570/1 -> VOUTP_UWB3Invalid_flg/1  "VOUTP_UWB3Invalid_flg"
  VDKC_UWB1Invalid_flg/1 -> VDKC_UWB1Invalid_flg_Inproc/1  "VDKC_UWB1Invalid_flg"
  VDKC_UWB1Invalid_flg_Inproc/1 -> UnitConverter571/1
  UnitConverter571/1 -> VOUTP_UWB1Invalid_flg/1  "VOUTP_UWB1Invalid_flg"
  VDKC_UWB2Invalid_flg/1 -> VDKC_UWB2Invalid_flg_Inproc/1  "VDKC_UWB2Invalid_flg"
  VDKC_UWB2Invalid_flg_Inproc/1 -> UnitConverter572/1
  UnitConverter572/1 -> VOUTP_UWB2Invalid_flg/1  "VOUTP_UWB2Invalid_flg"
  VDKC_UWB0Invalid_flg/1 -> VDKC_UWB0Invalid_flg_Inproc/1  "VDKC_UWB0Invalid_flg"
  VDKC_UWB0Invalid_flg_Inproc/1 -> UnitConverter573/1
  UnitConverter573/1 -> VOUTP_UWB0Invalid_flg/1  "VOUTP_UWB0Invalid_flg"
  VDKC_UIDBatVolt_enum/1 -> VDKC_UIDBatVolt_enum_Inproc/1  "VDKC_UIDBatVolt_enum"
  VDKC_UIDBatVolt_enum_Inproc/1 -> UnitConverter574/1
  UnitConverter574/1 -> VOUTP_UIDBatVolt_enum/1  "VOUTP_UIDBatVolt_enum"
  VDKC_CoordinateX_enum/1 -> VDKC_CoordinateX_enum_Inproc/1  "VDKC_CoordinateX_enum"
  VDKC_CoordinateX_enum_Inproc/1 -> UnitConverter575/1
  UnitConverter575/1 -> VOUTP_CoordinateX_enum/1  "VOUTP_CoordinateX_enum"
  VDKC_FDCSPTGDet_flg/1 -> VDKC_FDCSPTGDet_flg_Inproc/1  "VDKC_FDCSPTGDet_flg"
  VDKC_FDCSPTGDet_flg_Inproc/1 -> UnitConverter576/1
  UnitConverter576/1 -> VOUTP_FDCSPTGDet_flg/1  "VOUTP_FDCSPTGDet_flg"
  VDKC_FDCSPTGOpen_flg/1 -> VDKC_FDCSPTGOpen_flg_Inproc/1  "VDKC_FDCSPTGOpen_flg"
  VDKC_FDCSPTGOpen_flg_Inproc/1 -> UnitConverter577/1
  UnitConverter577/1 -> VOUTP_FDCSPTGOpen_flg/1  "VOUTP_FDCSPTGOpen_flg"
  VDKC_UIDLowPowerSta_flg/1 -> VDKC_UIDLowPowerSta_flg_Inproc/1  "VDKC_UIDLowPowerSta_flg"
  VDKC_UIDLowPowerSta_flg_Inproc/1 -> UnitConverter578/1
  UnitConverter578/1 -> VOUTP_UIDLowPowerSta_flg/1  "VOUTP_UIDLowPowerSta_flg"
  VDKC_CoordinateY_enum/1 -> VDKC_CoordinateY_enum_Inproc/1  "VDKC_CoordinateY_enum"
  VDKC_CoordinateY_enum_Inproc/1 -> UnitConverter579/1
  UnitConverter579/1 -> VOUTP_CoordinateY_enum/1  "VOUTP_CoordinateY_enum"
  VDKC_AllowSleep_flg/1 -> VDKC_AllowSleep_flg_Inproc/1  "VDKC_AllowSleep_flg"
  VDKC_AllowSleep_flg_Inproc/1 -> UnitConverter580/1
  UnitConverter580/1 -> VOUTP_AllowSleep_flg/1  "VOUTP_AllowSleep_flg"
  VDKC_KeyTypeSta_enum/1 -> VDKC_KeyTypeSta_enum_Inproc/1  "VDKC_KeyTypeSta_enum"
  VDKC_KeyTypeSta_enum_Inproc/1 -> UnitConverter581/1
  UnitConverter581/1 -> VOUTP_KeyTypeSta_enum/1  "VOUTP_KeyTypeSta_enum"
  VDKC_CalDistance_enum/1 -> VDKC_CalDistance_enum_Inproc/1  "VDKC_CalDistance_enum"
  VDKC_CalDistance_enum_Inproc/1 -> UnitConverter582/1
  UnitConverter582/1 -> VOUTP_CalDistance_enum/1  "VOUTP_CalDistance_enum"
  VDKC_UWBDetPTGArea_enum/1 -> VDKC_UWBDetPTGArea_enum_Inproc/1  "VDKC_UWBDetPTGArea_enum"
  VDKC_UWBDetPTGArea_enum_Inproc/1 -> UnitConverter583/1
  UnitConverter583/1 -> VOUTP_UWBDetPTGArea_enum/1  "VOUTP_UWBDetPTGArea_enum"
  VDKC_A0UWBEvent_enum/1 -> VDKC_A0UWBEvent_enum_Inproc/1  "VDKC_A0UWBEvent_enum"
  VDKC_A0UWBEvent_enum_Inproc/1 -> UnitConverter584/1
  UnitConverter584/1 -> VOUTP_A0UWBEvent_enum/1  "VOUTP_A0UWBEvent_enum"
  VDKC_ParkingModeCmd_enum/1 -> VDKC_ParkingModeCmd_enum_Inproc/1  "VDKC_ParkingModeCmd_enum"
  VDKC_ParkingModeCmd_enum_Inproc/1 -> UnitConverter585/1
  UnitConverter585/1 -> VOUTP_ParkingModeCmd_enum/1  "VOUTP_ParkingModeCmd_enum"
  VDKC_KeyModeSta_enum/1 -> VDKC_KeyModeSta_enum_Inproc/1  "VDKC_KeyModeSta_enum"
  VDKC_KeyModeSta_enum_Inproc/1 -> UnitConverter586/1
  UnitConverter586/1 -> VOUTP_KeyModeSta_enum/1  "VOUTP_KeyModeSta_enum"
  VDKC_ReVehData_enum/1 -> VDKC_ReVehData_enum_Inproc/1  "VDKC_ReVehData_enum"
  VDKC_ReVehData_enum_Inproc/1 -> UnitConverter587/1
  UnitConverter587/1 -> VOUTP_ReVehData_enum/1  "VOUTP_ReVehData_enum"
  VDKC_UWB0Distance_enum/1 -> VDKC_UWB0Distance_enum_Inproc/1  "VDKC_UWB0Distance_enum"
  VDKC_UWB0Distance_enum_Inproc/1 -> UnitConverter588/1
  UnitConverter588/1 -> VOUTP_UWB0Distance_enum/1  "VOUTP_UWB0Distance_enum"
  VDKC_DKeyWelcomeSta_enum/1 -> VDKC_DKeyWelcomeSta_enum_Inproc/1  "VDKC_DKeyWelcomeSta_enum"
  VDKC_DKeyWelcomeSta_enum_Inproc/1 -> UnitConverter589/1
  UnitConverter589/1 -> VOUTP_DKeyWelcomeSta_enum/1  "VOUTP_DKeyWelcomeSta_enum"
  VDKC_UWB1Distance_enum/1 -> VDKC_UWB1Distance_enum_Inproc/1  "VDKC_UWB1Distance_enum"
  VDKC_UWB1Distance_enum_Inproc/1 -> UnitConverter590/1
  UnitConverter590/1 -> VOUTP_UWB1Distance_enum/1  "VOUTP_UWB1Distance_enum"
  VDKC_UWB2Distance_enum/1 -> VDKC_UWB2Distance_enum_Inproc/1  "VDKC_UWB2Distance_enum"
  VDKC_UWB2Distance_enum_Inproc/1 -> UnitConverter591/1
  UnitConverter591/1 -> VOUTP_UWB2Distance_enum/1  "VOUTP_UWB2Distance_enum"
  VDKC_UWB3Distance_enum/1 -> VDKC_UWB3Distance_enum_Inproc/1  "VDKC_UWB3Distance_enum"
  VDKC_UWB3Distance_enum_Inproc/1 -> UnitConverter592/1
  UnitConverter592/1 -> VOUTP_UWB3Distance_enum/1  "VOUTP_UWB3Distance_enum"
  VDKC_UWB4Distance_enum/1 -> VDKC_UWB4Distance_enum_Inproc/1  "VDKC_UWB4Distance_enum"
  VDKC_UWB4Distance_enum_Inproc/1 -> UnitConverter593/1
  UnitConverter593/1 -> VOUTP_UWB4Distance_enum/1  "VOUTP_UWB4Distance_enum"
  VDKC_BLERSSI_enum/1 -> VDKC_BLERSSI_enum_Inproc/1  "VDKC_BLERSSI_enum"
  VDKC_BLERSSI_enum_Inproc/1 -> UnitConverter594/1
  UnitConverter594/1 -> VOUTP_BLERSSI_enum/1  "VOUTP_BLERSSI_enum"
  VDKC_BLEdcEvent_enum/1 -> VDKC_BLEdcEvent_enum_Inproc/1  "VDKC_BLEdcEvent_enum"
  VDKC_BLEdcEvent_enum_Inproc/1 -> UnitConverter595/1
  UnitConverter595/1 -> VOUTP_BLEdcEvent_enum/1  "VOUTP_BLEdcEvent_enum"
  VDKC_UWB0FPP_enum/1 -> VDKC_UWB0FPP_enum_Inproc/1  "VDKC_UWB0FPP_enum"
  VDKC_UWB0FPP_enum_Inproc/1 -> UnitConverter596/1
  UnitConverter596/1 -> VOUTP_UWB0FPP_enum/1  "VOUTP_UWB0FPP_enum"
  VDKC_UWB1FPP_enum/1 -> VDKC_UWB1FPP_enum_Inproc/1  "VDKC_UWB1FPP_enum"
  VDKC_UWB1FPP_enum_Inproc/1 -> UnitConverter597/1
  UnitConverter597/1 -> VOUTP_UWB1FPP_enum/1  "VOUTP_UWB1FPP_enum"
  VDKC_UWB2FPP_enum/1 -> VDKC_UWB2FPP_enum_Inproc/1  "VDKC_UWB2FPP_enum"
  VDKC_UWB2FPP_enum_Inproc/1 -> UnitConverter598/1
  UnitConverter598/1 -> VOUTP_UWB2FPP_enum/1  "VOUTP_UWB2FPP_enum"
  VDKC_UWB3FPP_enum/1 -> VDKC_UWB3FPP_enum_Inproc/1  "VDKC_UWB3FPP_enum"
  VDKC_UWB3FPP_enum_Inproc/1 -> UnitConverter599/1
  UnitConverter599/1 -> VOUTP_UWB3FPP_enum/1  "VOUTP_UWB3FPP_enum"
  VDKC_UWB4FPP_enum/1 -> VDKC_UWB4FPP_enum_Inproc/1  "VDKC_UWB4FPP_enum"
  VDKC_UWB4FPP_enum_Inproc/1 -> UnitConverter600/1
  UnitConverter600/1 -> VOUTP_UWB4FPP_enum/1  "VOUTP_UWB4FPP_enum"
  VDKC_UWBDetArea_enum/1 -> VDKC_UWBDetArea_enum_Inproc/1  "VDKC_UWBDetArea_enum"
  VDKC_UWBDetArea_enum_Inproc/1 -> UnitConverter601/1
  UnitConverter601/1 -> VOUTP_UWBDetArea_enum/1  "VOUTP_UWBDetArea_enum"
  VDKC_OutputPCMDModule_enum/1 -> VDKC_OutputPCMDModule_enum_Inproc/1  "VDKC_OutputPCMDModule_enum"
  VDKC_OutputPCMDModule_enum_Inproc/1 -> UnitConverter602/1
  UnitConverter602/1 -> VOUTP_OutputPCMDModule_enum/1  "VOUTP_OutputPCMDModule_enum"
  VDKC_FDCDKCAllowSleep_flg/1 -> VDKC_FDCDKCAllowSleep_flg_Inproc/1  "VDKC_FDCDKCAllowSleep_flg"
  VDKC_FDCDKCAllowSleep_flg_Inproc/1 -> UnitConverter603/1
  UnitConverter603/1 -> VOUTP_FDCDKCAllowSleep_flg/1  "VOUTP_FDCDKCAllowSleep_flg"
  VDKC_JudgeKeepUnlockZone_flg/1 -> VDKC_JudgeKeepUnlockZone_flg_Inproc/1  "VDKC_JudgeKeepUnlockZone_flg"
  VDKC_JudgeKeepUnlockZone_flg_Inproc/1 -> UnitConverter604/1
  UnitConverter604/1 -> VOUTP_JudgeKeepUnlockZone_flg/1  "VOUTP_JudgeKeepUnlockZone_flg"
  VDSC_DISCTurn_flg/1 -> VDSC_DISCTurn_flg_Inproc/1  "VDSC_DISCTurn_flg"
  VDSC_DISCTurn_flg_Inproc/1 -> UnitConverter605/1
  UnitConverter605/1 -> VOUTP_DISCTurn_flg/1  "VOUTP_DISCTurn_flg"
  VDSC_DISCTargetSpd_kph/1 -> VDSC_DISCTargetSpd_kph_Inproc/1  "VDSC_DISCTargetSpd_kph"
  VDSC_DISCTargetSpd_kph_Inproc/1 -> UnitConverter606/1
  UnitConverter606/1 -> VOUTP_DISCTargetSpd_kph/1  "VOUTP_DISCTargetSpd_kph"
  VDSC_DISCSta_enum/1 -> VDSC_DISCSta_enum_Inproc/1  "VDSC_DISCSta_enum"
  VDSC_DISCSta_enum_Inproc/1 -> UnitConverter607/1
  UnitConverter607/1 -> VOUTP_DISCSta_enum/1  "VOUTP_DISCSta_enum"
  VDSC_DISCButtSta_flg/1 -> VDSC_DISCButtSta_flg_Inproc/1  "VDSC_DISCButtSta_flg"
  VDSC_DISCButtSta_flg_Inproc/1 -> UnitConverter608/1
  UnitConverter608/1 -> VOUTP_DISCButtSta_flg/1  "VOUTP_DISCButtSta_flg"
  VNMM_AllCANTxReq_flg/1 -> VNMM_AllCANTxReq_flg_Inproc/1  "VNMM_AllCANTxReq_flg"
  VNMM_AllCANTxReq_flg_Inproc/1 -> UnitConverter609/1
  UnitConverter609/1 -> VOUTP_AllCANTxReq_flg/1  "VOUTP_AllCANTxReq_flg"
  VNMM_NMmTxReq_flg/1 -> VNMM_NMmTxReq_flg_Inproc/1  "VNMM_NMmTxReq_flg"
  VNMM_NMmTxReq_flg_Inproc/1 -> UnitConverter610/1
  UnitConverter610/1 -> VOUTP_NMmTxReq_flg/1  "VOUTP_NMmTxReq_flg"
  VNMM_Awake_enum/1 -> VNMM_Awake_enum_Inproc/1  "VNMM_Awake_enum"
  VNMM_Awake_enum_Inproc/1 -> UnitConverter611/1
  UnitConverter611/1 -> VOUTP_Awake_enum/1  "VOUTP_Awake_enum"
  VNMM_CSB_flg/1 -> VNMM_CSB_flg_Inproc/1  "VNMM_CSB_flg"
  VNMM_CSB_flg_Inproc/1 -> UnitConverter612/1
  UnitConverter612/1 -> VOUTP_CSB_flg/1  "VOUTP_CSB_flg"
  VNMM_ErrorState_enum/1 -> VNMM_ErrorState_enum_Inproc/1  "VNMM_ErrorState_enum"
  VNMM_ErrorState_enum_Inproc/1 -> UnitConverter613/1
  UnitConverter613/1 -> VOUTP_ErrorState_enum/1  "VOUTP_ErrorState_enum"
  VNMM_NodeID_enum/1 -> VNMM_NodeID_enum_Inproc/1  "VNMM_NodeID_enum"
  VNMM_NodeID_enum_Inproc/1 -> UnitConverter614/1
  UnitConverter614/1 -> VOUTP_NodeID_enum/1  "VOUTP_NodeID_enum"
  VNMM_PNI_flg/1 -> VNMM_PNI_flg_Inproc/1  "VNMM_PNI_flg"
  VNMM_PNI_flg_Inproc/1 -> UnitConverter615/1
  UnitConverter615/1 -> VOUTP_PNI_flg/1  "VOUTP_PNI_flg"
  VNMM_RptMsgReq_flg/1 -> VNMM_RptMsgReq_flg_Inproc/1  "VNMM_RptMsgReq_flg"
  VNMM_RptMsgReq_flg_Inproc/1 -> UnitConverter616/1
  UnitConverter616/1 -> VOUTP_RptMsgReq_flg/1  "VOUTP_RptMsgReq_flg"
  VNMM_WakeUp_enum/1 -> VNMM_WakeUp_enum_Inproc/1  "VNMM_WakeUp_enum"
  VNMM_WakeUp_enum_Inproc/1 -> UnitConverter617/1
  UnitConverter617/1 -> VOUTP_WakeUp_enum/1  "VOUTP_WakeUp_enum"
  VNMM_ActiveWU_flg/1 -> VNMM_ActiveWU_flg_Inproc/1  "VNMM_ActiveWU_flg"
  VNMM_ActiveWU_flg_Inproc/1 -> UnitConverter618/1
  UnitConverter618/1 -> VOUTP_ActiveWU_flg/1  "VOUTP_ActiveWU_flg"
  VNMM_SysNMmSta_enum/1 -> VNMM_SysNMmSta_enum_Inproc/1  "VNMM_SysNMmSta_enum"
  VNMM_SysNMmSta_enum_Inproc/1 -> UnitConverter619/1
  UnitConverter619/1 -> VOUTP_SysNMmSta_enum/1  "VOUTP_SysNMmSta_enum"
  VNMM_NetworkReq_flg/1 -> VNMM_NetworkReq_flg_Inproc/1  "VNMM_NetworkReq_flg"
  VNMM_NetworkReq_flg_Inproc/1 -> UnitConverter620/1
  UnitConverter620/1 -> VOUTP_NetworkReq_flg/1  "VOUTP_NetworkReq_flg"
  VPMM_PowerUpState_enum/1 -> VPMM_PowerUpState_enum_Inproc/1  "VPMM_PowerUpState_enum"
  VPMM_PowerUpState_enum_Inproc/1 -> UnitConverter621/1
  UnitConverter621/1 -> VOUTP_PowerUpState_enum/1  "VOUTP_PowerUpState_enum"
  VPMM_PowerDownState_enum/1 -> VPMM_PowerDownState_enum_Inproc/1  "VPMM_PowerDownState_enum"
  VPMM_PowerDownState_enum_Inproc/1 -> UnitConverter622/1
  UnitConverter622/1 -> VOUTP_PowerDownState_enum/1  "VOUTP_PowerDownState_enum"
  VPMM_PowerUpFault_enum/1 -> VPMM_PowerUpFault_enum_Inproc/1  "VPMM_PowerUpFault_enum"
  VPMM_PowerUpFault_enum_Inproc/1 -> UnitConverter623/1
  UnitConverter623/1 -> VOUTP_PowerUpFault_enum/1  "VOUTP_PowerUpFault_enum"
  VPMM_PowerDownFault_enum/1 -> VPMM_PowerDownFault_enum_Inproc/1  "VPMM_PowerDownFault_enum"
  VPMM_PowerDownFault_enum_Inproc/1 -> UnitConverter624/1
  UnitConverter624/1 -> VOUTP_PowerDownFault_enum/1  "VOUTP_PowerDownFault_enum"
  VPMM_ActiveDischargeReq_flg/1 -> VPMM_ActiveDischargeReq_flg_Inproc/1  "VPMM_ActiveDischargeReq_flg"
  VPMM_ActiveDischargeReq_flg_Inproc/1 -> UnitConverter625/1
  UnitConverter625/1 -> VOUTP_ActiveDischargeReq_flg/1  "VOUTP_ActiveDischargeReq_flg"
  VPMM_DCDCEnaReq_flg/1 -> VPMM_DCDCEnaReq_flg_Inproc/1  "VPMM_DCDCEnaReq_flg"
  VPMM_DCDCEnaReq_flg_Inproc/1 -> UnitConverter626/1
  UnitConverter626/1 -> VOUTP_DCDCEnaReq_flg/1  "VOUTP_DCDCEnaReq_flg"
  VPMM_DCDCVoltSetpoint_V/1 -> VPMM_DCDCVoltSetpoint_V_Inproc/1  "VPMM_DCDCVoltSetpoint_V"
  VPMM_DCDCVoltSetpoint_V_Inproc/1 -> UnitConverter627/1
  UnitConverter627/1 -> VOUTP_DCDCVoltSetpoint_V/1  "VOUTP_DCDCVoltSetpoint_V"
  VPMM_HVBatCnctReq_flg/1 -> VPMM_HVBatCnctReq_flg_Inproc/1  "VPMM_HVBatCnctReq_flg"
  VPMM_HVBatCnctReq_flg_Inproc/1 -> UnitConverter628/1
  UnitConverter628/1 -> VOUTP_HVBatCnctReq_flg/1  "VOUTP_HVBatCnctReq_flg"
  VPMM_HVSysReadyToCharge_enum/1 -> VPMM_HVSysReadyToCharge_enum_Inproc/1  "VPMM_HVSysReadyToCharge_enum"
  VPMM_HVSysReadyToCharge_enum_Inproc/1 -> UnitConverter629/1
  UnitConverter629/1 -> VOUTP_HVSysReadyToCharge_enum/1  "VOUTP_HVSysReadyToCharge_enum"
  VPMM_PowerSta_enum/1 -> VPMM_PowerSta_enum_Inproc/1  "VPMM_PowerSta_enum"
  VPMM_PowerSta_enum_Inproc/1 -> UnitConverter630/1
  UnitConverter630/1 -> VOUTP_PowerSta_enum/1  "VOUTP_PowerSta_enum"
  VPMM_LVPwrSta_flg/1 -> VPMM_LVPwrSta_flg_Inproc/1  "VPMM_LVPwrSta_flg"
  VPMM_LVPwrSta_flg_Inproc/1 -> UnitConverter631/1
  UnitConverter631/1 -> VOUTP_LVPwrSta_flg/1  "VOUTP_LVPwrSta_flg"
  VPMM_HVPwrSta_flg/1 -> VPMM_HVPwrSta_flg_Inproc/1  "VPMM_HVPwrSta_flg"
  VPMM_HVPwrSta_flg_Inproc/1 -> UnitConverter632/1
  UnitConverter632/1 -> VOUTP_HVPwrSta_flg/1  "VOUTP_HVPwrSta_flg"
  VPMM_SysPowerMode_enum/1 -> VPMM_SysPowerMode_enum_Inproc/1  "VPMM_SysPowerMode_enum"
  VPMM_SysPowerMode_enum_Inproc/1 -> UnitConverter633/1
  UnitConverter633/1 -> VOUTP_SysPowerMode_enum/1  "VOUTP_SysPowerMode_enum"
  VPMM_FrMCUEnaReq_flg/1 -> VPMM_FrMCUEnaReq_flg_Inproc/1  "VPMM_FrMCUEnaReq_flg"
  VPMM_FrMCUEnaReq_flg_Inproc/1 -> UnitConverter634/1
  UnitConverter634/1 -> VOUTP_FrMCUEnaReq_flg/1  "VOUTP_FrMCUEnaReq_flg"
  VPMM_RrMCUEnaReq_flg/1 -> VPMM_RrMCUEnaReq_flg_Inproc/1  "VPMM_RrMCUEnaReq_flg"
  VPMM_RrMCUEnaReq_flg_Inproc/1 -> UnitConverter635/1
  UnitConverter635/1 -> VOUTP_RrMCUEnaReq_flg/1  "VOUTP_RrMCUEnaReq_flg"
  VPMM_DrivetrainSelect_enum/1 -> VPMM_DrivetrainSelect_enum_Inproc/1  "VPMM_DrivetrainSelect_enum"
  VPMM_DrivetrainSelect_enum_Inproc/1 -> UnitConverter636/1
  UnitConverter636/1 -> VOUTP_DrivetrainSelect_enum/1  "VOUTP_DrivetrainSelect_enum"
  VPMM_DrSeatSta_enum/1 -> VPMM_DrSeatSta_enum_Inproc/1  "VPMM_DrSeatSta_enum"
  VPMM_DrSeatSta_enum_Inproc/1 -> UnitConverter637/1
  UnitConverter637/1 -> VOUTP_DrSeatSta_enum/1  "VOUTP_DrSeatSta_enum"
  VPMM_PwrStaSelect_enum/1 -> VPMM_PwrStaSelect_enum_Inproc/1  "VPMM_PwrStaSelect_enum"
  VPMM_PwrStaSelect_enum_Inproc/1 -> UnitConverter638/1
  UnitConverter638/1 -> VOUTP_PwrStaSelect_enum/1  "VOUTP_PwrStaSelect_enum"
  VPMM_PwrStaConstraint_enum/1 -> VPMM_PwrStaConstraint_enum_Inproc/1  "VPMM_PwrStaConstraint_enum"
  VPMM_PwrStaConstraint_enum_Inproc/1 -> UnitConverter639/1
  UnitConverter639/1 -> VOUTP_PwrStaConstraint_enum/1  "VOUTP_PwrStaConstraint_enum"
  VPMM_TCountSta_enum/1 -> VPMM_TCountSta_enum_Inproc/1  "VPMM_TCountSta_enum"
  VPMM_TCountSta_enum_Inproc/1 -> UnitConverter640/1
  UnitConverter640/1 -> VOUTP_TCountSta_enum/1  "VOUTP_TCountSta_enum"
  VPMM_PwrUpReq_enum/1 -> VPMM_PwrUpReq_enum_Inproc/1  "VPMM_PwrUpReq_enum"
  VPMM_PwrUpReq_enum_Inproc/1 -> UnitConverter641/1
  UnitConverter641/1 -> VOUTP_PwrUpReq_enum/1  "VOUTP_PwrUpReq_enum"
  VPMM_PwrDownReq_enum/1 -> VPMM_PwrDownReq_enum_Inproc/1  "VPMM_PwrDownReq_enum"
  VPMM_PwrDownReq_enum_Inproc/1 -> UnitConverter642/1
  UnitConverter642/1 -> VOUTP_PwrDownReq_enum/1  "VOUTP_PwrDownReq_enum"
  VPMM_LowSOCWarn_enum/1 -> VPMM_LowSOCWarn_enum_Inproc/1  "VPMM_LowSOCWarn_enum"
  VPMM_LowSOCWarn_enum_Inproc/1 -> UnitConverter643/1
  UnitConverter643/1 -> VOUTP_LowSOCWarn_enum/1  "VOUTP_LowSOCWarn_enum"
  VPMM_ReVehThdChkSta_enum/1 -> VPMM_ReVehThdChkSta_enum_Inproc/1  "VPMM_ReVehThdChkSta_enum"
  VPMM_ReVehThdChkSta_enum_Inproc/1 -> UnitConverter644/1
  UnitConverter644/1 -> VOUTP_ReVehThdChkSta_enum/1  "VOUTP_ReVehThdChkSta_enum"
  VPMM_EvccAplusPwrUpReq_flg/1 -> VPMM_EvccAplusPwrUpReq_flg_Inproc/1  "VPMM_EvccAplusPwrUpReq_flg"
  VPMM_EvccAplusPwrUpReq_flg_Inproc/1 -> UnitConverter645/1
  UnitConverter645/1 -> VOUTP_EvccAplusPwrUpReq_flg/1  "VOUTP_EvccAplusPwrUpReq_flg"
  VPMM_PwrStaONTOPopReq_flg/1 -> VPMM_PwrStaONTOPopReq_flg_Inproc/1  "VPMM_PwrStaONTOPopReq_flg"
  VPMM_PwrStaONTOPopReq_flg_Inproc/1 -> UnitConverter646/1
  UnitConverter646/1 -> VOUTP_PwrStaONTOPopReq_flg/1  "VOUTP_PwrStaONTOPopReq_flg"
  VPMM_IVIPwrStaONTOPopT_s/1 -> VPMM_IVIPwrStaONTOPopT_s_Inproc/1  "VPMM_IVIPwrStaONTOPopT_s"
  VPMM_IVIPwrStaONTOPopT_s_Inproc/1 -> UnitConverter647/1
  UnitConverter647/1 -> VOUTP_IVIPwrStaONTOPopT_s/1  "VOUTP_IVIPwrStaONTOPopT_s"
  VPMM_LVChrgHoldTtimer_s/1 -> VPMM_LVChrgHoldTtimer_s_Inproc/1  "VPMM_LVChrgHoldTtimer_s"
  VPMM_LVChrgHoldTtimer_s_Inproc/1 -> UnitConverter648/1
  UnitConverter648/1 -> VOUTP_LVChrgHoldTtimer_s/1  "VOUTP_LVChrgHoldTtimer_s"
  VPMM_LVBattChrgTimeCnt_s/1 -> VPMM_LVBattChrgTimeCnt_s_Inproc/1  "VPMM_LVBattChrgTimeCnt_s"
  VPMM_LVBattChrgTimeCnt_s_Inproc/1 -> UnitConverter649/1
  UnitConverter649/1 -> VOUTP_LVBattChrgTimeCnt_s/1  "VOUTP_LVBattChrgTimeCnt_s"
  VPMM_SilentChkAllowSleep_flg/1 -> VPMM_SilentChkAllowSleep_flg_Inproc/1  "VPMM_SilentChkAllowSleep_flg"
  VPMM_SilentChkAllowSleep_flg_Inproc/1 -> UnitConverter650/1
  UnitConverter650/1 -> VOUTP_SilentChkAllowSleep_flg/1  "VOUTP_SilentChkAllowSleep_flg"
  VPMM_TimerAllowSleep_flg/1 -> VPMM_TimerAllowSleep_flg_Inproc/1  "VPMM_TimerAllowSleep_flg"
  VPMM_TimerAllowSleep_flg_Inproc/1 -> UnitConverter651/1
  UnitConverter651/1 -> VOUTP_TimerAllowSleep_flg/1  "VOUTP_TimerAllowSleep_flg"
  VPMM_FDADC12VDetAvg_mV/1 -> VPMM_FDADC12VDetAvg_mV_Inproc/1  "VPMM_FDADC12VDetAvg_mV"
  VPMM_FDADC12VDetAvg_mV_Inproc/1 -> UnitConverter652/1
  UnitConverter652/1 -> VOUTP_FDADC12VDetAvg_mV/1  "VOUTP_FDADC12VDetAvg_mV"
  VPMM_PMMAllowECUSleep_flg/1 -> VPMM_PMMAllowECUSleep_flg_Inproc/1  "VPMM_PMMAllowECUSleep_flg"
  VPMM_PMMAllowECUSleep_flg_Inproc/1 -> UnitConverter653/1
  UnitConverter653/1 -> VOUTP_PMMAllowECUSleep_flg/1  "VOUTP_PMMAllowECUSleep_flg"
  VPMM_LVSilentChrgSta_enum/1 -> VPMM_LVSilentChrgSta_enum_Inproc/1  "VPMM_LVSilentChrgSta_enum"
  VPMM_LVSilentChrgSta_enum_Inproc/1 -> UnitConverter654/1
  UnitConverter654/1 -> VOUTP_LVSilentChrgSta_enum/1  "VOUTP_LVSilentChrgSta_enum"
  VPMM_LVSilentChrgReq_flg/1 -> VPMM_LVSilentChrgReq_flg_Inproc/1  "VPMM_LVSilentChrgReq_flg"
  VPMM_LVSilentChrgReq_flg_Inproc/1 -> UnitConverter655/1
  UnitConverter655/1 -> VOUTP_LVSilentChrgReq_flg/1  "VOUTP_LVSilentChrgReq_flg"
  VPMM_LVSilentChrgLv_enum/1 -> VPMM_LVSilentChrgLv_enum_Inproc/1  "VPMM_LVSilentChrgLv_enum"
  VPMM_LVSilentChrgLv_enum_Inproc/1 -> UnitConverter656/1
  UnitConverter656/1 -> VOUTP_LVSilentChrgLv_enum/1  "VOUTP_LVSilentChrgLv_enum"
  VPMM_CtrlFrPwrStbA1P_flg/1 -> VPMM_CtrlFrPwrStbA1P_flg_Inproc/1  "VPMM_CtrlFrPwrStbA1P_flg"
  VPMM_CtrlFrPwrStbA1P_flg_Inproc/1 -> UnitConverter657/1
  UnitConverter657/1 -> VOUTP_CtrlFrPwrStbA1P_flg/1  "VOUTP_CtrlFrPwrStbA1P_flg"
  VPMM_CtrlFrRC1_flg/1 -> VPMM_CtrlFrRC1_flg_Inproc/1  "VPMM_CtrlFrRC1_flg"
  VPMM_CtrlFrRC1_flg_Inproc/1 -> UnitConverter658/1
  UnitConverter658/1 -> VOUTP_CtrlFrRC1_flg/1  "VOUTP_CtrlFrRC1_flg"
  VPMM_CtrlFrBMSCCUCIR_flg/1 -> VPMM_CtrlFrBMSCCUCIR_flg_Inproc/1  "VPMM_CtrlFrBMSCCUCIR_flg"
  VPMM_CtrlFrBMSCCUCIR_flg_Inproc/1 -> UnitConverter659/1
  UnitConverter659/1 -> VOUTP_CtrlFrBMSCCUCIR_flg/1  "VOUTP_CtrlFrBMSCCUCIR_flg"
  VPMM_CtrlFrEDUINVERTER_flg/1 -> VPMM_CtrlFrEDUINVERTER_flg_Inproc/1  "VPMM_CtrlFrEDUINVERTER_flg"
  VPMM_CtrlFrEDUINVERTER_flg_Inproc/1 -> UnitConverter660/1
  UnitConverter660/1 -> VOUTP_CtrlFrEDUINVERTER_flg/1  "VOUTP_CtrlFrEDUINVERTER_flg"
  VPMM_HWResetSta_enum/1 -> VPMM_HWResetSta_enum_Inproc/1  "VPMM_HWResetSta_enum"
  VPMM_HWResetSta_enum_Inproc/1 -> UnitConverter661/1
  UnitConverter661/1 -> VOUTP_HWResetSta_enum/1  "VOUTP_HWResetSta_enum"
  VPMM_CtrlDrPwrStbA2_flg/1 -> VPMM_CtrlDrPwrStbA2_flg_Inproc/1  "VPMM_CtrlDrPwrStbA2_flg"
  VPMM_CtrlDrPwrStbA2_flg_Inproc/1 -> UnitConverter662/1
  UnitConverter662/1 -> VOUTP_CtrlDrPwrStbA2_flg/1  "VOUTP_CtrlDrPwrStbA2_flg"
  VPMM_PwrStaTOSta_enum/1 -> VPMM_PwrStaTOSta_enum_Inproc/1  "VPMM_PwrStaTOSta_enum"
  VPMM_PwrStaTOSta_enum_Inproc/1 -> UnitConverter663/1
  UnitConverter663/1 -> VOUTP_PwrStaTOSta_enum/1  "VOUTP_PwrStaTOSta_enum"
  VPMM_Sched_ChgTOSta_enum/1 -> VPMM_Sched_ChgTOSta_enum_Inproc/1  "VPMM_Sched_ChgTOSta_enum"
  VPMM_Sched_ChgTOSta_enum_Inproc/1 -> UnitConverter664/1
  UnitConverter664/1 -> VOUTP_Sched_ChgTOSta_enum/1  "VOUTP_Sched_ChgTOSta_enum"
  VPMM_PwrReq_OTA_enum/1 -> VPMM_PwrReq_OTA_enum_Inproc/1  "VPMM_PwrReq_OTA_enum"
  VPMM_PwrReq_OTA_enum_Inproc/1 -> UnitConverter665/1
  UnitConverter665/1 -> VOUTP_PwrReq_OTA_enum/1  "VOUTP_PwrReq_OTA_enum"
  VPMM_OTAPwrReqOFFChkSta_enum/1 -> VPMM_OTAPwrReqOFFChkSta_enum_Inproc/1  "VPMM_OTAPwrReqOFFChkSta_enum"
  VPMM_OTAPwrReqOFFChkSta_enum_Inproc/1 -> UnitConverter666/1
  UnitConverter666/1 -> VOUTP_OTAPwrReqOFFChkSta_enum/1  "VOUTP_OTAPwrReqOFFChkSta_enum"
  VPMM_OTAPwrReqStdChkSta_enum/1 -> VPMM_OTAPwrReqStdChkSta_enum_Inproc/1  "VPMM_OTAPwrReqStdChkSta_enum"
  VPMM_OTAPwrReqStdChkSta_enum_Inproc/1 -> UnitConverter667/1
  UnitConverter667/1 -> VOUTP_OTAPwrReqStdChkSta_enum/1  "VOUTP_OTAPwrReqStdChkSta_enum"
  VPMM_PwrReqRAPSAvail_flg/1 -> VPMM_PwrReqRAPSAvail_flg_Inproc/1  "VPMM_PwrReqRAPSAvail_flg"
  VPMM_PwrReqRAPSAvail_flg_Inproc/1 -> UnitConverter668/1
  UnitConverter668/1 -> VOUTP_PwrReqRAPSAvail_flg/1  "VOUTP_PwrReqRAPSAvail_flg"
  VSYS_HWVer1_cnt/1 -> VSYS_HWVer1_cnt_Inproc/1  "VSYS_HWVer1_cnt"
  VSYS_HWVer1_cnt_Inproc/1 -> UnitConverter669/1
  UnitConverter669/1 -> VOUTP_HWVer1_cnt/1  "VOUTP_HWVer1_cnt"
  VSYS_HWVer2_cnt/1 -> VSYS_HWVer2_cnt_Inproc/1  "VSYS_HWVer2_cnt"
  VSYS_HWVer2_cnt_Inproc/1 -> UnitConverter670/1
  UnitConverter670/1 -> VOUTP_HWVer2_cnt/1  "VOUTP_HWVer2_cnt"
  VSYS_HWVer3_cnt/1 -> VSYS_HWVer3_cnt_Inproc/1  "VSYS_HWVer3_cnt"
  VSYS_HWVer3_cnt_Inproc/1 -> UnitConverter671/1
  UnitConverter671/1 -> VOUTP_HWVer3_cnt/1  "VOUTP_HWVer3_cnt"
  VSYS_CarModel1_cnt/1 -> VSYS_CarModel1_cnt_Inproc/1  "VSYS_CarModel1_cnt"
  VSYS_CarModel1_cnt_Inproc/1 -> UnitConverter672/1
  UnitConverter672/1 -> VOUTP_CarModel1_cnt/1  "VOUTP_CarModel1_cnt"
  VSYS_CarModel2_cnt/1 -> VSYS_CarModel2_cnt_Inproc/1  "VSYS_CarModel2_cnt"
  VSYS_CarModel2_cnt_Inproc/1 -> UnitConverter673/1
  UnitConverter673/1 -> VOUTP_CarModel2_cnt/1  "VOUTP_CarModel2_cnt"
  VSYS_CarModel3_cnt/1 -> VSYS_CarModel3_cnt_Inproc/1  "VSYS_CarModel3_cnt"
  VSYS_CarModel3_cnt_Inproc/1 -> UnitConverter674/1
  UnitConverter674/1 -> VOUTP_CarModel3_cnt/1  "VOUTP_CarModel3_cnt"
  VSYS_ECU1_cnt/1 -> VSYS_ECU1_cnt_Inproc/1  "VSYS_ECU1_cnt"
  VSYS_ECU1_cnt_Inproc/1 -> UnitConverter675/1
  UnitConverter675/1 -> VOUTP_ECU1_cnt/1  "VOUTP_ECU1_cnt"
  VSYS_ECU2_cnt/1 -> VSYS_ECU2_cnt_Inproc/1  "VSYS_ECU2_cnt"
  VSYS_ECU2_cnt_Inproc/1 -> UnitConverter676/1
  UnitConverter676/1 -> VOUTP_ECU2_cnt/1  "VOUTP_ECU2_cnt"
  VSYS_Major1_cnt/1 -> VSYS_Major1_cnt_Inproc/1  "VSYS_Major1_cnt"
  VSYS_Major1_cnt_Inproc/1 -> UnitConverter677/1
  UnitConverter677/1 -> VOUTP_Major1_cnt/1  "VOUTP_Major1_cnt"
  VSYS_Major2_cnt/1 -> VSYS_Major2_cnt_Inproc/1  "VSYS_Major2_cnt"
  VSYS_Major2_cnt_Inproc/1 -> UnitConverter678/1
  UnitConverter678/1 -> VOUTP_Major2_cnt/1  "VOUTP_Major2_cnt"
  VSYS_Minor1_cnt/1 -> VSYS_Minor1_cnt_Inproc/1  "VSYS_Minor1_cnt"
  VSYS_Minor1_cnt_Inproc/1 -> UnitConverter679/1
  UnitConverter679/1 -> VOUTP_Minor1_cnt/1  "VOUTP_Minor1_cnt"
  VSYS_Minor2_cnt/1 -> VSYS_Minor2_cnt_Inproc/1  "VSYS_Minor2_cnt"
  VSYS_Minor2_cnt_Inproc/1 -> UnitConverter680/1
  UnitConverter680/1 -> VOUTP_Minor2_cnt/1  "VOUTP_Minor2_cnt"
  VSYS_Patch1_cnt/1 -> VSYS_Patch1_cnt_Inproc/1  "VSYS_Patch1_cnt"
  VSYS_Patch1_cnt_Inproc/1 -> UnitConverter681/1
  UnitConverter681/1 -> VOUTP_Patch1_cnt/1  "VOUTP_Patch1_cnt"
  VSYS_Patch2_cnt/1 -> VSYS_Patch2_cnt_Inproc/1  "VSYS_Patch2_cnt"
  VSYS_Patch2_cnt_Inproc/1 -> UnitConverter682/1
  UnitConverter682/1 -> VOUTP_Patch2_cnt/1  "VOUTP_Patch2_cnt"
  VSYS_Country1_cnt/1 -> VSYS_Country1_cnt_Inproc/1  "VSYS_Country1_cnt"
  VSYS_Country1_cnt_Inproc/1 -> UnitConverter683/1
  UnitConverter683/1 -> VOUTP_Country1_cnt/1  "VOUTP_Country1_cnt"
  VSYS_Country2_cnt/1 -> VSYS_Country2_cnt_Inproc/1  "VSYS_Country2_cnt"
  VSYS_Country2_cnt_Inproc/1 -> UnitConverter684/1
  UnitConverter684/1 -> VOUTP_Country2_cnt/1  "VOUTP_Country2_cnt"
  VSYS_Variation_cnt/1 -> VSYS_Variation_cnt_Inproc/1  "VSYS_Variation_cnt"
  VSYS_Variation_cnt_Inproc/1 -> UnitConverter685/1
  UnitConverter685/1 -> VOUTP_Variation_cnt/1  "VOUTP_Variation_cnt"
  VSYS_Dash1_cnt/1 -> VSYS_Dash1_cnt_Inproc/1  "VSYS_Dash1_cnt"
  VSYS_Dash1_cnt_Inproc/1 -> UnitConverter686/1
  UnitConverter686/1 -> VOUTP_Dash1_cnt/1  "VOUTP_Dash1_cnt"
  VSYS_Change1_cnt/1 -> VSYS_Change1_cnt_Inproc/1  "VSYS_Change1_cnt"
  VSYS_Change1_cnt_Inproc/1 -> UnitConverter687/1
  UnitConverter687/1 -> VOUTP_Change1_cnt/1  "VOUTP_Change1_cnt"
  VSYS_Change2_cnt/1 -> VSYS_Change2_cnt_Inproc/1  "VSYS_Change2_cnt"
  VSYS_Change2_cnt_Inproc/1 -> UnitConverter688/1
  UnitConverter688/1 -> VOUTP_Change2_cnt/1  "VOUTP_Change2_cnt"
  VSYS_Dash2_cnt/1 -> VSYS_Dash2_cnt_Inproc/1  "VSYS_Dash2_cnt"
  VSYS_Dash2_cnt_Inproc/1 -> UnitConverter689/1
  UnitConverter689/1 -> VOUTP_Dash2_cnt/1  "VOUTP_Dash2_cnt"
  VSYS_SHA1_cnt/1 -> VSYS_SHA1_cnt_Inproc/1  "VSYS_SHA1_cnt"
  VSYS_SHA1_cnt_Inproc/1 -> UnitConverter690/1
  UnitConverter690/1 -> VOUTP_SHA1_cnt/1  "VOUTP_SHA1_cnt"
  VSYS_SHA2_cnt/1 -> VSYS_SHA2_cnt_Inproc/1  "VSYS_SHA2_cnt"
  VSYS_SHA2_cnt_Inproc/1 -> UnitConverter691/1
  UnitConverter691/1 -> VOUTP_SHA2_cnt/1  "VOUTP_SHA2_cnt"
  VSYS_SHA3_cnt/1 -> VSYS_SHA3_cnt_Inproc/1  "VSYS_SHA3_cnt"
  VSYS_SHA3_cnt_Inproc/1 -> UnitConverter692/1
  UnitConverter692/1 -> VOUTP_SHA3_cnt/1  "VOUTP_SHA3_cnt"
  VSYS_SHA4_cnt/1 -> VSYS_SHA4_cnt_Inproc/1  "VSYS_SHA4_cnt"
  VSYS_SHA4_cnt_Inproc/1 -> UnitConverter693/1
  UnitConverter693/1 -> VOUTP_SHA4_cnt/1  "VOUTP_SHA4_cnt"
  VSYS_SHA5_cnt/1 -> VSYS_SHA5_cnt_Inproc/1  "VSYS_SHA5_cnt"
  VSYS_SHA5_cnt_Inproc/1 -> UnitConverter694/1
  UnitConverter694/1 -> VOUTP_SHA5_cnt/1  "VOUTP_SHA5_cnt"
  VSYS_SHA6_cnt/1 -> VSYS_SHA6_cnt_Inproc/1  "VSYS_SHA6_cnt"
  VSYS_SHA6_cnt_Inproc/1 -> UnitConverter695/1
  UnitConverter695/1 -> VOUTP_SHA6_cnt/1  "VOUTP_SHA6_cnt"
  VSYS_SHA7_cnt/1 -> VSYS_SHA7_cnt_Inproc/1  "VSYS_SHA7_cnt"
  VSYS_SHA7_cnt_Inproc/1 -> UnitConverter696/1
  UnitConverter696/1 -> VOUTP_SHA7_cnt/1  "VOUTP_SHA7_cnt"
  VSYS_SHA8_cnt/1 -> VSYS_SHA8_cnt_Inproc/1  "VSYS_SHA8_cnt"
  VSYS_SHA8_cnt_Inproc/1 -> UnitConverter697/1
  UnitConverter697/1 -> VOUTP_SHA8_cnt/1  "VOUTP_SHA8_cnt"
  VSYS_NvWriteReqRisingEdge_flg/1 -> VSYS_NvWriteReqRisingEdge_flg_Inproc/1  "VSYS_NvWriteReqRisingEdge_flg"
  VSYS_NvWriteReqRisingEdge_flg_Inproc/1 -> UnitConverter698/1
  UnitConverter698/1 -> VOUTP_NvWriteReqRisingEdge_flg/1  "VOUTP_NvWriteReqRisingEdge_flg"
  VSYS_FdcSlpReqRisingEdge_flg/1 -> VSYS_FdcSlpReqRisingEdge_flg_Inproc/1  "VSYS_FdcSlpReqRisingEdge_flg"
  VSYS_FdcSlpReqRisingEdge_flg_Inproc/1 -> UnitConverter699/1
  UnitConverter699/1 -> VOUTP_FdcSlpReqRisingEdge_flg/1  "VOUTP_FdcSlpReqRisingEdge_flg"
  VSYS_FdcSlpTime_sec/1 -> VSYS_FdcSlpTime_sec_Inproc/1  "VSYS_FdcSlpTime_sec"
  VSYS_FdcSlpTime_sec_Inproc/1 -> UnitConverter700/1
  UnitConverter700/1 -> VOUTP_FdcSlpTime_sec/1  "VOUTP_FdcSlpTime_sec"
  VSYS_PmicBootReason_enum/1 -> VSYS_PmicBootReason_enum_Inproc/1  "VSYS_PmicBootReason_enum"
  VSYS_PmicBootReason_enum_Inproc/1 -> UnitConverter701/1
  UnitConverter701/1 -> VOUTP_PmicBootReason_enum/1  "VOUTP_PmicBootReason_enum"
  VSYS_WisrBootReason_raw32/1 -> VSYS_WisrBootReason_raw32_Inproc/1  "VSYS_WisrBootReason_raw32"
  VSYS_WisrBootReason_raw32_Inproc/1 -> UnitConverter702/1
  UnitConverter702/1 -> VOUTP_WisrBootReason_raw32/1  "VOUTP_WisrBootReason_raw32"
  VSYS_AcoreRebootCmdACK_flg/1 -> VSYS_AcoreRebootCmdACK_flg_Inproc/1  "VSYS_AcoreRebootCmdACK_flg"
  VSYS_AcoreRebootCmdACK_flg_Inproc/1 -> UnitConverter703/1
  UnitConverter703/1 -> VOUTP_AcoreRebootCmdACK_flg/1  "VOUTP_AcoreRebootCmdACK_flg"
  VSYS_CurrentNmState_enum/1 -> VSYS_CurrentNmState_enum_Inproc/1  "VSYS_CurrentNmState_enum"
  VSYS_CurrentNmState_enum_Inproc/1 -> UnitConverter704/1
  UnitConverter704/1 -> VOUTP_CurrentNmState_enum/1  "VOUTP_CurrentNmState_enum"
  VSYS_ECUGen1_cnt/1 -> VSYS_ECUGen1_cnt_Inproc/1  "VSYS_ECUGen1_cnt"
  VSYS_ECUGen1_cnt_Inproc/1 -> UnitConverter705/1
  UnitConverter705/1 -> VOUTP_ECUGen1_cnt/1  "VOUTP_ECUGen1_cnt"
  VSYS_ECUGen2_cnt/1 -> VSYS_ECUGen2_cnt_Inproc/1  "VSYS_ECUGen2_cnt"
  VSYS_ECUGen2_cnt_Inproc/1 -> UnitConverter706/1
  UnitConverter706/1 -> VOUTP_ECUGen2_cnt/1  "VOUTP_ECUGen2_cnt"
  VSYS_PmicBootPath_raw32/1 -> VSYS_PmicBootPath_raw32_Inproc/1  "VSYS_PmicBootPath_raw32"
